simulink model "Intergration_simu"  (R2018b)
settings: Solver=FixedStepDiscrete  StartTime=0.0  StopTime=14  FixedStep=0.005  RelTol=1e-3
PostLoadFcn:
  | if any(exist('dsrtsu_mdlpostloadfcn', 'file') ~= 0), dsrtsu_mdlpostloadfcn('Execute', bdroot); end
values from neighbouring files (symbols this model uses):
  P_x165_On = 1.0    [CAN_Tx.sldd]
  P_x242_On = 1.0    [CAN_Tx.sldd]
  P_x246_On = 1.0    [CAN_Tx.sldd]
libraries: rtican x112, simulink x59
(part 2 of 31)

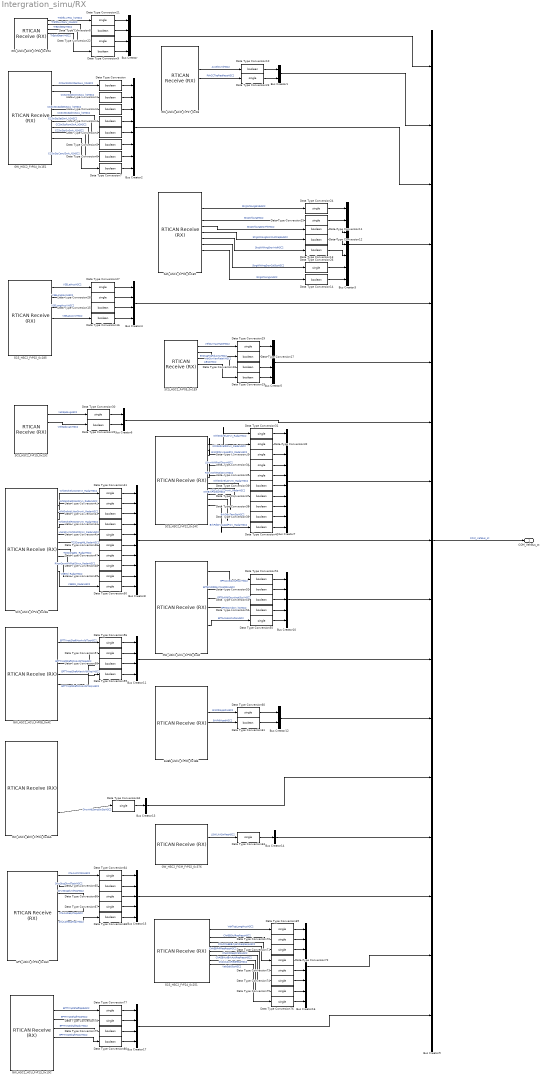
== system Intergration_simu/RX ==
  Bus Creator : BusCreator  Inputs=4  OutDataTypeStr=Bus: x194  NonVirtualBus=on
      settings: InheritFromInputs=off
  Bus Creator1 : BusCreator  Inputs=2  OutDataTypeStr=Bus: xFB  NonVirtualBus=on
      settings: InheritFromInputs=off
  Bus Creator10 : BusCreator  Inputs=5  OutDataTypeStr=Bus: xAF  NonVirtualBus=on
      settings: InheritFromInputs=off
  Bus Creator11 : BusCreator  Inputs=4  OutDataTypeStr=Bus: xAC  NonVirtualBus=on
      settings: InheritFromInputs=off
  Bus Creator12 : BusCreator  Inputs=2  OutDataTypeStr=Bus: x1B6  NonVirtualBus=on
      settings: InheritFromInputs=off
  Bus Creator13 : BusCreator  Inputs=1  OutDataTypeStr=Bus: x46A  NonVirtualBus=on
      settings: InheritFromInputs=off
  Bus Creator14 : BusCreator  Inputs=1  OutDataTypeStr=Bus: x376  NonVirtualBus=on
      settings: InheritFromInputs=off
  Bus Creator15 : BusCreator  Inputs=5  OutDataTypeStr=Bus: x1EC  NonVirtualBus=on
      settings: InheritFromInputs=off
  Bus Creator16 : BusCreator  Inputs=8  OutDataTypeStr=Bus: x251  NonVirtualBus=on
      settings: InheritFromInputs=off
  Bus Creator17 : BusCreator  Inputs=4  OutDataTypeStr=Bus: x19C  NonVirtualBus=on
      settings: InheritFromInputs=off
  Bus Creator2 : BusCreator  Inputs=8  OutDataTypeStr=Bus: x1E1  NonVirtualBus=on
      settings: InheritFromInputs=off
  Bus Creator3 : BusCreator  Inputs=7  OutDataTypeStr=Bus: x1E5  NonVirtualBus=on
      settings: InheritFromInputs=off
  Bus Creator4 : BusCreator  Inputs=4  OutDataTypeStr=Bus: x185  NonVirtualBus=on
      settings: InheritFromInputs=off
  Bus Creator5 : BusCreator  Inputs=4  OutDataTypeStr=Bus: x1E9  NonVirtualBus=on
      settings: InheritFromInputs=off
  Bus Creator6 : BusCreator  Inputs=2  OutDataTypeStr=Bus: x23C  NonVirtualBus=on
      settings: InheritFromInputs=off
  Bus Creator7 : BusCreator  Inputs=10  OutDataTypeStr=Bus: x24C  NonVirtualBus=on
      settings: InheritFromInputs=off
  Bus Creator8 : BusCreator  Inputs=10  OutDataTypeStr=Bus: x24E  NonVirtualBus=on
      settings: InheritFromInputs=off
  Bus Creator9 : BusCreator  Inputs=17  OutDataTypeStr=Bus: COM_VEHBUS_ST  NonVirtualBus=on
      settings: InheritFromInputs=off
  Data Type Conversion{,1..20,36..40,43..44,51..54,58..59,61,65,68,79..80} (39 alike) : DataTypeConversion  OutDataTypeStr=boolean
  Data Type Conversion{21..35,41..42,45..50,55..57,60,62..64,66..67,69..78} (42 alike) : DataTypeConversion  OutDataTypeStr=single
  EHBS_HSC2_FrP00_0x1B6 : rtican/RTICAN Receive (RX)   Reserved1=[]  Reserved2=[]  Reserved3=[]  Reserved4=[]  SfcnMessage=[]  Msg_Struct=[]  BoardTypeNo=[]  BoardNo=[]  ChannelNo=[]  Parameters=[]  DialogFcn=[]  UnitName=[]  Revision=[]  UnitValues=[]  DSProperties=struct('RTI',struct('Version',uint32(5),'BlockType',struct('isSLSource',uint8(1),'isSLSink',uint8(1),'isHWSource',uint8(0),'isHWSink',uint8(0),'isSetup',uint8(0),'isInline',uint8(1),'isNonInline',uint8(0),'isInterrupt',uint8(0),'isChannelwise',uint8(0)),'IOBoardType','RTICAN','UnitType','MESSAGE','Identifier','RX','DialogType','MSVC','BlockSet','RTICAN','SlaveProcessor','CAN'))  RTIBlockInterface=struct('OutputPortsWidth',int32([1 1 1 1 1 1 1]),'OutputPortsActive',[1 1 1 1 1 1 1],'OutputPortsName',{{'BrkPdlAppdChksmHSC2','BrkPdlAppdRCHSC2','BrkPdlAppdVHSC2','BrkPdlAppdHSC2',['RX status'],['RX time'],['RX delta time']}},'OutputPortsDataType',{{'SS_DOUBLE','SS_DOUBLE','SS_DOUBLE','SS_DOUBLE','SS_DOUBLE','SS_DOUBLE','SS_DOUBLE'}},'OutputPortsLabel',{{'BrkPdlAppdChksmHSC2','BrkPdlAppdRCHSC2','BrkPdlAppdVHSC2','BrkPdlAppdHSC2','','',''}},'OutputPortsLabelMode','ON','InputPortsWidth',int32(0),'InputPortsActive',0,'DialogFcn','rtican_message_interface_gui','BlockDisplay',{{'','center'}},'IconTransparency','on','ParameterTunableNames',{{}},'InitLevel',3,'BlockName',struct('Token',{{'EHBS_HSC2_FrP00'}}),'SampleTime',{{-1}},'TriggerPort',{{'none'}},'EnablePort',{{'none'}})  RTIBlockParameters=struct('BoardTypeNo',{{1,'OFF',[]}},'BoardNo',{{1,'ON',[1 16]}},'ChannelNo',{{1,'ON',[1 2]}},'Parameters',{{struct('DataFileSupport',struct('DataFileSelectedMaster',1,'DataFileSelectedLocal',1,'DataFileName','c:\users\linqi\desktop\matlab\acc\dbc\ep21_dbc\171114-lh1-ep21_ep2_fdr-_v07_acc.dbc|','DataFileDate',['24-11月-2020 15:06:17'],'SelectedFile','..\..\dbc\ep21_dbc\171114-lh1-ep21_ep2_fdr-_v07_acc.dbc','InterfaceFcn','rtican_dbc_file_parser'),'Options',struct('StatusSelected',1,'TimeSelected',1,'DeltaTimeSelected',1,'BytePortSelected',0,'MessageLengthSelected',0,'TriggerPort',struct('Selected',0,'TriggerType',0),'UserCoding',struct('Selected',0,'InterfaceFile','UserDecodingFile','FcnName','UserDecodeFcn','InportSelected',0,'InportWidth',1,'OutportSelected',0,'OutportWidth',1),'EnablePortSelected',0,'SignalOnPortnameSelected',1,'UseRXService',0),'Message',struct('MsgOnBlocknameSelected',1,'MsgName','EHBS_HSC2_FrP00','MsgIdFormat',0,'MsgId',438,'MsgLength',8,'NumSignals',4,'SampleTime',-1,'Signal',struct('SgnName',{'BrkPdlAppdChksmHSC2','BrkPdlAppdRCHSC2','BrkPdlAppdVHSC2','BrkPdlAppdHSC2'},'SgnStartBit',{0,8,48,50},'SgnLength',{8,4,2,1},'ByteLayout',{2,2,2,2},'Factor',{1,1,1,1},'Offset',{0,0,0,0},'SgnComment',{'','','',''},'SgnUnit',{'','','',''},'Min',{0,0,0,0},'Max',{255,15,3,1},'SgnType',{0,0,0,0},'SLDataType',{'SS_DOUBLE','SS_DOUBLE','SS_DOUBLE','SS_DOUBLE'},'DataType',{0,0,0,0},'ModeValue',{-1,-1,-1,-1}),'MsgIdNumFormat',0,'MsgComment',{{''}}),'Version',1.2,'general',struct('isFromLib',0)),'OFF',[]}},'GroupId',{{struct('Group',{{'RTICAN'}},'No',1,'Behavior',{{'NAMECHANGE'}},'BlockType',{{'SINK'}},'NameChangeFlag',0),'OFF',[]}},'SFcnRTICANMessage',{{struct('MsgType','RX','SFcnPortType','Scalar','MsgName','EHBS_HSC2_FrP00','MsgIdFormat','STD','MsgId',438,'MsgLength',8,'NumSignals',4,'SampleTime',-1,'Signal',struct('SgnName',{'BrkPdlAppdChksmHSC2','BrkPdlAppdRCHSC2','BrkPdlAppdVHSC2','BrkPdlAppdHSC2'},'SgnStartBit',{0,8,48,50},'SgnLength',{8,4,2,1},'ByteLayout',{['motorola back.'],['motorola back.'],['motorola back.'],['motorola back.']},'Factor',{1,1,1,1},'Offset',{0,0,0,0},'SgnType',{'standard','standard','standard','standard'},'SLDataType',{'SS_DOUBLE','SS_DOUBLE','SS_DOUBLE','SS_DOUBLE'},'DataType',{['unsigned int'],['unsigned int'],['unsigned int'],['unsigned int']},'ModeValue',{-1,-1,-1,-1}),'StatusSelected','yes','TimeSelected','yes','DeltaTimeSelected','yes','BytePortSelected','no','MessageLengthSelected','no','TriggerPort',struct('Selected','no','TriggerType',0),'UserCoding',struct('Selected','no','InterfaceFile','UserDecodingFile','FcnName','UserDecodeFcn','InportSelected','no','InportWidth',1,'OutportSelected','no','OutportWidth',1),'EnablePortSelected','no','UseRXService','no','BoardType','DS1','BoardNo',1,'ControllerNo',1),'OFF',[]}},'TLCFileName',{{'rtican_rx_message','OFF',[]}})  RTISFcnParameters=struct('SFcnRTICANMessage','struct','TLCFileName','char')  RTIBlockParaDefault=struct('BoardTypeNo',4302,'BoardNo',1,'ChannelNo',1,'Parameters',struct('DataFileSupport',struct('DataFileSelectedMaster',0,'DataFileSelectedLocal',0,'DataFileName','','DataFileDate','','SelectedFile',['<no file selected>']),'Options',struct('StatusSelected',1,'TimeSelected',1,'DeltaTimeSelected',1,'BytePortSelected',0,'MessageLengthSelected',0,'TriggerPort',struct('Selected',0,'TriggerType','rising'),'UserCoding',struct('Selected',0,'InterfaceFile','UserDecodingFile','FcnName','UserDecodeFcn','InportSelected',0,'InportWidth',1,'OutportSelected',0,'OutportWidth',1),'EnablePortSelected',0,'SignalOnPortnameSelected',1,'UseRXService',0),'Message',struct('MsgOnBlocknameSelected',0,'MsgName',['RX Message'],'MsgIdFormat',0,'MsgId',100,'MsgLength',8,'NumSignals',1,'SampleTime',-1,'Signal',struct('SgnName',['RX signal'],'SgnStartBit',0,'SgnLength',8,'SgnType',0,'ModeValue',-1,'DataType',0,'SLDataType','SS_DOUBLE','ByteLayout',0,'Factor',1,'Offset',0,'Min',0,'Max',255,'SgnComment',{{}},'SgnUnit',''),'MsgIdNumFormat',0,'MsgComment',{{''}}),'Version',1.2,'general',struct('isFromLib',1)),'GroupId',struct('Group',{{'RTICAN'}},'No',1,'Behavior',{{'NAMECHANGE'}},'BlockType',{{'SINK'}},'NameChangeFlag',0),'SFcnRTICANMessage',struct('MsgType','RX','MsgName',['RX Message'],'MsgIdFormat','STD','MsgId',100,'MsgLength',8,'NumSignals',1,'SampleTime',-1,'Signal',struct('SgnName',['RX signal'],'SgnStartBit',0,'SgnLength',8,'SgnType','standard','ModeValue',-1,'DataType',['unsigned int'],'ByteLayout',['little endian'],'SLDataType','SS_DOUBLE','Factor',1,'Offset',0),'StatusSelected','yes','TimeSelected','yes','DeltaTimeSelected','yes','BytePortSelected','no','MessageLengthSelected','no','EnablePortSelected','no','UserCoding',struct('Selected','no','InterfaceFile','UserDecodingFile','FcnName','UserDecodeFcn','InportSelected','no','InportWidth',1,'OutportSelected','no','OutportWidth',1),'TriggerPort',struct('Selected','no','TriggerType','rising'),'UseRXService','no','BoardType','DS4302','BoardNo',1,'ControllerNo',1,'SFcnPortType','Scalar'),'TLCFileName','rtican_rx_message')
      settings: AttributesFormatString=Group Id: RTICAN1\n  SourceProductName=dSPACE RTI CAN Blockset
  EPS_HSC2_FrP03_0x1EC : rtican/RTICAN Receive (RX)   Reserved1=[]  Reserved2=[]  Reserved3=[]  Reserved4=[]  SfcnMessage=[]  Msg_Struct=[]  BoardTypeNo=[]  BoardNo=[]  ChannelNo=[]  Parameters=[]  DialogFcn=[]  UnitName=[]  Revision=[]  UnitValues=[]  DSProperties=struct('RTI',struct('Version',uint32(5),'BlockType',struct('isSLSource',uint8(1),'isSLSink',uint8(1),'isHWSource',uint8(0),'isHWSink',uint8(0),'isSetup',uint8(0),'isInline',uint8(1),'isNonInline',uint8(0),'isInterrupt',uint8(0),'isChannelwise',uint8(0)),'IOBoardType','RTICAN','UnitType','MESSAGE','Identifier','RX','DialogType','MSVC','BlockSet','RTICAN','SlaveProcessor','CAN'))  RTIBlockInterface=struct('OutputPortsWidth',int32([1 1 1 1 1 1 1 1 1 1]),'OutputPortsActive',[1 1 1 1 1 1 1 1 1 1],'OutputPortsName',{{'ChLKACtrlStsHSC2','DrvrStrgDlvrdToqVHSC2','DrvrStrgDlvrdToqHSC2','ChLKARespToqPVHSC2','ChLKARespToqHSC2','ChLKARespToqVHSC2','ChLKAAlvRCHSC2',['RX status'],['RX time'],['RX delta time']}},'OutputPortsDataType',{{'SS_DOUBLE','SS_DOUBLE','SS_DOUBLE','SS_DOUBLE','SS_DOUBLE','SS_DOUBLE','SS_DOUBLE','SS_DOUBLE','SS_DOUBLE','SS_DOUBLE'}},'OutputPortsLabel',{{'ChLKACtrlStsHSC2','DrvrStrgDlvrdToqVHSC2','DrvrStrgDlvrdToqHSC2','ChLKARespToqPVHSC2','ChLKARespToqHSC2','ChLKARespToqVHSC2','ChLKAAlvRCHSC2','','',''}},'OutputPortsLabelMode','ON','InputPortsWidth',int32(0),'InputPortsActive',0,'DialogFcn','rtican_message_interface_gui','BlockDisplay',{{'','center'}},'IconTransparency','on','ParameterTunableNames',{{}},'InitLevel',3,'BlockName',struct('Token',{{'EPS_HSC2_FrP03'}}),'SampleTime',{{-1}},'TriggerPort',{{'none'}},'EnablePort',{{'none'}})  RTIBlockParameters=struct('BoardTypeNo',{{1,'OFF',[]}},'BoardNo',{{1,'ON',[1 16]}},'ChannelNo',{{1,'ON',[1 2]}},'Parameters',{{struct('DataFileSupport',struct('DataFileSelectedMaster',1,'DataFileSelectedLocal',1,'DataFileName','c:\users\linqi\desktop\matlab\acc\dbc\ep21_dbc\171114-lh1-ep21_ep2_fdr-_v07_acc.dbc|c:\users\linqi\desktop\matlab\acc\dbc\ep21_dbc\171120-lh1-ep21_ep2_fvcm-_v07_lka.dbc|','DataFileDate',{{{['24-11月-2020 15:06:17']},{['24-11月-2020 15:35:27']}}},'SelectedFile','..\..\dbc\ep21_dbc\171120-lh1-ep21_ep2_fvcm-_v07_lka.dbc','InterfaceFcn','rtican_dbc_file_parser'),'Options',struct('StatusSelected',1,'TimeSelected',1,'DeltaTimeSelected',1,'BytePortSelected',0,'MessageLengthSelected',0,'TriggerPort',struct('Selected',0,'TriggerType',0),'UserCoding',struct('Selected',0,'InterfaceFile','UserDecodingFile','FcnName','UserDecodeFcn','InportSelected',0,'InportWidth',1,'OutportSelected',0,'OutportWidth',1),'EnablePortSelected',0,'SignalOnPortnameSelected',1,'UseRXService',0),'Message',struct('MsgOnBlocknameSelected',1,'MsgName','EPS_HSC2_FrP03','MsgIdFormat',0,'MsgId',492,'MsgLength',8,'NumSignals',7,'SampleTime',-1,'Signal',struct('SgnName',{'ChLKACtrlStsHSC2','DrvrStrgDlvrdToqVHSC2','DrvrStrgDlvrdToqHSC2','ChLKARespToqPVHSC2','ChLKARespToqHSC2','ChLKARespToqVHSC2','ChLKAAlvRCHSC2'},'SgnStartBit',{12,15,16,32,48,59,60},'SgnLength',{3,1,11,15,11,1,4},'SgnType',{0,0,0,0,0,0,0},'ModeValue',{-1,-1,-1,-1,-1,-1,-1},'DataType',{0,0,0,0,0,0,0},'ByteLayout',{2,2,2,2,2,2,2},'Factor',{1,1,0.01,1,0.01,1,1},'Offset',{0,0,-10.24,0,-10.24,0,0},'SgnComment',{{''},{''},{''},{''},{''},{''},{''}},'SgnUnit',{'','','Nm','','Nm','',''},'Min',{0,0,-10.24,0,-10.24,0,0},'Max',{7,1,10.23,32767,10.23,1,15},'SLDataType',{'SS_DOUBLE','SS_DOUBLE','SS_DOUBLE','SS_DOUBLE','SS_DOUBLE','SS_DOUBLE','SS_DOUBLE'}),'MsgIdNumFormat',1,'MsgComment',{{''}}),'Version',1.2,'general',struct('isFromLib',0)),'OFF',[]}},'GroupId',{{struct('Group',{{'RTICAN'}},'No',1,'Behavior',{{'NAMECHANGE'}},'BlockType',{{'SINK'}},'NameChangeFlag',0),'OFF',[]}},'SFcnRTICANMessage',{{struct('MsgType','RX','SFcnPortType','Scalar','MsgName','EPS_HSC2_FrP03','MsgIdFormat','STD','MsgId',492,'MsgLength',8,'NumSignals',7,'SampleTime',-1,'Signal',struct('SgnName',{'ChLKACtrlStsHSC2','DrvrStrgDlvrdToqVHSC2','DrvrStrgDlvrdToqHSC2','ChLKARespToqPVHSC2','ChLKARespToqHSC2','ChLKARespToqVHSC2','ChLKAAlvRCHSC2'},'SgnStartBit',{12,15,16,32,48,59,60},'SgnLength',{3,1,11,15,11,1,4},'SgnType',{'standard','standard','standard','standard','standard','standard','standard'},'ModeValue',{-1,-1,-1,-1,-1,-1,-1},'DataType',{['unsigned int'],['unsigned int'],['unsigned int'],['unsigned int'],['unsigned int'],['unsigned int'],['unsigned int']},'ByteLayout',{['motorola back.'],['motorola back.'],['motorola back.'],['motorola back.'],['motorola back.'],['motorola back.'],['motorola back.']},'Factor',{1,1,0.01,1,0.01,1,1},'Offset',{0,0,-10.24,0,-10.24,0,0},'SLDataType',{'SS_DOUBLE','SS_DOUBLE','SS_DOUBLE','SS_DOUBLE','SS_DOUBLE','SS_DOUBLE','SS_DOUBLE'}),'StatusSelected','yes','TimeSelected','yes','DeltaTimeSelected','yes','BytePortSelected','no','MessageLengthSelected','no','TriggerPort',struct('Selected','no','TriggerType',0),'UserCoding',struct('Selected','no','InterfaceFile','UserDecodingFile','FcnName','UserDecodeFcn','InportSelected','no','InportWidth',1,'OutportSelected','no','OutportWidth',1),'EnablePortSelected','no','UseRXService','no','BoardType','DS1','BoardNo',1,'ControllerNo',1),'OFF',[]}},'TLCFileName',{{'rtican_rx_message','OFF',[]}})  RTISFcnParameters=struct('SFcnRTICANMessage','struct','TLCFileName','char')  RTIBlockParaDefault=struct('BoardTypeNo',4302,'BoardNo',1,'ChannelNo',1,'Parameters',struct('DataFileSupport',struct('DataFileSelectedMaster',0,'DataFileSelectedLocal',0,'DataFileName','','DataFileDate','','SelectedFile',['<no file selected>']),'Options',struct('StatusSelected',1,'TimeSelected',1,'DeltaTimeSelected',1,'BytePortSelected',0,'MessageLengthSelected',0,'TriggerPort',struct('Selected',0,'TriggerType','rising'),'UserCoding',struct('Selected',0,'InterfaceFile','UserDecodingFile','FcnName','UserDecodeFcn','InportSelected',0,'InportWidth',1,'OutportSelected',0,'OutportWidth',1),'EnablePortSelected',0,'SignalOnPortnameSelected',1,'UseRXService',0),'Message',struct('MsgOnBlocknameSelected',0,'MsgName',['RX Message'],'MsgIdFormat',0,'MsgId',100,'MsgLength',8,'NumSignals',1,'SampleTime',-1,'Signal',struct('SgnName',['RX signal'],'SgnStartBit',0,'SgnLength',8,'SgnType',0,'ModeValue',-1,'DataType',0,'SLDataType','SS_DOUBLE','ByteLayout',0,'Factor',1,'Offset',0,'Min',0,'Max',255,'SgnComment',{{}},'SgnUnit',''),'MsgIdNumFormat',0,'MsgComment',{{''}}),'Version',1.2,'general',struct('isFromLib',1)),'GroupId',struct('Group',{{'RTICAN'}},'No',1,'Behavior',{{'NAMECHANGE'}},'BlockType',{{'SINK'}},'NameChangeFlag',0),'SFcnRTICANMessage',struct('MsgType','RX','MsgName',['RX Message'],'MsgIdFormat','STD','MsgId',100,'MsgLength',8,'NumSignals',1,'SampleTime',-1,'Signal',struct('SgnName',['RX signal'],'SgnStartBit',0,'SgnLength',8,'SgnType','standard','ModeValue',-1,'DataType',['unsigned int'],'ByteLayout',['little endian'],'SLDataType','SS_DOUBLE','Factor',1,'Offset',0),'StatusSelected','yes','TimeSelected','yes','DeltaTimeSelected','yes','BytePortSelected','no','MessageLengthSelected','no','EnablePortSelected','no','UserCoding',struct('Selected','no','InterfaceFile','UserDecodingFile','FcnName','UserDecodeFcn','InportSelected','no','InportWidth',1,'OutportSelected','no','OutportWidth',1),'TriggerPort',struct('Selected','no','TriggerType','rising'),'UseRXService','no','BoardType','DS4302','BoardNo',1,'ControllerNo',1,'SFcnPortType','Scalar'),'TLCFileName','rtican_rx_message')
      settings: AttributesFormatString=Group Id: RTICAN1\n  SourceProductName=dSPACE RTI CAN Blockset
  GW_HSC2_BCM_FrP04_0x46A : rtican/RTICAN Receive (RX)   Reserved1=[]  Reserved2=[]  Reserved3=[]  Reserved4=[]  SfcnMessage=[]  Msg_Struct=[]  BoardTypeNo=[]  BoardNo=[]  ChannelNo=[]  Parameters=[]  DialogFcn=[]  UnitName=[]  Revision=[]  UnitValues=[]  DSProperties=struct('RTI',struct('Version',uint32(5),'BlockType',struct('isSLSource',uint8(1),'isSLSink',uint8(1),'isHWSource',uint8(0),'isHWSink',uint8(0),'isSetup',uint8(0),'isInline',uint8(1),'isNonInline',uint8(0),'isInterrupt',uint8(0),'isChannelwise',uint8(0)),'IOBoardType','RTICAN','UnitType','MESSAGE','Identifier','RX','DialogType','MSVC','BlockSet','RTICAN','SlaveProcessor','CAN'))  RTIBlockInterface=struct('OutputPortsWidth',int32([1 1 1 1 1 1 1 1 1 1 1 1 1 1 1 1 1 1 1 1 1 1 1]),'OutputPortsActive',ones(1,23),'OutputPortsName',{{'VehSideLghtStsHSC2','RDircnIndLghtFHSC2','KeyDetIndxHSC2','FrtWiperParkPosAHSC2','FrtWshrPumpAHSC2','RLDoorOpenStsHSC2','FrtPsngDoorOpenStsHSC2','DspMeasSysHSC2','BntOpenStsHSC2','RrFogLghtOnHSC2','RDircnIOHSC2','LDircnIndLghtFHSC2','LDircnIOHSC2','DipdBeamLghtOnHSC2','FrtFogLghtOnHSC2','MainBeamLghtOnHSC2','DrvrDoorOpenStsHSC2','DircnIndLampSwStsHSC2','RRDoorOpenStsHSC2','LdspcOpenStsHSC2',['RX status'],['RX time'],['RX delta time']}},'OutputPortsDataType',{{'SS_DOUBLE','SS_DOUBLE','SS_DOUBLE','SS_DOUBLE','SS_DOUBLE','SS_DOUBLE','SS_DOUBLE','SS_DOUBLE','SS_DOUBLE','SS_DOUBLE','SS_DOUBLE','SS_DOUBLE','SS_DOUBLE','SS_DOUBLE','SS_DOUBLE','SS_DOUBLE','SS_DOUBLE','SS_DOUBLE','SS_DOUBLE','SS_DOUBLE','SS_DOUBLE','SS_DOUBLE','SS_DOUBLE'}},'OutputPortsLabel',{{'VehSideLghtStsHSC2','RDircnIndLghtFHSC2','KeyDetIndxHSC2','FrtWiperParkPosAHSC2','FrtWshrPumpAHSC2','RLDoorOpenStsHSC2','FrtPsngDoorOpenStsHSC2','DspMeasSysHSC2','BntOpenStsHSC2','RrFogLghtOnHSC2','RDircnIOHSC2','LDircnIndLghtFHSC2','LDircnIOHSC2','DipdBeamLghtOnHSC2','FrtFogLghtOnHSC2','MainBeamLghtOnHSC2','DrvrDoorOpenStsHSC2','DircnIndLampSwStsHSC2','RRDoorOpenStsHSC2','LdspcOpenStsHSC2','','',''}},'OutputPortsLabelMode','ON','InputPortsWidth',int32(0),'InputPortsActive',0,'DialogFcn','rtican_message_interface_gui','BlockDisplay',{{'','center'}},'IconTransparency','on','ParameterTunableNames',{{}},'InitLevel',3,'BlockName',struct('Token',{{'GW_HSC2_BCM_FrP04'}}),'SampleTime',{{-1}},'TriggerPort',{{'none'}},'EnablePort',{{'none'}})  RTIBlockParameters=struct('BoardTypeNo',{{1,'OFF',[]}},'BoardNo',{{1,'ON',[1 16]}},'ChannelNo',{{1,'ON',[1 2]}},'Parameters',{{struct('DataFileSupport',struct('DataFileSelectedMaster',1,'DataFileSelectedLocal',1,'DataFileName','c:\users\linqi\desktop\matlab\acc\dbc\ep21_dbc\171114-lh1-ep21_ep2_fdr-_v07_acc.dbc|','DataFileDate',{{{['24-11月-2020 15:06:17']}}},'SelectedFile','..\..\dbc\ep21_dbc\171114-lh1-ep21_ep2_fdr-_v07_acc.dbc','InterfaceFcn','rtican_dbc_file_parser'),'Options',struct('StatusSelected',1,'TimeSelected',1,'DeltaTimeSelected',1,'BytePortSelected',0,'MessageLengthSelected',0,'TriggerPort',struct('Selected',0,'TriggerType',0),'UserCoding',struct('Selected',0,'InterfaceFile','UserDecodingFile','FcnName','UserDecodeFcn','InportSelected',0,'InportWidth',1,'OutportSelected',0,'OutportWidth',1),'EnablePortSelected',0,'SignalOnPortnameSelected',1,'UseRXService',0),'Message',struct('MsgOnBlocknameSelected',1,'MsgName','GW_HSC2_BCM_FrP04','MsgIdFormat',0,'MsgId',1130,'MsgLength',8,'NumSignals',20,'SampleTime',-1,'Signal',struct('SgnName',{'VehSideLghtStsHSC2','RDircnIndLghtFHSC2','KeyDetIndxHSC2','FrtWiperParkPosAHSC2','FrtWshrPumpAHSC2','RLDoorOpenStsHSC2','FrtPsngDoorOpenStsHSC2','DspMeasSysHSC2','BntOpenStsHSC2','RrFogLghtOnHSC2','RDircnIOHSC2','LDircnIndLghtFHSC2','LDircnIOHSC2','DipdBeamLghtOnHSC2','FrtFogLghtOnHSC2','MainBeamLghtOnHSC2','DrvrDoorOpenStsHSC2','DircnIndLampSwStsHSC2','RRDoorOpenStsHSC2','LdspcOpenStsHSC2'},'SgnStartBit',{0,8,9,12,15,16,18,20,22,48,49,50,51,53,54,55,56,58,60,62},'SgnLength',{2,1,3,1,1,2,2,1,2,1,1,1,1,1,1,1,2,2,2,2},'SgnType',{0,0,0,0,0,0,0,0,0,0,0,0,0,0,0,0,0,0,0,0},'ModeValue',{-1,-1,-1,-1,-1,-1,-1,-1,-1,-1,-1,-1,-1,-1,-1,-1,-1,-1,-1,-1},'DataType',{0,0,0,0,0,0,0,0,0,0,0,0,0,0,0,0,0,0,0,0},'ByteLayout',{2,2,2,2,2,2,2,2,2,2,2,2,2,2,2,2,2,2,2,2},'Factor',{1,1,1,1,1,1,1,1,1,1,1,1,1,1,1,1,1,1,1,1},'Offset',{0,0,0,0,0,0,0,0,0,0,0,0,0,0,0,0,0,0,0,0},'SgnComment',{{''},{''},{''},{['Front Wiper Park Position Active' char(10) 'Wiper Park Position for the Front wiper']},{['Front Washer Pump Active']},{''},{''},{''},{''},{''},{''},{''},{''},{''},{''},{''},{''},{''},{['Rear Right Door Open Status']},{''}},'SgnUnit',{'','','','','','','','','','','','','','','','','','','',''},'Min',{0,0,0,0,0,0,0,0,0,0,0,0,0,0,0,0,0,0,0,0},'Max',{3,1,7,1,1,3,3,1,3,1,1,1,1,1,1,1,3,3,3,3},'SLDataType',{'SS_DOUBLE','SS_DOUBLE','SS_DOUBLE','SS_DOUBLE','SS_DOUBLE','SS_DOUBLE','SS_DOUBLE','SS_DOUBLE','SS_DOUBLE','SS_DOUBLE','SS_DOUBLE','SS_DOUBLE','SS_DOUBLE','SS_DOUBLE','SS_DOUBLE','SS_DOUBLE','SS_DOUBLE','SS_DOUBLE','SS_DOUBLE','SS_DOUBLE'}),'MsgIdNumFormat',1,'MsgComment',{{''}}),'Version',1.2,'general',struct('isFromLib',0)),'OFF',[]}},'GroupId',{{struct('Group',{{'RTICAN'}},'No',1,'Behavior',{{'NAMECHANGE'}},'BlockType',{{'SINK'}},'NameChangeFlag',0),'OFF',[]}},'SFcnRTICANMessage',{{struct('MsgType','RX','SFcnPortType','Scalar','MsgName','GW_HSC2_BCM_FrP04','MsgIdFormat','STD','MsgId',1130,'MsgLength',8,'NumSignals',20,'SampleTime',-1,'Signal',struct('SgnName',{'VehSideLghtStsHSC2','RDircnIndLghtFHSC2','KeyDetIndxHSC2','FrtWiperParkPosAHSC2','FrtWshrPumpAHSC2','RLDoorOpenStsHSC2','FrtPsngDoorOpenStsHSC2','DspMeasSysHSC2','BntOpenStsHSC2','RrFogLghtOnHSC2','RDircnIOHSC2','LDircnIndLghtFHSC2','LDircnIOHSC2','DipdBeamLghtOnHSC2','FrtFogLghtOnHSC2','MainBeamLghtOnHSC2','DrvrDoorOpenStsHSC2','DircnIndLampSwStsHSC2','RRDoorOpenStsHSC2','LdspcOpenStsHSC2'},'SgnStartBit',{0,8,9,12,15,16,18,20,22,48,49,50,51,53,54,55,56,58,60,62},'SgnLength',{2,1,3,1,1,2,2,1,2,1,1,1,1,1,1,1,2,2,2,2},'SgnType',{'standard','standard','standard','standard','standard','standard','standard','standard','standard','standard','standard','standard','standard','standard','standard','standard','standard','standard','standard','standard'},'ModeValue',{-1,-1,-1,-1,-1,-1,-1,-1,-1,-1,-1,-1,-1,-1,-1,-1,-1,-1,-1,-1},'DataType',{['unsigned int'],['unsigned int'],['unsigned int'],['unsigned int'],['unsigned int'],['unsigned int'],['unsigned int'],['unsigned int'],['unsigned int'],['unsigned int'],['unsigned int'],['unsigned int'],['unsigned int'],['unsigned int'],['unsigned int'],['unsigned int'],['unsigned int'],['unsigned int'],['unsigned int'],['unsigned int']},'ByteLayout',{['motorola back.'],['motorola back.'],['motorola back.'],['motorola back.'],['motorola back.'],['motorola back.'],['motorola back.'],['motorola back.'],['motorola back.'],['motorola back.'],['motorola back.'],['motorola back.'],['motorola back.'],['motorola back.'],['motorola back.'],['motorola back.'],['motorola back.'],['motorola back.'],['motorola back.'],['motorola back.']},'Factor',{1,1,1,1,1,1,1,1,1,1,1,1,1,1,1,1,1,1,1,1},'Offset',{0,0,0,0,0,0,0,0,0,0,0,0,0,0,0,0,0,0,0,0},'SLDataType',{'SS_DOUBLE','SS_DOUBLE','SS_DOUBLE','SS_DOUBLE','SS_DOUBLE','SS_DOUBLE','SS_DOUBLE','SS_DOUBLE','SS_DOUBLE','SS_DOUBLE','SS_DOUBLE','SS_DOUBLE','SS_DOUBLE','SS_DOUBLE','SS_DOUBLE','SS_DOUBLE','SS_DOUBLE','SS_DOUBLE','SS_DOUBLE','SS_DOUBLE'}),'StatusSelected','yes','TimeSelected','yes','DeltaTimeSelected','yes','BytePortSelected','no','MessageLengthSelected','no','TriggerPort',struct('Selected','no','TriggerType',0),'UserCoding',struct('Selected','no','InterfaceFile','UserDecodingFile','FcnName','UserDecodeFcn','InportSelected','no','InportWidth',1,'OutportSelected','no','OutportWidth',1),'EnablePortSelected','no','UseRXService','no','BoardType','DS1','BoardNo',1,'ControllerNo',1),'OFF',[]}},'TLCFileName',{{'rtican_rx_message','OFF',[]}})  RTISFcnParameters=struct('SFcnRTICANMessage','struct','TLCFileName','char')  RTIBlockParaDefault=struct('BoardTypeNo',4302,'BoardNo',1,'ChannelNo',1,'Parameters',struct('DataFileSupport',struct('DataFileSelectedMaster',0,'DataFileSelectedLocal',0,'DataFileName','','DataFileDate','','SelectedFile',['<no file selected>']),'Options',struct('StatusSelected',1,'TimeSelected',1,'DeltaTimeSelected',1,'BytePortSelected',0,'MessageLengthSelected',0,'TriggerPort',struct('Selected',0,'TriggerType','rising'),'UserCoding',struct('Selected',0,'InterfaceFile','UserDecodingFile','FcnName','UserDecodeFcn','InportSelected',0,'InportWidth',1,'OutportSelected',0,'OutportWidth',1),'EnablePortSelected',0,'SignalOnPortnameSelected',1,'UseRXService',0),'Message',struct('MsgOnBlocknameSelected',0,'MsgName',['RX Message'],'MsgIdFormat',0,'MsgId',100,'MsgLength',8,'NumSignals',1,'SampleTime',-1,'Signal',struct('SgnName',['RX signal'],'SgnStartBit',0,'SgnLength',8,'SgnType',0,'ModeValue',-1,'DataType',0,'SLDataType','SS_DOUBLE','ByteLayout',0,'Factor',1,'Offset',0,'Min',0,'Max',255,'SgnComment',{{}},'SgnUnit',''),'MsgIdNumFormat',0,'MsgComment',{{''}}),'Version',1.2,'general',struct('isFromLib',1)),'GroupId',struct('Group',{{'RTICAN'}},'No',1,'Behavior',{{'NAMECHANGE'}},'BlockType',{{'SINK'}},'NameChangeFlag',0),'SFcnRTICANMessage',struct('MsgType','RX','MsgName',['RX Message'],'MsgIdFormat','STD','MsgId',100,'MsgLength',8,'NumSignals',1,'SampleTime',-1,'Signal',struct('SgnName',['RX signal'],'SgnStartBit',0,'SgnLength',8,'SgnType','standard','ModeValue',-1,'DataType',['unsigned int'],'ByteLayout',['little endian'],'SLDataType','SS_DOUBLE','Factor',1,'Offset',0),'StatusSelected','yes','TimeSelected','yes','DeltaTimeSelected','yes','BytePortSelected','no','MessageLengthSelected','no','EnablePortSelected','no','UserCoding',struct('Selected','no','InterfaceFile','UserDecodingFile','FcnName','UserDecodeFcn','InportSelected','no','InportWidth',1,'OutportSelected','no','OutportWidth',1),'TriggerPort',struct('Selected','no','TriggerType','rising'),'UseRXService','no','BoardType','DS4302','BoardNo',1,'ControllerNo',1,'SFcnPortType','Scalar'),'TLCFileName','rtican_rx_message')
      settings: AttributesFormatString=Group Id: RTICAN1\n  SourceProductName=dSPACE RTI CAN Blockset
  GW_HSC2_ECM_FrP04_0x194 : rtican/RTICAN Receive (RX)   Reserved1=[]  Reserved2=[]  Reserved3=[]  Reserved4=[]  SfcnMessage=[]  Msg_Struct=[]  BoardTypeNo=[]  BoardNo=[]  ChannelNo=[]  Parameters=[]  DialogFcn=[]  UnitName=[]  Revision=[]  UnitValues=[]  DSProperties=struct('RTI',struct('Version',uint32(5),'BlockType',struct('isSLSource',uint8(1),'isSLSink',uint8(1),'isHWSource',uint8(0),'isHWSink',uint8(0),'isSetup',uint8(0),'isInline',uint8(1),'isNonInline',uint8(0),'isInterrupt',uint8(0),'isChannelwise',uint8(0)),'IOBoardType','RTICAN','UnitType','MESSAGE','Identifier','RX','DialogType','MSVC','BlockSet','RTICAN','SlaveProcessor','CAN'))  RTIBlockInterface=struct('OutputPortsWidth',int32([1 1 1 1 1 1 1]),'OutputPortsActive',[1 1 1 1 1 1 1],'OutputPortsName',{{'TrShftLvrPos_h1HSC2','TrShftLvrPosV_h1HSC2','TrEstdGearHSC2','TrEstdGearVHSC2',['RX status'],['RX time'],['RX delta time']}},'OutputPortsDataType',{{'SS_DOUBLE','SS_DOUBLE','SS_DOUBLE','SS_DOUBLE','SS_DOUBLE','SS_DOUBLE','SS_DOUBLE'}},'OutputPortsLabel',{{'TrShftLvrPos_h1HSC2','TrShftLvrPosV_h1HSC2','TrEstdGearHSC2','TrEstdGearVHSC2','','',''}},'OutputPortsLabelMode','ON','InputPortsWidth',int32(0),'InputPortsActive',0,'DialogFcn','rtican_message_interface_gui','BlockDisplay',{{'','center'}},'IconTransparency','on','ParameterTunableNames',{{}},'InitLevel',3,'BlockName',struct('Token',{{'GW_HSC2_ECM_FrP04'}}),'SampleTime',{{-1}},'TriggerPort',{{'none'}},'EnablePort',{{'none'}})  RTIBlockParameters=struct('BoardTypeNo',{{1,'OFF',[]}},'BoardNo',{{1,'ON',[1 16]}},'ChannelNo',{{1,'ON',[1 2]}},'Parameters',{{struct('DataFileSupport',struct('DataFileSelectedMaster',1,'DataFileSelectedLocal',1,'DataFileName','c:\users\linqi\desktop\matlab\acc\dbc\ep21_dbc\171114-lh1-ep21_ep2_fdr-_v07.dbc|','DataFileDate',['24-11月-2020 15:06:17'],'SelectedFile','..\..\dbc\ep21_dbc\171114-lh1-ep21_ep2_fdr-_v07_acc.dbc','InterfaceFcn','rtican_dbc_file_parser'),'Options',struct('StatusSelected',1,'TimeSelected',1,'DeltaTimeSelected',1,'BytePortSelected',0,'MessageLengthSelected',0,'TriggerPort',struct('Selected',0,'TriggerType',0),'UserCoding',struct('Selected',0,'InterfaceFile','UserDecodingFile','FcnName','UserDecodeFcn','InportSelected',0,'InportWidth',1,'OutportSelected',0,'OutportWidth',1),'EnablePortSelected',0,'SignalOnPortnameSelected',1,'UseRXService',0),'Message',struct('MsgOnBlocknameSelected',1,'MsgName','GW_HSC2_ECM_FrP04','MsgIdFormat',0,'MsgId',404,'MsgLength',8,'NumSignals',4,'SampleTime',-1,'Signal',struct('SgnName',{'TrShftLvrPos_h1HSC2','TrShftLvrPosV_h1HSC2','TrEstdGearHSC2','TrEstdGearVHSC2'},'SgnStartBit',{32,36,56,60},'SgnLength',{4,1,4,1},'ByteLayout',{2,2,2,2},'Factor',{1,1,1,1},'Offset',{0,0,0,0},'SgnComment',{'','','',''},'SgnUnit',{'','','',''},'Min',{0,0,0,0},'Max',{15,1,15,1},'SgnType',{0,0,0,0},'SLDataType',{'SS_DOUBLE','SS_DOUBLE','SS_DOUBLE','SS_DOUBLE'},'DataType',{0,0,0,0},'ModeValue',{-1,-1,-1,-1}),'MsgIdNumFormat',0,'MsgComment',{{''}}),'Version',1.2,'general',struct('isFromLib',0)),'OFF',[]}},'GroupId',{{struct('Group',{{'RTICAN'}},'No',1,'Behavior',{{'NAMECHANGE'}},'BlockType',{{'SINK'}},'NameChangeFlag',0),'OFF',[]}},'SFcnRTICANMessage',{{struct('MsgType','RX','SFcnPortType','Scalar','MsgName','GW_HSC2_ECM_FrP04','MsgIdFormat','STD','MsgId',404,'MsgLength',8,'NumSignals',4,'SampleTime',-1,'Signal',struct('SgnName',{'TrShftLvrPos_h1HSC2','TrShftLvrPosV_h1HSC2','TrEstdGearHSC2','TrEstdGearVHSC2'},'SgnStartBit',{32,36,56,60},'SgnLength',{4,1,4,1},'ByteLayout',{['motorola back.'],['motorola back.'],['motorola back.'],['motorola back.']},'Factor',{1,1,1,1},'Offset',{0,0,0,0},'SgnType',{'standard','standard','standard','standard'},'SLDataType',{'SS_DOUBLE','SS_DOUBLE','SS_DOUBLE','SS_DOUBLE'},'DataType',{['unsigned int'],['unsigned int'],['unsigned int'],['unsigned int']},'ModeValue',{-1,-1,-1,-1}),'StatusSelected','yes','TimeSelected','yes','DeltaTimeSelected','yes','BytePortSelected','no','MessageLengthSelected','no','TriggerPort',struct('Selected','no','TriggerType',0),'UserCoding',struct('Selected','no','InterfaceFile','UserDecodingFile','FcnName','UserDecodeFcn','InportSelected','no','InportWidth',1,'OutportSelected','no','OutportWidth',1),'EnablePortSelected','no','UseRXService','no','BoardType','DS1','BoardNo',1,'ControllerNo',1),'OFF',[]}},'TLCFileName',{{'rtican_rx_message','OFF',[]}})  RTISFcnParameters=struct('SFcnRTICANMessage','struct','TLCFileName','char')  RTIBlockParaDefault=struct('BoardTypeNo',4302,'BoardNo',1,'ChannelNo',1,'Parameters',struct('DataFileSupport',struct('DataFileSelectedMaster',0,'DataFileSelectedLocal',0,'DataFileName','','DataFileDate','','SelectedFile',['<no file selected>']),'Options',struct('StatusSelected',1,'TimeSelected',1,'DeltaTimeSelected',1,'BytePortSelected',0,'MessageLengthSelected',0,'TriggerPort',struct('Selected',0,'TriggerType','rising'),'UserCoding',struct('Selected',0,'InterfaceFile','UserDecodingFile','FcnName','UserDecodeFcn','InportSelected',0,'InportWidth',1,'OutportSelected',0,'OutportWidth',1),'EnablePortSelected',0,'SignalOnPortnameSelected',1,'UseRXService',0),'Message',struct('MsgOnBlocknameSelected',0,'MsgName',['RX Message'],'MsgIdFormat',0,'MsgId',100,'MsgLength',8,'NumSignals',1,'SampleTime',-1,'Signal',struct('SgnName',['RX signal'],'SgnStartBit',0,'SgnLength',8,'SgnType',0,'ModeValue',-1,'DataType',0,'SLDataType','SS_DOUBLE','ByteLayout',0,'Factor',1,'Offset',0,'Min',0,'Max',255,'SgnComment',{{}},'SgnUnit',''),'MsgIdNumFormat',0,'MsgComment',{{''}}),'Version',1.2,'general',struct('isFromLib',1)),'GroupId',struct('Group',{{'RTICAN'}},'No',1,'Behavior',{{'NAMECHANGE'}},'BlockType',{{'SINK'}},'NameChangeFlag',0),'SFcnRTICANMessage',struct('MsgType','RX','MsgName',['RX Message'],'MsgIdFormat','STD','MsgId',100,'MsgLength',8,'NumSignals',1,'SampleTime',-1,'Signal',struct('SgnName',['RX signal'],'SgnStartBit',0,'SgnLength',8,'SgnType','standard','ModeValue',-1,'DataType',['unsigned int'],'ByteLayout',['little endian'],'SLDataType','SS_DOUBLE','Factor',1,'Offset',0),'StatusSelected','yes','TimeSelected','yes','DeltaTimeSelected','yes','BytePortSelected','no','MessageLengthSelected','no','EnablePortSelected','no','UserCoding',struct('Selected','no','InterfaceFile','UserDecodingFile','FcnName','UserDecodeFcn','InportSelected','no','InportWidth',1,'OutportSelected','no','OutportWidth',1),'TriggerPort',struct('Selected','no','TriggerType','rising'),'UseRXService','no','BoardType','DS4302','BoardNo',1,'ControllerNo',1,'SFcnPortType','Scalar'),'TLCFileName','rtican_rx_message')
      settings: AttributesFormatString=Group Id: RTICAN1\n  SourceProductName=dSPACE RTI CAN Blockset
  GW_HSC2_ECM_FrP27_0xFB : rtican/RTICAN Receive (RX)   Reserved1=[]  Reserved2=[]  Reserved3=[]  Reserved4=[]  SfcnMessage=[]  Msg_Struct=[]  BoardTypeNo=[]  BoardNo=[]  ChannelNo=[]  Parameters=[]  DialogFcn=[]  UnitName=[]  Revision=[]  UnitValues=[]  DSProperties=struct('RTI',struct('Version',uint32(5),'BlockType',struct('isSLSource',uint8(1),'isSLSink',uint8(1),'isHWSource',uint8(0),'isHWSink',uint8(0),'isSetup',uint8(0),'isInline',uint8(1),'isNonInline',uint8(0),'isInterrupt',uint8(0),'isChannelwise',uint8(0)),'IOBoardType','RTICAN','UnitType','MESSAGE','Identifier','RX','DialogType','MSVC','BlockSet','RTICAN','SlaveProcessor','CAN'))  RTIBlockInterface=struct('OutputPortsWidth',int32([1 1 1 1 1 1 1]),'OutputPortsActive',[1 1 1 1 1 1 1],'OutputPortsName',{{'PtACCToqReqRespPVHSC2','PtADASAlvRCHSC2','AccelOvrdHSC2','PtACCToqReqRespHSC2',['RX status'],['RX time'],['RX delta time']}},'OutputPortsDataType',{{'SS_DOUBLE','SS_DOUBLE','SS_DOUBLE','SS_DOUBLE','SS_DOUBLE','SS_DOUBLE','SS_DOUBLE'}},'OutputPortsLabel',{{'PtACCToqReqRespPVHSC2','PtADASAlvRCHSC2','AccelOvrdHSC2','PtACCToqReqRespHSC2','','',''}},'OutputPortsLabelMode','ON','InputPortsWidth',int32(0),'InputPortsActive',0,'DialogFcn','rtican_message_interface_gui','BlockDisplay',{{'','center'}},'IconTransparency','on','ParameterTunableNames',{{}},'InitLevel',3,'BlockName',struct('Token',{{'GW_HSC2_ECM_FrP27'}}),'SampleTime',{{-1}},'TriggerPort',{{'none'}},'EnablePort',{{'none'}})  RTIBlockParameters=struct('BoardTypeNo',{{1,'OFF',[]}},'BoardNo',{{1,'ON',[1 16]}},'ChannelNo',{{1,'ON',[1 2]}},'Parameters',{{struct('DataFileSupport',struct('DataFileSelectedMaster',1,'DataFileSelectedLocal',1,'DataFileName','c:\users\linqi\desktop\matlab\acc\dbc\ep21_dbc\171114-lh1-ep21_ep2_fdr-_v07.dbc|','DataFileDate',['24-11月-2020 15:06:17'],'SelectedFile','..\..\dbc\ep21_dbc\171114-lh1-ep21_ep2_fdr-_v07_acc.dbc','InterfaceFcn','rtican_dbc_file_parser'),'Options',struct('StatusSelected',1,'TimeSelected',1,'DeltaTimeSelected',1,'BytePortSelected',0,'MessageLengthSelected',0,'TriggerPort',struct('Selected',0,'TriggerType',0),'UserCoding',struct('Selected',0,'InterfaceFile','UserDecodingFile','FcnName','UserDecodeFcn','InportSelected',0,'InportWidth',1,'OutportSelected',0,'OutportWidth',1),'EnablePortSelected',0,'SignalOnPortnameSelected',1,'UseRXService',0),'Message',struct('MsgOnBlocknameSelected',1,'MsgName','GW_HSC2_ECM_FrP27','MsgIdFormat',0,'MsgId',251,'MsgLength',8,'NumSignals',4,'SampleTime',-1,'Signal',struct('SgnName',{'PtACCToqReqRespPVHSC2','PtADASAlvRCHSC2','AccelOvrdHSC2','PtACCToqReqRespHSC2'},'SgnStartBit',{16,20,43,58},'SgnLength',{4,4,1,3},'ByteLayout',{2,2,2,2},'Factor',{1,1,1,1},'Offset',{0,0,0,0},'SgnComment',{'','','',''},'SgnUnit',{'','','',''},'Min',{0,0,0,0},'Max',{15,15,1,7},'SgnType',{0,0,0,0},'SLDataType',{'SS_DOUBLE','SS_DOUBLE','SS_DOUBLE','SS_DOUBLE'},'DataType',{0,0,0,0},'ModeValue',{-1,-1,-1,-1}),'MsgIdNumFormat',0,'MsgComment',{{''}}),'Version',1.2,'general',struct('isFromLib',0)),'OFF',[]}},'GroupId',{{struct('Group',{{'RTICAN'}},'No',1,'Behavior',{{'NAMECHANGE'}},'BlockType',{{'SINK'}},'NameChangeFlag',0),'OFF',[]}},'SFcnRTICANMessage',{{struct('MsgType','RX','SFcnPortType','Scalar','MsgName','GW_HSC2_ECM_FrP27','MsgIdFormat','STD','MsgId',251,'MsgLength',8,'NumSignals',4,'SampleTime',-1,'Signal',struct('SgnName',{'PtACCToqReqRespPVHSC2','PtADASAlvRCHSC2','AccelOvrdHSC2','PtACCToqReqRespHSC2'},'SgnStartBit',{16,20,43,58},'SgnLength',{4,4,1,3},'ByteLayout',{['motorola back.'],['motorola back.'],['motorola back.'],['motorola back.']},'Factor',{1,1,1,1},'Offset',{0,0,0,0},'SgnType',{'standard','standard','standard','standard'},'SLDataType',{'SS_DOUBLE','SS_DOUBLE','SS_DOUBLE','SS_DOUBLE'},'DataType',{['unsigned int'],['unsigned int'],['unsigned int'],['unsigned int']},'ModeValue',{-1,-1,-1,-1}),'StatusSelected','yes','TimeSelected','yes','DeltaTimeSelected','yes','BytePortSelected','no','MessageLengthSelected','no','TriggerPort',struct('Selected','no','TriggerType',0),'UserCoding',struct('Selected','no','InterfaceFile','UserDecodingFile','FcnName','UserDecodeFcn','InportSelected','no','InportWidth',1,'OutportSelected','no','OutportWidth',1),'EnablePortSelected','no','UseRXService','no','BoardType','DS1','BoardNo',1,'ControllerNo',1),'OFF',[]}},'TLCFileName',{{'rtican_rx_message','OFF',[]}})  RTISFcnParameters=struct('SFcnRTICANMessage','struct','TLCFileName','char')  RTIBlockParaDefault=struct('BoardTypeNo',4302,'BoardNo',1,'ChannelNo',1,'Parameters',struct('DataFileSupport',struct('DataFileSelectedMaster',0,'DataFileSelectedLocal',0,'DataFileName','','DataFileDate','','SelectedFile',['<no file selected>']),'Options',struct('StatusSelected',1,'TimeSelected',1,'DeltaTimeSelected',1,'BytePortSelected',0,'MessageLengthSelected',0,'TriggerPort',struct('Selected',0,'TriggerType','rising'),'UserCoding',struct('Selected',0,'InterfaceFile','UserDecodingFile','FcnName','UserDecodeFcn','InportSelected',0,'InportWidth',1,'OutportSelected',0,'OutportWidth',1),'EnablePortSelected',0,'SignalOnPortnameSelected',1,'UseRXService',0),'Message',struct('MsgOnBlocknameSelected',0,'MsgName',['RX Message'],'MsgIdFormat',0,'MsgId',100,'MsgLength',8,'NumSignals',1,'SampleTime',-1,'Signal',struct('SgnName',['RX signal'],'SgnStartBit',0,'SgnLength',8,'SgnType',0,'ModeValue',-1,'DataType',0,'SLDataType','SS_DOUBLE','ByteLayout',0,'Factor',1,'Offset',0,'Min',0,'Max',255,'SgnComment',{{}},'SgnUnit',''),'MsgIdNumFormat',0,'MsgComment',{{''}}),'Version',1.2,'general',struct('isFromLib',1)),'GroupId',struct('Group',{{'RTICAN'}},'No',1,'Behavior',{{'NAMECHANGE'}},'BlockType',{{'SINK'}},'NameChangeFlag',0),'SFcnRTICANMessage',struct('MsgType','RX','MsgName',['RX Message'],'MsgIdFormat','STD','MsgId',100,'MsgLength',8,'NumSignals',1,'SampleTime',-1,'Signal',struct('SgnName',['RX signal'],'SgnStartBit',0,'SgnLength',8,'SgnType','standard','ModeValue',-1,'DataType',['unsigned int'],'ByteLayout',['little endian'],'SLDataType','SS_DOUBLE','Factor',1,'Offset',0),'StatusSelected','yes','TimeSelected','yes','DeltaTimeSelected','yes','BytePortSelected','no','MessageLengthSelected','no','EnablePortSelected','no','UserCoding',struct('Selected','no','InterfaceFile','UserDecodingFile','FcnName','UserDecodeFcn','InportSelected','no','InportWidth',1,'OutportSelected','no','OutportWidth',1),'TriggerPort',struct('Selected','no','TriggerType','rising'),'UseRXService','no','BoardType','DS4302','BoardNo',1,'ControllerNo',1,'SFcnPortType','Scalar'),'TLCFileName','rtican_rx_message')
      settings: AttributesFormatString=Group Id: RTICAN1\n  SourceProductName=dSPACE RTI CAN Blockset
  GW_HSC2_FICM_FrP02_0x376 : rtican/RTICAN Receive (RX)   Reserved1=[]  Reserved2=[]  Reserved3=[]  Reserved4=[]  SfcnMessage=[]  Msg_Struct=[]  BoardTypeNo=[]  BoardNo=[]  ChannelNo=[]  Parameters=[]  DialogFcn=[]  UnitName=[]  Revision=[]  UnitValues=[]  DSProperties=struct('RTI',struct('Version',uint32(5),'BlockType',struct('isSLSource',uint8(1),'isSLSink',uint8(1),'isHWSource',uint8(0),'isHWSink',uint8(0),'isSetup',uint8(0),'isInline',uint8(1),'isNonInline',uint8(0),'isInterrupt',uint8(0),'isChannelwise',uint8(0)),'IOBoardType','RTICAN','UnitType','MESSAGE','Identifier','RX','DialogType','MSVC','BlockSet','RTICAN','SlaveProcessor','CAN'))  RTIBlockInterface=struct('OutputPortsWidth',int32([1 1 1 1 1]),'OutputPortsActive',[1 1 1 1 1],'OutputPortsName',{{'RstrFctryDeftsReqHSC2','LDWLKASwReqHSC2',['RX status'],['RX time'],['RX delta time']}},'OutputPortsDataType',{{'SS_DOUBLE','SS_DOUBLE','SS_DOUBLE','SS_DOUBLE','SS_DOUBLE'}},'OutputPortsLabel',{{'RstrFctryDeftsReqHSC2','LDWLKASwReqHSC2','','',''}},'OutputPortsLabelMode','ON','InputPortsWidth',int32(0),'InputPortsActive',0,'DialogFcn','rtican_message_interface_gui','BlockDisplay',{{'','center'}},'IconTransparency','on','ParameterTunableNames',{{}},'InitLevel',3,'BlockName',struct('Token',{{'GW_HSC2_FICM_FrP02'}}),'SampleTime',{{-1}},'TriggerPort',{{'none'}},'EnablePort',{{'none'}})  RTIBlockParameters=struct('BoardTypeNo',{{1,'OFF',[]}},'BoardNo',{{1,'ON',[1 16]}},'ChannelNo',{{1,'ON',[1 2]}},'Parameters',{{struct('DataFileSupport',struct('DataFileSelectedMaster',1,'DataFileSelectedLocal',1,'DataFileName','c:\users\linqi\desktop\matlab\acc\dbc\ep21_dbc\171114-lh1-ep21_ep2_fdr-_v07_acc.dbc|','DataFileDate',{{{['24-11月-2020 15:06:17']}}},'SelectedFile','..\..\dbc\ep21_dbc\171114-lh1-ep21_ep2_fdr-_v07_acc.dbc','InterfaceFcn','rtican_dbc_file_parser'),'Options',struct('StatusSelected',1,'TimeSelected',1,'DeltaTimeSelected',1,'BytePortSelected',0,'MessageLengthSelected',0,'TriggerPort',struct('Selected',0,'TriggerType',0),'UserCoding',struct('Selected',0,'InterfaceFile','UserDecodingFile','FcnName','UserDecodeFcn','InportSelected',0,'InportWidth',1,'OutportSelected',0,'OutportWidth',1),'EnablePortSelected',0,'SignalOnPortnameSelected',1,'UseRXService',0),'Message',struct('MsgOnBlocknameSelected',1,'MsgName','GW_HSC2_FICM_FrP02','MsgIdFormat',0,'MsgId',886,'MsgLength',8,'NumSignals',2,'SampleTime',-1,'Signal',struct('SgnName',{'RstrFctryDeftsReqHSC2','LDWLKASwReqHSC2'},'SgnStartBit',{0,37},'SgnLength',{1,3},'SgnType',{0,0},'ModeValue',{-1,-1},'DataType',{0,0},'ByteLayout',{2,2},'Factor',{1,1},'Offset',{0,0},'SgnComment',{{''},{''}},'SgnUnit',{'',''},'Min',{0,0},'Max',{1,7},'SLDataType',{'SS_DOUBLE','SS_DOUBLE'}),'MsgIdNumFormat',1,'MsgComment',{{''}}),'Version',1.2,'general',struct('isFromLib',0)),'OFF',[]}},'GroupId',{{struct('Group',{{'RTICAN'}},'No',1,'Behavior',{{'NAMECHANGE'}},'BlockType',{{'SINK'}},'NameChangeFlag',0),'OFF',[]}},'SFcnRTICANMessage',{{struct('MsgType','RX','SFcnPortType','Scalar','MsgName','GW_HSC2_FICM_FrP02','MsgIdFormat','STD','MsgId',886,'MsgLength',8,'NumSignals',2,'SampleTime',-1,'Signal',struct('SgnName',{'RstrFctryDeftsReqHSC2','LDWLKASwReqHSC2'},'SgnStartBit',{0,37},'SgnLength',{1,3},'SgnType',{'standard','standard'},'ModeValue',{-1,-1},'DataType',{['unsigned int'],['unsigned int']},'ByteLayout',{['motorola back.'],['motorola back.']},'Factor',{1,1},'Offset',{0,0},'SLDataType',{'SS_DOUBLE','SS_DOUBLE'}),'StatusSelected','yes','TimeSelected','yes','DeltaTimeSelected','yes','BytePortSelected','no','MessageLengthSelected','no','TriggerPort',struct('Selected','no','TriggerType',0),'UserCoding',struct('Selected','no','InterfaceFile','UserDecodingFile','FcnName','UserDecodeFcn','InportSelected','no','InportWidth',1,'OutportSelected','no','OutportWidth',1),'EnablePortSelected','no','UseRXService','no','BoardType','DS1','BoardNo',1,'ControllerNo',1),'OFF',[]}},'TLCFileName',{{'rtican_rx_message','OFF',[]}})  RTISFcnParameters=struct('SFcnRTICANMessage','struct','TLCFileName','char')  RTIBlockParaDefault=struct('BoardTypeNo',4302,'BoardNo',1,'ChannelNo',1,'Parameters',struct('DataFileSupport',struct('DataFileSelectedMaster',0,'DataFileSelectedLocal',0,'DataFileName','','DataFileDate','','SelectedFile',['<no file selected>']),'Options',struct('StatusSelected',1,'TimeSelected',1,'DeltaTimeSelected',1,'BytePortSelected',0,'MessageLengthSelected',0,'TriggerPort',struct('Selected',0,'TriggerType','rising'),'UserCoding',struct('Selected',0,'InterfaceFile','UserDecodingFile','FcnName','UserDecodeFcn','InportSelected',0,'InportWidth',1,'OutportSelected',0,'OutportWidth',1),'EnablePortSelected',0,'SignalOnPortnameSelected',1,'UseRXService',0),'Message',struct('MsgOnBlocknameSelected',0,'MsgName',['RX Message'],'MsgIdFormat',0,'MsgId',100,'MsgLength',8,'NumSignals',1,'SampleTime',-1,'Signal',struct('SgnName',['RX signal'],'SgnStartBit',0,'SgnLength',8,'SgnType',0,'ModeValue',-1,'DataType',0,'SLDataType','SS_DOUBLE','ByteLayout',0,'Factor',1,'Offset',0,'Min',0,'Max',255,'SgnComment',{{}},'SgnUnit',''),'MsgIdNumFormat',0,'MsgComment',{{''}}),'Version',1.2,'general',struct('isFromLib',1)),'GroupId',struct('Group',{{'RTICAN'}},'No',1,'Behavior',{{'NAMECHANGE'}},'BlockType',{{'SINK'}},'NameChangeFlag',0),'SFcnRTICANMessage',struct('MsgType','RX','MsgName',['RX Message'],'MsgIdFormat','STD','MsgId',100,'MsgLength',8,'NumSignals',1,'SampleTime',-1,'Signal',struct('SgnName',['RX signal'],'SgnStartBit',0,'SgnLength',8,'SgnType','standard','ModeValue',-1,'DataType',['unsigned int'],'ByteLayout',['little endian'],'SLDataType','SS_DOUBLE','Factor',1,'Offset',0),'StatusSelected','yes','TimeSelected','yes','DeltaTimeSelected','yes','BytePortSelected','no','MessageLengthSelected','no','EnablePortSelected','no','UserCoding',struct('Selected','no','InterfaceFile','UserDecodingFile','FcnName','UserDecodeFcn','InportSelected','no','InportWidth',1,'OutportSelected','no','OutportWidth',1),'TriggerPort',struct('Selected','no','TriggerType','rising'),'UseRXService','no','BoardType','DS4302','BoardNo',1,'ControllerNo',1,'SFcnPortType','Scalar'),'TLCFileName','rtican_rx_message')
      settings: AttributesFormatString=Group Id: RTICAN1\n  SourceProductName=dSPACE RTI CAN Blockset
  GW_HSC2_FrP04_0x1E1 : rtican/RTICAN Receive (RX)   Reserved1=[]  Reserved2=[]  Reserved3=[]  Reserved4=[]  SfcnMessage=[]  Msg_Struct=[]  BoardTypeNo=[]  BoardNo=[]  ChannelNo=[]  Parameters=[]  DialogFcn=[]  UnitName=[]  Revision=[]  UnitValues=[]  DSProperties=struct('RTI',struct('Version',uint32(5),'BlockType',struct('isSLSource',uint8(1),'isSLSink',uint8(1),'isHWSource',uint8(0),'isHWSink',uint8(0),'isSetup',uint8(0),'isInline',uint8(1),'isNonInline',uint8(0),'isInterrupt',uint8(0),'isChannelwise',uint8(0)),'IOBoardType','RTICAN','UnitType','MESSAGE','Identifier','RX','DialogType','MSVC','BlockSet','RTICAN','SlaveProcessor','CAN'))  RTIBlockInterface=struct('OutputPortsWidth',int32([1 1 1 1 1 1 1 1 1 1 1 1 1 1]),'OutputPortsActive',ones(1,14),'OutputPortsName',{{'CCSwStsAlvRC_h2HSC2','CCSwStsDistDecSwA_h2HSC2','CCSwStsDistIncSwA_h2HSC2','CCSwStsPV_h2HSC2','CCSwStsSwDataIntgty_h2HSC2','CCSwStsSpdDecSwA_h2HSC2','CCSwStsSpdIncSwA_h2HSC2','CCSwStsSetSwA_h2HSC2','CCSwStsRsmSwA_h2HSC2','CCSwStsOnSwA_h2HSC2','CCSwStsCanclSwA_h2HSC2',['RX status'],['RX time'],['RX delta time']}},'OutputPortsDataType',{{'SS_DOUBLE','SS_DOUBLE','SS_DOUBLE','SS_DOUBLE','SS_DOUBLE','SS_DOUBLE','SS_DOUBLE','SS_DOUBLE','SS_DOUBLE','SS_DOUBLE','SS_DOUBLE','SS_DOUBLE','SS_DOUBLE','SS_DOUBLE'}},'OutputPortsLabel',{{'CCSwStsAlvRC_h2HSC2','CCSwStsDistDecSwA_h2HSC2','CCSwStsDistIncSwA_h2HSC2','CCSwStsPV_h2HSC2','CCSwStsSwDataIntgty_h2HSC2','CCSwStsSpdDecSwA_h2HSC2','CCSwStsSpdIncSwA_h2HSC2','CCSwStsSetSwA_h2HSC2','CCSwStsRsmSwA_h2HSC2','CCSwStsOnSwA_h2HSC2','CCSwStsCanclSwA_h2HSC2','','',''}},'OutputPortsLabelMode','ON','InputPortsWidth',int32(0),'InputPortsActive',0,'DialogFcn','rtican_message_interface_gui','BlockDisplay',{{'','center'}},'IconTransparency','on','ParameterTunableNames',{{}},'InitLevel',3,'BlockName',struct('Token',{{'GW_HSC2_FrP04'}}),'SampleTime',{{-1}},'TriggerPort',{{'none'}},'EnablePort',{{'none'}})  RTIBlockParameters=struct('BoardTypeNo',{{1,'OFF',[]}},'BoardNo',{{1,'ON',[1 16]}},'ChannelNo',{{1,'ON',[1 2]}},'Parameters',{{struct('DataFileSupport',struct('DataFileSelectedMaster',1,'DataFileSelectedLocal',1,'DataFileName','c:\users\linqi\desktop\matlab\acc\dbc\ep21_dbc\171114-lh1-ep21_ep2_fdr-_v07.dbc|','DataFileDate',['24-11月-2020 15:06:17'],'SelectedFile','..\..\dbc\ep21_dbc\171114-lh1-ep21_ep2_fdr-_v07_acc.dbc','InterfaceFcn','rtican_dbc_file_parser'),'Options',struct('StatusSelected',1,'TimeSelected',1,'DeltaTimeSelected',1,'BytePortSelected',0,'MessageLengthSelected',0,'TriggerPort',struct('Selected',0,'TriggerType',0),'UserCoding',struct('Selected',0,'InterfaceFile','UserDecodingFile','FcnName','UserDecodeFcn','InportSelected',0,'InportWidth',1,'OutportSelected',0,'OutportWidth',1),'EnablePortSelected',0,'SignalOnPortnameSelected',1,'UseRXService',0),'Message',struct('MsgOnBlocknameSelected',1,'MsgName','GW_HSC2_FrP04','MsgIdFormat',0,'MsgId',481,'MsgLength',7,'NumSignals',11,'SampleTime',-1,'Signal',struct('SgnName',{'CCSwStsAlvRC_h2HSC2','CCSwStsDistDecSwA_h2HSC2','CCSwStsDistIncSwA_h2HSC2','CCSwStsPV_h2HSC2','CCSwStsSwDataIntgty_h2HSC2','CCSwStsSpdDecSwA_h2HSC2','CCSwStsSpdIncSwA_h2HSC2','CCSwStsSetSwA_h2HSC2','CCSwStsRsmSwA_h2HSC2','CCSwStsOnSwA_h2HSC2','CCSwStsCanclSwA_h2HSC2'},'SgnStartBit',{32,34,35,40,48,50,51,52,53,54,55},'SgnLength',{2,1,1,8,2,1,1,1,1,1,1},'ByteLayout',{2,2,2,2,2,2,2,2,2,2,2},'Factor',{1,1,1,1,1,1,1,1,1,1,1},'Offset',{0,0,0,0,0,0,0,0,0,0,0},'SgnComment',{'','','','','','','','','','',''},'SgnUnit',{'','','','','','','','','','',''},'Min',{0,0,0,0,0,0,0,0,0,0,0},'Max',{3,1,1,255,3,1,1,1,1,1,1},'SgnType',{0,0,0,0,0,0,0,0,0,0,0},'SLDataType',{'SS_DOUBLE','SS_DOUBLE','SS_DOUBLE','SS_DOUBLE','SS_DOUBLE','SS_DOUBLE','SS_DOUBLE','SS_DOUBLE','SS_DOUBLE','SS_DOUBLE','SS_DOUBLE'},'DataType',{0,0,0,0,0,0,0,0,0,0,0},'ModeValue',{-1,-1,-1,-1,-1,-1,-1,-1,-1,-1,-1}),'MsgIdNumFormat',0,'MsgComment',{{''}}),'Version',1.2,'general',struct('isFromLib',0)),'OFF',[]}},'GroupId',{{struct('Group',{{'RTICAN'}},'No',1,'Behavior',{{'NAMECHANGE'}},'BlockType',{{'SINK'}},'NameChangeFlag',0),'OFF',[]}},'SFcnRTICANMessage',{{struct('MsgType','RX','SFcnPortType','Scalar','MsgName','GW_HSC2_FrP04','MsgIdFormat','STD','MsgId',481,'MsgLength',7,'NumSignals',11,'SampleTime',-1,'Signal',struct('SgnName',{'CCSwStsAlvRC_h2HSC2','CCSwStsDistDecSwA_h2HSC2','CCSwStsDistIncSwA_h2HSC2','CCSwStsPV_h2HSC2','CCSwStsSwDataIntgty_h2HSC2','CCSwStsSpdDecSwA_h2HSC2','CCSwStsSpdIncSwA_h2HSC2','CCSwStsSetSwA_h2HSC2','CCSwStsRsmSwA_h2HSC2','CCSwStsOnSwA_h2HSC2','CCSwStsCanclSwA_h2HSC2'},'SgnStartBit',{32,34,35,40,48,50,51,52,53,54,55},'SgnLength',{2,1,1,8,2,1,1,1,1,1,1},'ByteLayout',{['motorola back.'],['motorola back.'],['motorola back.'],['motorola back.'],['motorola back.'],['motorola back.'],['motorola back.'],['motorola back.'],['motorola back.'],['motorola back.'],['motorola back.']},'Factor',{1,1,1,1,1,1,1,1,1,1,1},'Offset',{0,0,0,0,0,0,0,0,0,0,0},'SgnType',{'standard','standard','standard','standard','standard','standard','standard','standard','standard','standard','standard'},'SLDataType',{'SS_DOUBLE','SS_DOUBLE','SS_DOUBLE','SS_DOUBLE','SS_DOUBLE','SS_DOUBLE','SS_DOUBLE','SS_DOUBLE','SS_DOUBLE','SS_DOUBLE','SS_DOUBLE'},'DataType',{['unsigned int'],['unsigned int'],['unsigned int'],['unsigned int'],['unsigned int'],['unsigned int'],['unsigned int'],['unsigned int'],['unsigned int'],['unsigned int'],['unsigned int']},'ModeValue',{-1,-1,-1,-1,-1,-1,-1,-1,-1,-1,-1}),'StatusSelected','yes','TimeSelected','yes','DeltaTimeSelected','yes','BytePortSelected','no','MessageLengthSelected','no','TriggerPort',struct('Selected','no','TriggerType',0),'UserCoding',struct('Selected','no','InterfaceFile','UserDecodingFile','FcnName','UserDecodeFcn','InportSelected','no','InportWidth',1,'OutportSelected','no','OutportWidth',1),'EnablePortSelected','no','UseRXService','no','BoardType','DS1','BoardNo',1,'ControllerNo',1),'OFF',[]}},'TLCFileName',{{'rtican_rx_message','OFF',[]}})  RTISFcnParameters=struct('SFcnRTICANMessage','struct','TLCFileName','char')  RTIBlockParaDefault=struct('BoardTypeNo',4302,'BoardNo',1,'ChannelNo',1,'Parameters',struct('DataFileSupport',struct('DataFileSelectedMaster',0,'DataFileSelectedLocal',0,'DataFileName','','DataFileDate','','SelectedFile',['<no file selected>']),'Options',struct('StatusSelected',1,'TimeSelected',1,'DeltaTimeSelected',1,'BytePortSelected',0,'MessageLengthSelected',0,'TriggerPort',struct('Selected',0,'TriggerType','rising'),'UserCoding',struct('Selected',0,'InterfaceFile','UserDecodingFile','FcnName','UserDecodeFcn','InportSelected',0,'InportWidth',1,'OutportSelected',0,'OutportWidth',1),'EnablePortSelected',0,'SignalOnPortnameSelected',1,'UseRXService',0),'Message',struct('MsgOnBlocknameSelected',0,'MsgName',['RX Message'],'MsgIdFormat',0,'MsgId',100,'MsgLength',8,'NumSignals',1,'SampleTime',-1,'Signal',struct('SgnName',['RX signal'],'SgnStartBit',0,'SgnLength',8,'SgnType',0,'ModeValue',-1,'DataType',0,'SLDataType','SS_DOUBLE','ByteLayout',0,'Factor',1,'Offset',0,'Min',0,'Max',255,'SgnComment',{{}},'SgnUnit',''),'MsgIdNumFormat',0,'MsgComment',{{''}}),'Version',1.2,'general',struct('isFromLib',1)),'GroupId',struct('Group',{{'RTICAN'}},'No',1,'Behavior',{{'NAMECHANGE'}},'BlockType',{{'SINK'}},'NameChangeFlag',0),'SFcnRTICANMessage',struct('MsgType','RX','MsgName',['RX Message'],'MsgIdFormat','STD','MsgId',100,'MsgLength',8,'NumSignals',1,'SampleTime',-1,'Signal',struct('SgnName',['RX signal'],'SgnStartBit',0,'SgnLength',8,'SgnType','standard','ModeValue',-1,'DataType',['unsigned int'],'ByteLayout',['little endian'],'SLDataType','SS_DOUBLE','Factor',1,'Offset',0),'StatusSelected','yes','TimeSelected','yes','DeltaTimeSelected','yes','BytePortSelected','no','MessageLengthSelected','no','EnablePortSelected','no','UserCoding',struct('Selected','no','InterfaceFile','UserDecodingFile','FcnName','UserDecodeFcn','InportSelected','no','InportWidth',1,'OutportSelected','no','OutportWidth',1),'TriggerPort',struct('Selected','no','TriggerType','rising'),'UseRXService','no','BoardType','DS4302','BoardNo',1,'ControllerNo',1,'SFcnPortType','Scalar'),'TLCFileName','rtican_rx_message')
      settings: AttributesFormatString=Group Id: RTICAN1\n  SourceProductName=dSPACE RTI CAN Blockset
  GW_HSC2_HCU_FrP00_0xAF : rtican/RTICAN Receive (RX)   Reserved1=[]  Reserved2=[]  Reserved3=[]  Reserved4=[]  SfcnMessage=[]  Msg_Struct=[]  BoardTypeNo=[]  BoardNo=[]  ChannelNo=[]  Parameters=[]  DialogFcn=[]  UnitName=[]  Revision=[]  UnitValues=[]  DSProperties=struct('RTI',struct('Version',uint32(5),'BlockType',struct('isSLSource',uint8(1),'isSLSink',uint8(1),'isHWSource',uint8(0),'isHWSink',uint8(0),'isSetup',uint8(0),'isInline',uint8(1),'isNonInline',uint8(0),'isInterrupt',uint8(0),'isChannelwise',uint8(0)),'IOBoardType','RTICAN','UnitType','MESSAGE','Identifier','RX','DialogType','MSVC','BlockSet','RTICAN','SlaveProcessor','CAN'))  RTIBlockInterface=struct('OutputPortsWidth',int32([1 1 1 1 1 1 1 1 1 1 1]),'OutputPortsActive',ones(1,11),'OutputPortsName',{{'EPTAccelActuPosPVHSC2','EPTAccelActuPosVHSC2','HCU_FrP00_RollingCounterHSC2','EPTBrkPdlDscrtInptStsHSC2','EPTBrkPdlDscrtInptStsVHSC2','EPTStCmdOn_h1HSC2','EPTBrkPdlDscrtInptStsPVHSC2','EPTAccelActuPosHSC2',['RX status'],['RX time'],['RX delta time']}},'OutputPortsDataType',{{'SS_DOUBLE','SS_DOUBLE','SS_DOUBLE','SS_DOUBLE','SS_DOUBLE','SS_DOUBLE','SS_DOUBLE','SS_DOUBLE','SS_DOUBLE','SS_DOUBLE','SS_DOUBLE'}},'OutputPortsLabel',{{'EPTAccelActuPosPVHSC2','EPTAccelActuPosVHSC2','HCU_FrP00_RollingCounterHSC2','EPTBrkPdlDscrtInptStsHSC2','EPTBrkPdlDscrtInptStsVHSC2','EPTStCmdOn_h1HSC2','EPTBrkPdlDscrtInptStsPVHSC2','EPTAccelActuPosHSC2','','',''}},'OutputPortsLabelMode','ON','InputPortsWidth',int32(0),'InputPortsActive',0,'DialogFcn','rtican_message_interface_gui','BlockDisplay',{{'','center'}},'IconTransparency','on','ParameterTunableNames',{{}},'InitLevel',3,'BlockName',struct('Token',{{'GW_HSC2_HCU_FrP00'}}),'SampleTime',{{-1}},'TriggerPort',{{'none'}},'EnablePort',{{'none'}})  RTIBlockParameters=struct('BoardTypeNo',{{1,'OFF',[]}},'BoardNo',{{1,'ON',[1 16]}},'ChannelNo',{{1,'ON',[1 2]}},'Parameters',{{struct('DataFileSupport',struct('DataFileSelectedMaster',1,'DataFileSelectedLocal',1,'DataFileName','c:\users\linqi\desktop\matlab\acc\dbc\ep21_dbc\171114-lh1-ep21_ep2_fdr-_v07.dbc|','DataFileDate',['24-11月-2020 15:06:17'],'SelectedFile','..\..\dbc\ep21_dbc\171114-lh1-ep21_ep2_fdr-_v07_acc.dbc','InterfaceFcn','rtican_dbc_file_parser'),'Options',struct('StatusSelected',1,'TimeSelected',1,'DeltaTimeSelected',1,'BytePortSelected',0,'MessageLengthSelected',0,'TriggerPort',struct('Selected',0,'TriggerType',0),'UserCoding',struct('Selected',0,'InterfaceFile','UserDecodingFile','FcnName','UserDecodeFcn','InportSelected',0,'InportWidth',1,'OutportSelected',0,'OutportWidth',1),'EnablePortSelected',0,'SignalOnPortnameSelected',1,'UseRXService',0),'Message',struct('MsgOnBlocknameSelected',1,'MsgName','GW_HSC2_HCU_FrP00','MsgIdFormat',0,'MsgId',175,'MsgLength',8,'NumSignals',8,'SampleTime',-1,'Signal',struct('SgnName',{'EPTAccelActuPosPVHSC2','EPTAccelActuPosVHSC2','HCU_FrP00_RollingCounterHSC2','EPTBrkPdlDscrtInptStsHSC2','EPTBrkPdlDscrtInptStsVHSC2','EPTStCmdOn_h1HSC2','EPTBrkPdlDscrtInptStsPVHSC2','EPTAccelActuPosHSC2'},'SgnStartBit',{8,19,20,39,40,41,42,56},'SgnLength',{9,1,4,1,1,1,4,8},'ByteLayout',{2,2,2,2,2,2,2,2},'Factor',{1,1,1,1,1,1,1,0.392157},'Offset',{0,0,0,0,0,0,0,0},'SgnComment',{['Electric Powertrain Accelerator Actual Position Protection Value'],'','','',['Electric Powertrain Brake Pedal Discrete Input Status Validity'],'',['Electric Powertrain Brake Pedal Discrete Input Status Protection Value'],''},'SgnUnit',{'','','','','','','','%'},'Min',{0,0,0,0,0,0,0,0},'Max',{511,1,15,1,1,1,15,100},'SgnType',{0,0,0,0,0,0,0,0},'SLDataType',{'SS_DOUBLE','SS_DOUBLE','SS_DOUBLE','SS_DOUBLE','SS_DOUBLE','SS_DOUBLE','SS_DOUBLE','SS_DOUBLE'},'DataType',{0,0,0,0,0,0,0,0},'ModeValue',{-1,-1,-1,-1,-1,-1,-1,-1}),'MsgIdNumFormat',0,'MsgComment',{{''}}),'Version',1.2,'general',struct('isFromLib',0)),'OFF',[]}},'GroupId',{{struct('Group',{{'RTICAN'}},'No',1,'Behavior',{{'NAMECHANGE'}},'BlockType',{{'SINK'}},'NameChangeFlag',0),'OFF',[]}},'SFcnRTICANMessage',{{struct('MsgType','RX','SFcnPortType','Scalar','MsgName','GW_HSC2_HCU_FrP00','MsgIdFormat','STD','MsgId',175,'MsgLength',8,'NumSignals',8,'SampleTime',-1,'Signal',struct('SgnName',{'EPTAccelActuPosPVHSC2','EPTAccelActuPosVHSC2','HCU_FrP00_RollingCounterHSC2','EPTBrkPdlDscrtInptStsHSC2','EPTBrkPdlDscrtInptStsVHSC2','EPTStCmdOn_h1HSC2','EPTBrkPdlDscrtInptStsPVHSC2','EPTAccelActuPosHSC2'},'SgnStartBit',{8,19,20,39,40,41,42,56},'SgnLength',{9,1,4,1,1,1,4,8},'ByteLayout',{['motorola back.'],['motorola back.'],['motorola back.'],['motorola back.'],['motorola back.'],['motorola back.'],['motorola back.'],['motorola back.']},'Factor',{1,1,1,1,1,1,1,0.392157},'Offset',{0,0,0,0,0,0,0,0},'SgnType',{'standard','standard','standard','standard','standard','standard','standard','standard'},'SLDataType',{'SS_DOUBLE','SS_DOUBLE','SS_DOUBLE','SS_DOUBLE','SS_DOUBLE','SS_DOUBLE','SS_DOUBLE','SS_DOUBLE'},'DataType',{['unsigned int'],['unsigned int'],['unsigned int'],['unsigned int'],['unsigned int'],['unsigned int'],['unsigned int'],['unsigned int']},'ModeValue',{-1,-1,-1,-1,-1,-1,-1,-1}),'StatusSelected','yes','TimeSelected','yes','DeltaTimeSelected','yes','BytePortSelected','no','MessageLengthSelected','no','TriggerPort',struct('Selected','no','TriggerType',0),'UserCoding',struct('Selected','no','InterfaceFile','UserDecodingFile','FcnName','UserDecodeFcn','InportSelected','no','InportWidth',1,'OutportSelected','no','OutportWidth',1),'EnablePortSelected','no','UseRXService','no','BoardType','DS1','BoardNo',1,'ControllerNo',1),'OFF',[]}},'TLCFileName',{{'rtican_rx_message','OFF',[]}})  RTISFcnParameters=struct('SFcnRTICANMessage','struct','TLCFileName','char')  RTIBlockParaDefault=struct('BoardTypeNo',4302,'BoardNo',1,'ChannelNo',1,'Parameters',struct('DataFileSupport',struct('DataFileSelectedMaster',0,'DataFileSelectedLocal',0,'DataFileName','','DataFileDate','','SelectedFile',['<no file selected>']),'Options',struct('StatusSelected',1,'TimeSelected',1,'DeltaTimeSelected',1,'BytePortSelected',0,'MessageLengthSelected',0,'TriggerPort',struct('Selected',0,'TriggerType','rising'),'UserCoding',struct('Selected',0,'InterfaceFile','UserDecodingFile','FcnName','UserDecodeFcn','InportSelected',0,'InportWidth',1,'OutportSelected',0,'OutportWidth',1),'EnablePortSelected',0,'SignalOnPortnameSelected',1,'UseRXService',0),'Message',struct('MsgOnBlocknameSelected',0,'MsgName',['RX Message'],'MsgIdFormat',0,'MsgId',100,'MsgLength',8,'NumSignals',1,'SampleTime',-1,'Signal',struct('SgnName',['RX signal'],'SgnStartBit',0,'SgnLength',8,'SgnType',0,'ModeValue',-1,'DataType',0,'SLDataType','SS_DOUBLE','ByteLayout',0,'Factor',1,'Offset',0,'Min',0,'Max',255,'SgnComment',{{}},'SgnUnit',''),'MsgIdNumFormat',0,'MsgComment',{{''}}),'Version',1.2,'general',struct('isFromLib',1)),'GroupId',struct('Group',{{'RTICAN'}},'No',1,'Behavior',{{'NAMECHANGE'}},'BlockType',{{'SINK'}},'NameChangeFlag',0),'SFcnRTICANMessage',struct('MsgType','RX','MsgName',['RX Message'],'MsgIdFormat','STD','MsgId',100,'MsgLength',8,'NumSignals',1,'SampleTime',-1,'Signal',struct('SgnName',['RX signal'],'SgnStartBit',0,'SgnLength',8,'SgnType','standard','ModeValue',-1,'DataType',['unsigned int'],'ByteLayout',['little endian'],'SLDataType','SS_DOUBLE','Factor',1,'Offset',0),'StatusSelected','yes','TimeSelected','yes','DeltaTimeSelected','yes','BytePortSelected','no','MessageLengthSelected','no','EnablePortSelected','no','UserCoding',struct('Selected','no','InterfaceFile','UserDecodingFile','FcnName','UserDecodeFcn','InportSelected','no','InportWidth',1,'OutportSelected','no','OutportWidth',1),'TriggerPort',struct('Selected','no','TriggerType','rising'),'UseRXService','no','BoardType','DS4302','BoardNo',1,'ControllerNo',1,'SFcnPortType','Scalar'),'TLCFileName','rtican_rx_message')
      settings: AttributesFormatString=Group Id: RTICAN1\n  SourceProductName=dSPACE RTI CAN Blockset
  GW_HSC2_HCU_FrP08_0xAC : rtican/RTICAN Receive (RX)   Reserved1=[]  Reserved2=[]  Reserved3=[]  Reserved4=[]  SfcnMessage=[]  Msg_Struct=[]  BoardTypeNo=[]  BoardNo=[]  ChannelNo=[]  Parameters=[]  DialogFcn=[]  UnitName=[]  Revision=[]  UnitValues=[]  DSProperties=struct('RTI',struct('Version',uint32(5),'BlockType',struct('isSLSource',uint8(1),'isSLSink',uint8(1),'isHWSource',uint8(0),'isHWSink',uint8(0),'isSetup',uint8(0),'isInline',uint8(1),'isNonInline',uint8(0),'isInterrupt',uint8(0),'isChannelwise',uint8(0)),'IOBoardType','RTICAN','UnitType','MESSAGE','Identifier','RX','DialogType','MSVC','BlockSet','RTICAN','SlaveProcessor','CAN'))  RTIBlockInterface=struct('OutputPortsWidth',int32([1 1 1 1 1 1 1 1 1]),'OutputPortsActive',[1 1 1 1 1 1 1 1 1],'OutputPortsName',{{'EPTTrInptShaftToqChksmHSC2','EPTTrInptShaftMaxAvlblToqHSC2','EPTTrInptShaftToqAlvRlngCtrHSC2','EPTTrInptShaftMinAvlblToqHSC2','EPTTrInptShaftMaxAvlblToqVHSC2','EPTTrInptShaftMinAvlblToqVHSC2',['RX status'],['RX time'],['RX delta time']}},'OutputPortsDataType',{{'SS_DOUBLE','SS_DOUBLE','SS_DOUBLE','SS_DOUBLE','SS_DOUBLE','SS_DOUBLE','SS_DOUBLE','SS_DOUBLE','SS_DOUBLE'}},'OutputPortsLabel',{{'EPTTrInptShaftToqChksmHSC2','EPTTrInptShaftMaxAvlblToqHSC2','EPTTrInptShaftToqAlvRlngCtrHSC2','EPTTrInptShaftMinAvlblToqHSC2','EPTTrInptShaftMaxAvlblToqVHSC2','EPTTrInptShaftMinAvlblToqVHSC2','','',''}},'OutputPortsLabelMode','ON','InputPortsWidth',int32(0),'InputPortsActive',0,'DialogFcn','rtican_message_interface_gui','BlockDisplay',{{'','center'}},'IconTransparency','on','ParameterTunableNames',{{}},'InitLevel',3,'BlockName',struct('Token',{{'GW_HSC2_HCU_FrP08'}}),'SampleTime',{{-1}},'TriggerPort',{{'none'}},'EnablePort',{{'none'}})  RTIBlockParameters=struct('BoardTypeNo',{{1,'OFF',[]}},'BoardNo',{{1,'ON',[1 16]}},'ChannelNo',{{1,'ON',[1 2]}},'Parameters',{{struct('DataFileSupport',struct('DataFileSelectedMaster',1,'DataFileSelectedLocal',1,'DataFileName','c:\users\linqi\desktop\matlab\acc\dbc\ep21_dbc\171114-lh1-ep21_ep2_fdr-_v07.dbc|','DataFileDate',['24-11月-2020 15:06:17'],'SelectedFile','..\..\dbc\ep21_dbc\171114-lh1-ep21_ep2_fdr-_v07_acc.dbc','InterfaceFcn','rtican_dbc_file_parser'),'Options',struct('StatusSelected',1,'TimeSelected',1,'DeltaTimeSelected',1,'BytePortSelected',0,'MessageLengthSelected',0,'TriggerPort',struct('Selected',0,'TriggerType',0),'UserCoding',struct('Selected',0,'InterfaceFile','UserDecodingFile','FcnName','UserDecodeFcn','InportSelected',0,'InportWidth',1,'OutportSelected',0,'OutportWidth',1),'EnablePortSelected',0,'SignalOnPortnameSelected',1,'UseRXService',0),'Message',struct('MsgOnBlocknameSelected',1,'MsgName','GW_HSC2_HCU_FrP08','MsgIdFormat',0,'MsgId',172,'MsgLength',8,'NumSignals',6,'SampleTime',-1,'Signal',struct('SgnName',{'EPTTrInptShaftToqChksmHSC2','EPTTrInptShaftMaxAvlblToqHSC2','EPTTrInptShaftToqAlvRlngCtrHSC2','EPTTrInptShaftMinAvlblToqHSC2','EPTTrInptShaftMaxAvlblToqVHSC2','EPTTrInptShaftMinAvlblToqVHSC2'},'SgnStartBit',{0,32,44,48,60,61},'SgnLength',{8,12,4,12,1,1},'ByteLayout',{2,2,2,2,2,2},'Factor',{1,2^-1,1,2^-1,1,1},'Offset',{0,-848,0,-848,0,0},'SgnComment',{['Electric Powertrain Transmission Input Shaft Torque Checksum'],'',['Electric Powertrain Transmission Input Shaft Torque Alive Rolling Counter'],'','',''},'SgnUnit',{'','Nm',['count value'],'Nm','',''},'Min',{0,-848,0,-848,0,0},'Max',{255,1199.5,15,1199.5,1,1},'SgnType',{0,0,0,0,0,0},'SLDataType',{'SS_DOUBLE','SS_DOUBLE','SS_DOUBLE','SS_DOUBLE','SS_DOUBLE','SS_DOUBLE'},'DataType',{0,0,0,0,0,0},'ModeValue',{-1,-1,-1,-1,-1,-1}),'MsgIdNumFormat',0,'MsgComment',{{''}}),'Version',1.2,'general',struct('isFromLib',0)),'OFF',[]}},'GroupId',{{struct('Group',{{'RTICAN'}},'No',1,'Behavior',{{'NAMECHANGE'}},'BlockType',{{'SINK'}},'NameChangeFlag',0),'OFF',[]}},'SFcnRTICANMessage',{{struct('MsgType','RX','SFcnPortType','Scalar','MsgName','GW_HSC2_HCU_FrP08','MsgIdFormat','STD','MsgId',172,'MsgLength',8,'NumSignals',6,'SampleTime',-1,'Signal',struct('SgnName',{'EPTTrInptShaftToqChksmHSC2','EPTTrInptShaftMaxAvlblToqHSC2','EPTTrInptShaftToqAlvRlngCtrHSC2','EPTTrInptShaftMinAvlblToqHSC2','EPTTrInptShaftMaxAvlblToqVHSC2','EPTTrInptShaftMinAvlblToqVHSC2'},'SgnStartBit',{0,32,44,48,60,61},'SgnLength',{8,12,4,12,1,1},'ByteLayout',{['motorola back.'],['motorola back.'],['motorola back.'],['motorola back.'],['motorola back.'],['motorola back.']},'Factor',{1,2^-1,1,2^-1,1,1},'Offset',{0,-848,0,-848,0,0},'SgnType',{'standard','standard','standard','standard','standard','standard'},'SLDataType',{'SS_DOUBLE','SS_DOUBLE','SS_DOUBLE','SS_DOUBLE','SS_DOUBLE','SS_DOUBLE'},'DataType',{['unsigned int'],['unsigned int'],['unsigned int'],['unsigned int'],['unsigned int'],['unsigned int']},'ModeValue',{-1,-1,-1,-1,-1,-1}),'StatusSelected','yes','TimeSelected','yes','DeltaTimeSelected','yes','BytePortSelected','no','MessageLengthSelected','no','TriggerPort',struct('Selected','no','TriggerType',0),'UserCoding',struct('Selected','no','InterfaceFile','UserDecodingFile','FcnName','UserDecodeFcn','InportSelected','no','InportWidth',1,'OutportSelected','no','OutportWidth',1),'EnablePortSelected','no','UseRXService','no','BoardType','DS1','BoardNo',1,'ControllerNo',1),'OFF',[]}},'TLCFileName',{{'rtican_rx_message','OFF',[]}})  RTISFcnParameters=struct('SFcnRTICANMessage','struct','TLCFileName','char')  RTIBlockParaDefault=struct('BoardTypeNo',4302,'BoardNo',1,'ChannelNo',1,'Parameters',struct('DataFileSupport',struct('DataFileSelectedMaster',0,'DataFileSelectedLocal',0,'DataFileName','','DataFileDate','','SelectedFile',['<no file selected>']),'Options',struct('StatusSelected',1,'TimeSelected',1,'DeltaTimeSelected',1,'BytePortSelected',0,'MessageLengthSelected',0,'TriggerPort',struct('Selected',0,'TriggerType','rising'),'UserCoding',struct('Selected',0,'InterfaceFile','UserDecodingFile','FcnName','UserDecodeFcn','InportSelected',0,'InportWidth',1,'OutportSelected',0,'OutportWidth',1),'EnablePortSelected',0,'SignalOnPortnameSelected',1,'UseRXService',0),'Message',struct('MsgOnBlocknameSelected',0,'MsgName',['RX Message'],'MsgIdFormat',0,'MsgId',100,'MsgLength',8,'NumSignals',1,'SampleTime',-1,'Signal',struct('SgnName',['RX signal'],'SgnStartBit',0,'SgnLength',8,'SgnType',0,'ModeValue',-1,'DataType',0,'SLDataType','SS_DOUBLE','ByteLayout',0,'Factor',1,'Offset',0,'Min',0,'Max',255,'SgnComment',{{}},'SgnUnit',''),'MsgIdNumFormat',0,'MsgComment',{{''}}),'Version',1.2,'general',struct('isFromLib',1)),'GroupId',struct('Group',{{'RTICAN'}},'No',1,'Behavior',{{'NAMECHANGE'}},'BlockType',{{'SINK'}},'NameChangeFlag',0),'SFcnRTICANMessage',struct('MsgType','RX','MsgName',['RX Message'],'MsgIdFormat','STD','MsgId',100,'MsgLength',8,'NumSignals',1,'SampleTime',-1,'Signal',struct('SgnName',['RX signal'],'SgnStartBit',0,'SgnLength',8,'SgnType','standard','ModeValue',-1,'DataType',['unsigned int'],'ByteLayout',['little endian'],'SLDataType','SS_DOUBLE','Factor',1,'Offset',0),'StatusSelected','yes','TimeSelected','yes','DeltaTimeSelected','yes','BytePortSelected','no','MessageLengthSelected','no','EnablePortSelected','no','UserCoding',struct('Selected','no','InterfaceFile','UserDecodingFile','FcnName','UserDecodeFcn','InportSelected','no','InportWidth',1,'OutportSelected','no','OutportWidth',1),'TriggerPort',struct('Selected','no','TriggerType','rising'),'UseRXService','no','BoardType','DS4302','BoardNo',1,'ControllerNo',1,'SFcnPortType','Scalar'),'TLCFileName','rtican_rx_message')
      settings: AttributesFormatString=Group Id: RTICAN1\n  SourceProductName=dSPACE RTI CAN Blockset
  GW_HSC2_HCU_FrP13_0x19C : rtican/RTICAN Receive (RX)   Reserved1=[]  Reserved2=[]  Reserved3=[]  Reserved4=[]  SfcnMessage=[]  Msg_Struct=[]  BoardTypeNo=[]  BoardNo=[]  ChannelNo=[]  Parameters=[]  DialogFcn=[]  UnitName=[]  Revision=[]  UnitValues=[]  DSProperties=struct('RTI',struct('Version',uint32(5),'BlockType',struct('isSLSource',uint8(1),'isSLSink',uint8(1),'isHWSource',uint8(0),'isHWSink',uint8(0),'isSetup',uint8(0),'isInline',uint8(1),'isNonInline',uint8(0),'isInterrupt',uint8(0),'isChannelwise',uint8(0)),'IOBoardType','RTICAN','UnitType','MESSAGE','Identifier','RX','DialogType','MSVC','BlockSet','RTICAN','SlaveProcessor','CAN'))  RTIBlockInterface=struct('OutputPortsWidth',int32([1 1 1 1 1 1 1 1]),'OutputPortsActive',[1 1 1 1 1 1 1 1],'OutputPortsName',{{'VCUNRCDAlvRCHSC2','EPTTrInptShaftSpdHSC2','EPTTrInptShaftToqHSC2','EPTTrInptShaftSpdVHSC2','EPTTrInptShaftToqVHSC2',['RX status'],['RX time'],['RX delta time']}},'OutputPortsDataType',{{'SS_DOUBLE','SS_DOUBLE','SS_DOUBLE','SS_DOUBLE','SS_DOUBLE','SS_DOUBLE','SS_DOUBLE','SS_DOUBLE'}},'OutputPortsLabel',{{'VCUNRCDAlvRCHSC2','EPTTrInptShaftSpdHSC2','EPTTrInptShaftToqHSC2','EPTTrInptShaftSpdVHSC2','EPTTrInptShaftToqVHSC2','','',''}},'OutputPortsLabelMode','ON','InputPortsWidth',int32(0),'InputPortsActive',0,'DialogFcn','rtican_message_interface_gui','BlockDisplay',{{'','center'}},'IconTransparency','on','ParameterTunableNames',{{}},'InitLevel',3,'BlockName',struct('Token',{{'GW_HSC2_HCU_FrP13'}}),'SampleTime',{{-1}},'TriggerPort',{{'none'}},'EnablePort',{{'none'}})  RTIBlockParameters=struct('BoardTypeNo',{{1,'OFF',[]}},'BoardNo',{{1,'ON',[1 16]}},'ChannelNo',{{1,'ON',[1 2]}},'Parameters',{{struct('DataFileSupport',struct('DataFileSelectedMaster',1,'DataFileSelectedLocal',1,'DataFileName','c:\users\linqi\desktop\matlab\acc\dbc\ep21_dbc\171114-lh1-ep21_ep2_fdr-_v07_acc.dbc|c:\users\linqi\desktop\matlab\acc\dbc\ep21_dbc\171120-lh1-ep21_ep2_fvcm-_v07_lka.dbc|','DataFileDate',{{{['24-11月-2020 15:06:17']},{['24-11月-2020 15:35:27']}}},'SelectedFile','..\..\dbc\ep21_dbc\171114-lh1-ep21_ep2_fdr-_v07_acc.dbc','InterfaceFcn','rtican_dbc_file_parser'),'Options',struct('StatusSelected',1,'TimeSelected',1,'DeltaTimeSelected',1,'BytePortSelected',0,'MessageLengthSelected',0,'TriggerPort',struct('Selected',0,'TriggerType',0),'UserCoding',struct('Selected',0,'InterfaceFile','UserDecodingFile','FcnName','UserDecodeFcn','InportSelected',0,'InportWidth',1,'OutportSelected',0,'OutportWidth',1),'EnablePortSelected',0,'SignalOnPortnameSelected',1,'UseRXService',0),'Message',struct('MsgOnBlocknameSelected',1,'MsgName','GW_HSC2_HCU_FrP13','MsgIdFormat',0,'MsgId',412,'MsgLength',8,'NumSignals',5,'SampleTime',-1,'Signal',struct('SgnName',{'VCUNRCDAlvRCHSC2','EPTTrInptShaftSpdHSC2','EPTTrInptShaftToqHSC2','EPTTrInptShaftSpdVHSC2','EPTTrInptShaftToqVHSC2'},'SgnStartBit',{8,16,32,61,62},'SgnLength',{4,16,12,1,1},'SgnType',{0,0,0,0,0},'ModeValue',{-1,-1,-1,-1,-1},'DataType',{0,0,0,0,0},'ByteLayout',{2,2,2,2,2},'Factor',{1,1,2^-1,1,1},'Offset',{0,-32767,-848,0,0},'SgnComment',{{''},{''},{''},{''},{''}},'SgnUnit',{'','rpm','Nm','',''},'Min',{0,-32767,-848,0,0},'Max',{15,32768,1199.5,1,1},'SLDataType',{'SS_DOUBLE','SS_DOUBLE','SS_DOUBLE','SS_DOUBLE','SS_DOUBLE'}),'MsgIdNumFormat',1,'MsgComment',{{''}}),'Version',1.2,'general',struct('isFromLib',0)),'OFF',[]}},'GroupId',{{struct('Group',{{'RTICAN'}},'No',1,'Behavior',{{'NAMECHANGE'}},'BlockType',{{'SINK'}},'NameChangeFlag',0),'OFF',[]}},'SFcnRTICANMessage',{{struct('MsgType','RX','SFcnPortType','Scalar','MsgName','GW_HSC2_HCU_FrP13','MsgIdFormat','STD','MsgId',412,'MsgLength',8,'NumSignals',5,'SampleTime',-1,'Signal',struct('SgnName',{'VCUNRCDAlvRCHSC2','EPTTrInptShaftSpdHSC2','EPTTrInptShaftToqHSC2','EPTTrInptShaftSpdVHSC2','EPTTrInptShaftToqVHSC2'},'SgnStartBit',{8,16,32,61,62},'SgnLength',{4,16,12,1,1},'SgnType',{'standard','standard','standard','standard','standard'},'ModeValue',{-1,-1,-1,-1,-1},'DataType',{['unsigned int'],['unsigned int'],['unsigned int'],['unsigned int'],['unsigned int']},'ByteLayout',{['motorola back.'],['motorola back.'],['motorola back.'],['motorola back.'],['motorola back.']},'Factor',{1,1,2^-1,1,1},'Offset',{0,-32767,-848,0,0},'SLDataType',{'SS_DOUBLE','SS_DOUBLE','SS_DOUBLE','SS_DOUBLE','SS_DOUBLE'}),'StatusSelected','yes','TimeSelected','yes','DeltaTimeSelected','yes','BytePortSelected','no','MessageLengthSelected','no','TriggerPort',struct('Selected','no','TriggerType',0),'UserCoding',struct('Selected','no','InterfaceFile','UserDecodingFile','FcnName','UserDecodeFcn','InportSelected','no','InportWidth',1,'OutportSelected','no','OutportWidth',1),'EnablePortSelected','no','UseRXService','no','BoardType','DS1','BoardNo',1,'ControllerNo',1),'OFF',[]}},'TLCFileName',{{'rtican_rx_message','OFF',[]}})  RTISFcnParameters=struct('SFcnRTICANMessage','struct','TLCFileName','char')  RTIBlockParaDefault=struct('BoardTypeNo',4302,'BoardNo',1,'ChannelNo',1,'Parameters',struct('DataFileSupport',struct('DataFileSelectedMaster',0,'DataFileSelectedLocal',0,'DataFileName','','DataFileDate','','SelectedFile',['<no file selected>']),'Options',struct('StatusSelected',1,'TimeSelected',1,'DeltaTimeSelected',1,'BytePortSelected',0,'MessageLengthSelected',0,'TriggerPort',struct('Selected',0,'TriggerType','rising'),'UserCoding',struct('Selected',0,'InterfaceFile','UserDecodingFile','FcnName','UserDecodeFcn','InportSelected',0,'InportWidth',1,'OutportSelected',0,'OutportWidth',1),'EnablePortSelected',0,'SignalOnPortnameSelected',1,'UseRXService',0),'Message',struct('MsgOnBlocknameSelected',0,'MsgName',['RX Message'],'MsgIdFormat',0,'MsgId',100,'MsgLength',8,'NumSignals',1,'SampleTime',-1,'Signal',struct('SgnName',['RX signal'],'SgnStartBit',0,'SgnLength',8,'SgnType',0,'ModeValue',-1,'DataType',0,'SLDataType','SS_DOUBLE','ByteLayout',0,'Factor',1,'Offset',0,'Min',0,'Max',255,'SgnComment',{{}},'SgnUnit',''),'MsgIdNumFormat',0,'MsgComment',{{''}}),'Version',1.2,'general',struct('isFromLib',1)),'GroupId',struct('Group',{{'RTICAN'}},'No',1,'Behavior',{{'NAMECHANGE'}},'BlockType',{{'SINK'}},'NameChangeFlag',0),'SFcnRTICANMessage',struct('MsgType','RX','MsgName',['RX Message'],'MsgIdFormat','STD','MsgId',100,'MsgLength',8,'NumSignals',1,'SampleTime',-1,'Signal',struct('SgnName',['RX signal'],'SgnStartBit',0,'SgnLength',8,'SgnType','standard','ModeValue',-1,'DataType',['unsigned int'],'ByteLayout',['little endian'],'SLDataType','SS_DOUBLE','Factor',1,'Offset',0),'StatusSelected','yes','TimeSelected','yes','DeltaTimeSelected','yes','BytePortSelected','no','MessageLengthSelected','no','EnablePortSelected','no','UserCoding',struct('Selected','no','InterfaceFile','UserDecodingFile','FcnName','UserDecodeFcn','InportSelected','no','InportWidth',1,'OutportSelected','no','OutportWidth',1),'TriggerPort',struct('Selected','no','TriggerType','rising'),'UseRXService','no','BoardType','DS4302','BoardNo',1,'ControllerNo',1,'SFcnPortType','Scalar'),'TLCFileName','rtican_rx_message')
      settings: AttributesFormatString=Group Id: RTICAN1\n  SourceProductName=dSPACE RTI CAN Blockset
  SAS_HSC2_FrP00_0x1E5 : rtican/RTICAN Receive (RX)   Reserved1=[]  Reserved2=[]  Reserved3=[]  Reserved4=[]  SfcnMessage=[]  Msg_Struct=[]  BoardTypeNo=[]  BoardNo=[]  ChannelNo=[]  Parameters=[]  DialogFcn=[]  UnitName=[]  Revision=[]  UnitValues=[]  DSProperties=struct('RTI',struct('Version',uint32(5),'BlockType',struct('isSLSource',uint8(1),'isSLSink',uint8(1),'isHWSource',uint8(0),'isHWSink',uint8(0),'isSetup',uint8(0),'isInline',uint8(1),'isNonInline',uint8(0),'isInterrupt',uint8(0),'isChannelwise',uint8(0)),'IOBoardType','RTICAN','UnitType','MESSAGE','Identifier','RX','DialogType','MSVC','BlockSet','RTICAN','SlaveProcessor','CAN'))  RTIBlockInterface=struct('OutputPortsWidth',int32([1 1 1 1 1 1 1 1 1 1 1 1 1]),'OutputPortsActive',ones(1,13),'OutputPortsName',{{'StrgWhlAngSnsrChksmHSC2','StrgWhlAngExtdPVHSC2','StrgWhlAngGrdHSC2','StrgWhlAngAlvRCHSC2','StrgWhlAngHSC2','StrgWhlAngSnsrFltHSC2','StrgWhlAngSnsrMultCapbHSC2','StrgWhlAngSnsrInidHSC2','StrgWhlAngSnsrCalStsHSC2','StrgWhlAngVHSC2',['RX status'],['RX time'],['RX delta time']}},'OutputPortsDataType',{{'SS_DOUBLE','SS_DOUBLE','SS_DOUBLE','SS_DOUBLE','SS_DOUBLE','SS_DOUBLE','SS_DOUBLE','SS_DOUBLE','SS_DOUBLE','SS_DOUBLE','SS_DOUBLE','SS_DOUBLE','SS_DOUBLE'}},'OutputPortsLabel',{{'StrgWhlAngSnsrChksmHSC2','StrgWhlAngExtdPVHSC2','StrgWhlAngGrdHSC2','StrgWhlAngAlvRCHSC2','StrgWhlAngHSC2','StrgWhlAngSnsrFltHSC2','StrgWhlAngSnsrMultCapbHSC2','StrgWhlAngSnsrInidHSC2','StrgWhlAngSnsrCalStsHSC2','StrgWhlAngVHSC2','','',''}},'OutputPortsLabelMode','ON','InputPortsWidth',int32(0),'InputPortsActive',0,'DialogFcn','rtican_message_interface_gui','BlockDisplay',{{'','center'}},'IconTransparency','on','ParameterTunableNames',{{}},'InitLevel',3,'BlockName',struct('Token',{{'SAS_HSC2_FrP00'}}),'SampleTime',{{-1}},'TriggerPort',{{'none'}},'EnablePort',{{'none'}})  RTIBlockParameters=struct('BoardTypeNo',{{1,'OFF',[]}},'BoardNo',{{1,'ON',[1 16]}},'ChannelNo',{{1,'ON',[1 2]}},'Parameters',{{struct('DataFileSupport',struct('DataFileSelectedMaster',1,'DataFileSelectedLocal',1,'DataFileName','c:\users\linqi\desktop\matlab\acc\dbc\ep21_dbc\171114-lh1-ep21_ep2_fdr-_v07.dbc|','DataFileDate',['24-11月-2020 15:06:17'],'SelectedFile','..\..\dbc\ep21_dbc\171114-lh1-ep21_ep2_fdr-_v07_acc.dbc','InterfaceFcn','rtican_dbc_file_parser'),'Options',struct('StatusSelected',1,'TimeSelected',1,'DeltaTimeSelected',1,'BytePortSelected',0,'MessageLengthSelected',0,'TriggerPort',struct('Selected',0,'TriggerType',0),'UserCoding',struct('Selected',0,'InterfaceFile','UserDecodingFile','FcnName','UserDecodeFcn','InportSelected',0,'InportWidth',1,'OutportSelected',0,'OutportWidth',1),'EnablePortSelected',0,'SignalOnPortnameSelected',1,'UseRXService',0),'Message',struct('MsgOnBlocknameSelected',1,'MsgName','SAS_HSC2_FrP00','MsgIdFormat',0,'MsgId',485,'MsgLength',8,'NumSignals',10,'SampleTime',-1,'Signal',struct('SgnName',{'StrgWhlAngSnsrChksmHSC2','StrgWhlAngExtdPVHSC2','StrgWhlAngGrdHSC2','StrgWhlAngAlvRCHSC2','StrgWhlAngHSC2','StrgWhlAngSnsrFltHSC2','StrgWhlAngSnsrMultCapbHSC2','StrgWhlAngSnsrInidHSC2','StrgWhlAngSnsrCalStsHSC2','StrgWhlAngVHSC2'},'SgnStartBit',{0,8,24,36,40,56,57,58,61,63},'SgnLength',{8,16,12,4,16,1,1,1,2,1},'ByteLayout',{2,2,2,2,2,2,2,2,2,2},'Factor',{1,1,1,1,2^-4,1,1,1,1,1},'Offset',{0,0,-2048,0,-2048,0,0,0,0,0},'SgnComment',{'','','','','','','','','',''},'SgnUnit',{'','','degree/s','','degree','','','','',''},'Min',{0,0,-2048,0,-2048,0,0,0,0,0},'Max',{255,65535,2046,15,2047.88,1,1,1,3,1},'SgnType',{0,0,0,0,0,0,0,0,0,0},'SLDataType',{'SS_DOUBLE','SS_DOUBLE','SS_DOUBLE','SS_DOUBLE','SS_DOUBLE','SS_DOUBLE','SS_DOUBLE','SS_DOUBLE','SS_DOUBLE','SS_DOUBLE'},'DataType',{0,0,0,0,0,0,0,0,0,0},'ModeValue',{-1,-1,-1,-1,-1,-1,-1,-1,-1,-1}),'MsgIdNumFormat',0,'MsgComment',{{''}}),'Version',1.2,'general',struct('isFromLib',0)),'OFF',[]}},'GroupId',{{struct('Group',{{'RTICAN'}},'No',1,'Behavior',{{'NAMECHANGE'}},'BlockType',{{'SINK'}},'NameChangeFlag',0),'OFF',[]}},'SFcnRTICANMessage',{{struct('MsgType','RX','SFcnPortType','Scalar','MsgName','SAS_HSC2_FrP00','MsgIdFormat','STD','MsgId',485,'MsgLength',8,'NumSignals',10,'SampleTime',-1,'Signal',struct('SgnName',{'StrgWhlAngSnsrChksmHSC2','StrgWhlAngExtdPVHSC2','StrgWhlAngGrdHSC2','StrgWhlAngAlvRCHSC2','StrgWhlAngHSC2','StrgWhlAngSnsrFltHSC2','StrgWhlAngSnsrMultCapbHSC2','StrgWhlAngSnsrInidHSC2','StrgWhlAngSnsrCalStsHSC2','StrgWhlAngVHSC2'},'SgnStartBit',{0,8,24,36,40,56,57,58,61,63},'SgnLength',{8,16,12,4,16,1,1,1,2,1},'ByteLayout',{['motorola back.'],['motorola back.'],['motorola back.'],['motorola back.'],['motorola back.'],['motorola back.'],['motorola back.'],['motorola back.'],['motorola back.'],['motorola back.']},'Factor',{1,1,1,1,2^-4,1,1,1,1,1},'Offset',{0,0,-2048,0,-2048,0,0,0,0,0},'SgnType',{'standard','standard','standard','standard','standard','standard','standard','standard','standard','standard'},'SLDataType',{'SS_DOUBLE','SS_DOUBLE','SS_DOUBLE','SS_DOUBLE','SS_DOUBLE','SS_DOUBLE','SS_DOUBLE','SS_DOUBLE','SS_DOUBLE','SS_DOUBLE'},'DataType',{['unsigned int'],['unsigned int'],['unsigned int'],['unsigned int'],['unsigned int'],['unsigned int'],['unsigned int'],['unsigned int'],['unsigned int'],['unsigned int']},'ModeValue',{-1,-1,-1,-1,-1,-1,-1,-1,-1,-1}),'StatusSelected','yes','TimeSelected','yes','DeltaTimeSelected','yes','BytePortSelected','no','MessageLengthSelected','no','TriggerPort',struct('Selected','no','TriggerType',0),'UserCoding',struct('Selected','no','InterfaceFile','UserDecodingFile','FcnName','UserDecodeFcn','InportSelected','no','InportWidth',1,'OutportSelected','no','OutportWidth',1),'EnablePortSelected','no','UseRXService','no','BoardType','DS1','BoardNo',1,'ControllerNo',1),'OFF',[]}},'TLCFileName',{{'rtican_rx_message','OFF',[]}})  RTISFcnParameters=struct('SFcnRTICANMessage','struct','TLCFileName','char')  RTIBlockParaDefault=struct('BoardTypeNo',4302,'BoardNo',1,'ChannelNo',1,'Parameters',struct('DataFileSupport',struct('DataFileSelectedMaster',0,'DataFileSelectedLocal',0,'DataFileName','','DataFileDate','','SelectedFile',['<no file selected>']),'Options',struct('StatusSelected',1,'TimeSelected',1,'DeltaTimeSelected',1,'BytePortSelected',0,'MessageLengthSelected',0,'TriggerPort',struct('Selected',0,'TriggerType','rising'),'UserCoding',struct('Selected',0,'InterfaceFile','UserDecodingFile','FcnName','UserDecodeFcn','InportSelected',0,'InportWidth',1,'OutportSelected',0,'OutportWidth',1),'EnablePortSelected',0,'SignalOnPortnameSelected',1,'UseRXService',0),'Message',struct('MsgOnBlocknameSelected',0,'MsgName',['RX Message'],'MsgIdFormat',0,'MsgId',100,'MsgLength',8,'NumSignals',1,'SampleTime',-1,'Signal',struct('SgnName',['RX signal'],'SgnStartBit',0,'SgnLength',8,'SgnType',0,'ModeValue',-1,'DataType',0,'SLDataType','SS_DOUBLE','ByteLayout',0,'Factor',1,'Offset',0,'Min',0,'Max',255,'SgnComment',{{}},'SgnUnit',''),'MsgIdNumFormat',0,'MsgComment',{{''}}),'Version',1.2,'general',struct('isFromLib',1)),'GroupId',struct('Group',{{'RTICAN'}},'No',1,'Behavior',{{'NAMECHANGE'}},'BlockType',{{'SINK'}},'NameChangeFlag',0),'SFcnRTICANMessage',struct('MsgType','RX','MsgName',['RX Message'],'MsgIdFormat','STD','MsgId',100,'MsgLength',8,'NumSignals',1,'SampleTime',-1,'Signal',struct('SgnName',['RX signal'],'SgnStartBit',0,'SgnLength',8,'SgnType','standard','ModeValue',-1,'DataType',['unsigned int'],'ByteLayout',['little endian'],'SLDataType','SS_DOUBLE','Factor',1,'Offset',0),'StatusSelected','yes','TimeSelected','yes','DeltaTimeSelected','yes','BytePortSelected','no','MessageLengthSelected','no','EnablePortSelected','no','UserCoding',struct('Selected','no','InterfaceFile','UserDecodingFile','FcnName','UserDecodeFcn','InportSelected','no','InportWidth',1,'OutportSelected','no','OutportWidth',1),'TriggerPort',struct('Selected','no','TriggerType','rising'),'UseRXService','no','BoardType','DS4302','BoardNo',1,'ControllerNo',1,'SFcnPortType','Scalar'),'TLCFileName','rtican_rx_message')
      settings: AttributesFormatString=Group Id: RTICAN1\n  SourceProductName=dSPACE RTI CAN Blockset
  SCS_HSC2_FrP02_0x185 : rtican/RTICAN Receive (RX)   Reserved1=[]  Reserved2=[]  Reserved3=[]  Reserved4=[]  SfcnMessage=[]  Msg_Struct=[]  BoardTypeNo=[]  BoardNo=[]  ChannelNo=[]  Parameters=[]  DialogFcn=[]  UnitName=[]  Revision=[]  UnitValues=[]  DSProperties=struct('RTI',struct('Version',uint32(5),'BlockType',struct('isSLSource',uint8(1),'isSLSink',uint8(1),'isHWSource',uint8(0),'isHWSink',uint8(0),'isSetup',uint8(0),'isInline',uint8(1),'isNonInline',uint8(0),'isInterrupt',uint8(0),'isChannelwise',uint8(0)),'IOBoardType','RTICAN','UnitType','MESSAGE','Identifier','RX','DialogType','MSVC','BlockSet','RTICAN','SlaveProcessor','CAN'))  RTIBlockInterface=struct('OutputPortsWidth',int32([1 1 1 1 1 1 1]),'OutputPortsActive',[1 1 1 1 1 1 1],'OutputPortsName',{{'VSELatAccHSC2','VSELongtAccHSC2','VSELongtAccVHSC2','VSELatAccVHSC2',['RX status'],['RX time'],['RX delta time']}},'OutputPortsDataType',{{'SS_DOUBLE','SS_DOUBLE','SS_DOUBLE','SS_DOUBLE','SS_DOUBLE','SS_DOUBLE','SS_DOUBLE'}},'OutputPortsLabel',{{'VSELatAccHSC2','VSELongtAccHSC2','VSELongtAccVHSC2','VSELatAccVHSC2','','',''}},'OutputPortsLabelMode','ON','InputPortsWidth',int32(0),'InputPortsActive',0,'DialogFcn','rtican_message_interface_gui','BlockDisplay',{{'','center'}},'IconTransparency','on','ParameterTunableNames',{{}},'InitLevel',3,'BlockName',struct('Token',{{'SCS_HSC2_FrP02'}}),'SampleTime',{{-1}},'TriggerPort',{{'none'}},'EnablePort',{{'none'}})  RTIBlockParameters=struct('BoardTypeNo',{{1,'OFF',[]}},'BoardNo',{{1,'ON',[1 16]}},'ChannelNo',{{1,'ON',[1 2]}},'Parameters',{{struct('DataFileSupport',struct('DataFileSelectedMaster',1,'DataFileSelectedLocal',1,'DataFileName','c:\users\linqi\desktop\matlab\acc\dbc\ep21_dbc\171114-lh1-ep21_ep2_fdr-_v07.dbc|','DataFileDate',['24-11月-2020 15:06:17'],'SelectedFile','..\..\dbc\ep21_dbc\171114-lh1-ep21_ep2_fdr-_v07_acc.dbc','InterfaceFcn','rtican_dbc_file_parser'),'Options',struct('StatusSelected',1,'TimeSelected',1,'DeltaTimeSelected',1,'BytePortSelected',0,'MessageLengthSelected',0,'TriggerPort',struct('Selected',0,'TriggerType',0),'UserCoding',struct('Selected',0,'InterfaceFile','UserDecodingFile','FcnName','UserDecodeFcn','InportSelected',0,'InportWidth',1,'OutportSelected',0,'OutportWidth',1),'EnablePortSelected',0,'SignalOnPortnameSelected',1,'UseRXService',0),'Message',struct('MsgOnBlocknameSelected',1,'MsgName','SCS_HSC2_FrP02','MsgIdFormat',0,'MsgId',389,'MsgLength',4,'NumSignals',4,'SampleTime',-1,'Signal',struct('SgnName',{'VSELatAccHSC2','VSELongtAccHSC2','VSELongtAccVHSC2','VSELatAccVHSC2'},'SgnStartBit',{0,16,26,27},'SgnLength',{12,10,1,1},'ByteLayout',{2,2,2,2},'Factor',{2^-6,0.03,1,1},'Offset',{0,0,0,0},'SgnComment',{'','','',''},'SgnUnit',{'m/s^2','m/s^2','',''},'Min',{-32,-15.36,0,0},'Max',{31.9844,15.33,1,1},'SgnType',{0,0,0,0},'SLDataType',{'SS_DOUBLE','SS_DOUBLE','SS_DOUBLE','SS_DOUBLE'},'DataType',{1,1,0,0},'ModeValue',{-1,-1,-1,-1}),'MsgIdNumFormat',0,'MsgComment',{{''}}),'Version',1.2,'general',struct('isFromLib',0)),'OFF',[]}},'GroupId',{{struct('Group',{{'RTICAN'}},'No',1,'Behavior',{{'NAMECHANGE'}},'BlockType',{{'SINK'}},'NameChangeFlag',0),'OFF',[]}},'SFcnRTICANMessage',{{struct('MsgType','RX','SFcnPortType','Scalar','MsgName','SCS_HSC2_FrP02','MsgIdFormat','STD','MsgId',389,'MsgLength',4,'NumSignals',4,'SampleTime',-1,'Signal',struct('SgnName',{'VSELatAccHSC2','VSELongtAccHSC2','VSELongtAccVHSC2','VSELatAccVHSC2'},'SgnStartBit',{0,16,26,27},'SgnLength',{12,10,1,1},'ByteLayout',{['motorola back.'],['motorola back.'],['motorola back.'],['motorola back.']},'Factor',{2^-6,0.03,1,1},'Offset',{0,0,0,0},'SgnType',{'standard','standard','standard','standard'},'SLDataType',{'SS_DOUBLE','SS_DOUBLE','SS_DOUBLE','SS_DOUBLE'},'DataType',{['signed int'],['signed int'],['unsigned int'],['unsigned int']},'ModeValue',{-1,-1,-1,-1}),'StatusSelected','yes','TimeSelected','yes','DeltaTimeSelected','yes','BytePortSelected','no','MessageLengthSelected','no','TriggerPort',struct('Selected','no','TriggerType',0),'UserCoding',struct('Selected','no','InterfaceFile','UserDecodingFile','FcnName','UserDecodeFcn','InportSelected','no','InportWidth',1,'OutportSelected','no','OutportWidth',1),'EnablePortSelected','no','UseRXService','no','BoardType','DS1','BoardNo',1,'ControllerNo',1),'OFF',[]}},'TLCFileName',{{'rtican_rx_message','OFF',[]}})  RTISFcnParameters=struct('SFcnRTICANMessage','struct','TLCFileName','char')  RTIBlockParaDefault=struct('BoardTypeNo',4302,'BoardNo',1,'ChannelNo',1,'Parameters',struct('DataFileSupport',struct('DataFileSelectedMaster',0,'DataFileSelectedLocal',0,'DataFileName','','DataFileDate','','SelectedFile',['<no file selected>']),'Options',struct('StatusSelected',1,'TimeSelected',1,'DeltaTimeSelected',1,'BytePortSelected',0,'MessageLengthSelected',0,'TriggerPort',struct('Selected',0,'TriggerType','rising'),'UserCoding',struct('Selected',0,'InterfaceFile','UserDecodingFile','FcnName','UserDecodeFcn','InportSelected',0,'InportWidth',1,'OutportSelected',0,'OutportWidth',1),'EnablePortSelected',0,'SignalOnPortnameSelected',1,'UseRXService',0),'Message',struct('MsgOnBlocknameSelected',0,'MsgName',['RX Message'],'MsgIdFormat',0,'MsgId',100,'MsgLength',8,'NumSignals',1,'SampleTime',-1,'Signal',struct('SgnName',['RX signal'],'SgnStartBit',0,'SgnLength',8,'SgnType',0,'ModeValue',-1,'DataType',0,'SLDataType','SS_DOUBLE','ByteLayout',0,'Factor',1,'Offset',0,'Min',0,'Max',255,'SgnComment',{{}},'SgnUnit',''),'MsgIdNumFormat',0,'MsgComment',{{''}}),'Version',1.2,'general',struct('isFromLib',1)),'GroupId',struct('Group',{{'RTICAN'}},'No',1,'Behavior',{{'NAMECHANGE'}},'BlockType',{{'SINK'}},'NameChangeFlag',0),'SFcnRTICANMessage',struct('MsgType','RX','MsgName',['RX Message'],'MsgIdFormat','STD','MsgId',100,'MsgLength',8,'NumSignals',1,'SampleTime',-1,'Signal',struct('SgnName',['RX signal'],'SgnStartBit',0,'SgnLength',8,'SgnType','standard','ModeValue',-1,'DataType',['unsigned int'],'ByteLayout',['little endian'],'SLDataType','SS_DOUBLE','Factor',1,'Offset',0),'StatusSelected','yes','TimeSelected','yes','DeltaTimeSelected','yes','BytePortSelected','no','MessageLengthSelected','no','EnablePortSelected','no','UserCoding',struct('Selected','no','InterfaceFile','UserDecodingFile','FcnName','UserDecodeFcn','InportSelected','no','InportWidth',1,'OutportSelected','no','OutportWidth',1),'TriggerPort',struct('Selected','no','TriggerType','rising'),'UseRXService','no','BoardType','DS4302','BoardNo',1,'ControllerNo',1,'SFcnPortType','Scalar'),'TLCFileName','rtican_rx_message')
      settings: AttributesFormatString=Group Id: RTICAN1\n  SourceProductName=dSPACE RTI CAN Blockset
  SCS_HSC2_FrP05_0x1E9 : rtican/RTICAN Receive (RX)   Reserved1=[]  Reserved2=[]  Reserved3=[]  Reserved4=[]  SfcnMessage=[]  Msg_Struct=[]  BoardTypeNo=[]  BoardNo=[]  ChannelNo=[]  Parameters=[]  DialogFcn=[]  UnitName=[]  Revision=[]  UnitValues=[]  DSProperties=struct('RTI',struct('Version',uint32(5),'BlockType',struct('isSLSource',uint8(1),'isSLSink',uint8(1),'isHWSource',uint8(0),'isHWSink',uint8(0),'isSetup',uint8(0),'isInline',uint8(1),'isNonInline',uint8(0),'isInterrupt',uint8(0),'isChannelwise',uint8(0)),'IOBoardType','RTICAN','UnitType','MESSAGE','Identifier','RX','DialogType','MSVC','BlockSet','RTICAN','SlaveProcessor','CAN'))  RTIBlockInterface=struct('OutputPortsWidth',int32([1 1 1 1 1 1 1]),'OutputPortsActive',[1 1 1 1 1 1 1],'OutputPortsName',{{'VehDynYawRateHSC2','VehDynYawRateVHSC2','EnDragToqRducnAHSC2','ABSAHSC2',['RX status'],['RX time'],['RX delta time']}},'OutputPortsDataType',{{'SS_DOUBLE','SS_DOUBLE','SS_DOUBLE','SS_DOUBLE','SS_DOUBLE','SS_DOUBLE','SS_DOUBLE'}},'OutputPortsLabel',{{'VehDynYawRateHSC2','VehDynYawRateVHSC2','EnDragToqRducnAHSC2','ABSAHSC2','','',''}},'OutputPortsLabelMode','ON','InputPortsWidth',int32(0),'InputPortsActive',0,'DialogFcn','rtican_message_interface_gui','BlockDisplay',{{'','center'}},'IconTransparency','on','ParameterTunableNames',{{}},'InitLevel',3,'BlockName',struct('Token',{{'SCS_HSC2_FrP05'}}),'SampleTime',{{-1}},'TriggerPort',{{'none'}},'EnablePort',{{'none'}})  RTIBlockParameters=struct('BoardTypeNo',{{1,'OFF',[]}},'BoardNo',{{1,'ON',[1 16]}},'ChannelNo',{{1,'ON',[1 2]}},'Parameters',{{struct('DataFileSupport',struct('DataFileSelectedMaster',1,'DataFileSelectedLocal',1,'DataFileName','c:\users\linqi\desktop\matlab\acc\dbc\ep21_dbc\171114-lh1-ep21_ep2_fdr-_v07.dbc|','DataFileDate',['24-11月-2020 15:06:17'],'SelectedFile','..\..\dbc\ep21_dbc\171114-lh1-ep21_ep2_fdr-_v07_acc.dbc','InterfaceFcn','rtican_dbc_file_parser'),'Options',struct('StatusSelected',1,'TimeSelected',1,'DeltaTimeSelected',1,'BytePortSelected',0,'MessageLengthSelected',0,'TriggerPort',struct('Selected',0,'TriggerType',0),'UserCoding',struct('Selected',0,'InterfaceFile','UserDecodingFile','FcnName','UserDecodeFcn','InportSelected',0,'InportWidth',1,'OutportSelected',0,'OutportWidth',1),'EnablePortSelected',0,'SignalOnPortnameSelected',1,'UseRXService',0),'Message',struct('MsgOnBlocknameSelected',1,'MsgName','SCS_HSC2_FrP05','MsgIdFormat',0,'MsgId',489,'MsgLength',8,'NumSignals',4,'SampleTime',-1,'Signal',struct('SgnName',{'VehDynYawRateHSC2','VehDynYawRateVHSC2','EnDragToqRducnAHSC2','ABSAHSC2'},'SgnStartBit',{16,28,33,38},'SgnLength',{12,1,1,1},'ByteLayout',{2,2,2,2},'Factor',{2^-4,1,1,1},'Offset',{0,0,0,0},'SgnComment',{'','',['Engine Drag Torque Reduction Active' char(10) ''],''},'SgnUnit',{'deg/s','','',''},'Min',{-128,0,0,0},'Max',{127.938,1,1,1},'SgnType',{0,0,0,0},'SLDataType',{'SS_DOUBLE','SS_DOUBLE','SS_DOUBLE','SS_DOUBLE'},'DataType',{1,0,0,0},'ModeValue',{-1,-1,-1,-1}),'MsgIdNumFormat',0,'MsgComment',{{''}}),'Version',1.2,'general',struct('isFromLib',0)),'OFF',[]}},'GroupId',{{struct('Group',{{'RTICAN'}},'No',1,'Behavior',{{'NAMECHANGE'}},'BlockType',{{'SINK'}},'NameChangeFlag',0),'OFF',[]}},'SFcnRTICANMessage',{{struct('MsgType','RX','SFcnPortType','Scalar','MsgName','SCS_HSC2_FrP05','MsgIdFormat','STD','MsgId',489,'MsgLength',8,'NumSignals',4,'SampleTime',-1,'Signal',struct('SgnName',{'VehDynYawRateHSC2','VehDynYawRateVHSC2','EnDragToqRducnAHSC2','ABSAHSC2'},'SgnStartBit',{16,28,33,38},'SgnLength',{12,1,1,1},'ByteLayout',{['motorola back.'],['motorola back.'],['motorola back.'],['motorola back.']},'Factor',{2^-4,1,1,1},'Offset',{0,0,0,0},'SgnType',{'standard','standard','standard','standard'},'SLDataType',{'SS_DOUBLE','SS_DOUBLE','SS_DOUBLE','SS_DOUBLE'},'DataType',{['signed int'],['unsigned int'],['unsigned int'],['unsigned int']},'ModeValue',{-1,-1,-1,-1}),'StatusSelected','yes','TimeSelected','yes','DeltaTimeSelected','yes','BytePortSelected','no','MessageLengthSelected','no','TriggerPort',struct('Selected','no','TriggerType',0),'UserCoding',struct('Selected','no','InterfaceFile','UserDecodingFile','FcnName','UserDecodeFcn','InportSelected','no','InportWidth',1,'OutportSelected','no','OutportWidth',1),'EnablePortSelected','no','UseRXService','no','BoardType','DS1','BoardNo',1,'ControllerNo',1),'OFF',[]}},'TLCFileName',{{'rtican_rx_message','OFF',[]}})  RTISFcnParameters=struct('SFcnRTICANMessage','struct','TLCFileName','char')  RTIBlockParaDefault=struct('BoardTypeNo',4302,'BoardNo',1,'ChannelNo',1,'Parameters',struct('DataFileSupport',struct('DataFileSelectedMaster',0,'DataFileSelectedLocal',0,'DataFileName','','DataFileDate','','SelectedFile',['<no file selected>']),'Options',struct('StatusSelected',1,'TimeSelected',1,'DeltaTimeSelected',1,'BytePortSelected',0,'MessageLengthSelected',0,'TriggerPort',struct('Selected',0,'TriggerType','rising'),'UserCoding',struct('Selected',0,'InterfaceFile','UserDecodingFile','FcnName','UserDecodeFcn','InportSelected',0,'InportWidth',1,'OutportSelected',0,'OutportWidth',1),'EnablePortSelected',0,'SignalOnPortnameSelected',1,'UseRXService',0),'Message',struct('MsgOnBlocknameSelected',0,'MsgName',['RX Message'],'MsgIdFormat',0,'MsgId',100,'MsgLength',8,'NumSignals',1,'SampleTime',-1,'Signal',struct('SgnName',['RX signal'],'SgnStartBit',0,'SgnLength',8,'SgnType',0,'ModeValue',-1,'DataType',0,'SLDataType','SS_DOUBLE','ByteLayout',0,'Factor',1,'Offset',0,'Min',0,'Max',255,'SgnComment',{{}},'SgnUnit',''),'MsgIdNumFormat',0,'MsgComment',{{''}}),'Version',1.2,'general',struct('isFromLib',1)),'GroupId',struct('Group',{{'RTICAN'}},'No',1,'Behavior',{{'NAMECHANGE'}},'BlockType',{{'SINK'}},'NameChangeFlag',0),'SFcnRTICANMessage',struct('MsgType','RX','MsgName',['RX Message'],'MsgIdFormat','STD','MsgId',100,'MsgLength',8,'NumSignals',1,'SampleTime',-1,'Signal',struct('SgnName',['RX signal'],'SgnStartBit',0,'SgnLength',8,'SgnType','standard','ModeValue',-1,'DataType',['unsigned int'],'ByteLayout',['little endian'],'SLDataType','SS_DOUBLE','Factor',1,'Offset',0),'StatusSelected','yes','TimeSelected','yes','DeltaTimeSelected','yes','BytePortSelected','no','MessageLengthSelected','no','EnablePortSelected','no','UserCoding',struct('Selected','no','InterfaceFile','UserDecodingFile','FcnName','UserDecodeFcn','InportSelected','no','InportWidth',1,'OutportSelected','no','OutportWidth',1),'TriggerPort',struct('Selected','no','TriggerType','rising'),'UseRXService','no','BoardType','DS4302','BoardNo',1,'ControllerNo',1,'SFcnPortType','Scalar'),'TLCFileName','rtican_rx_message')
      settings: AttributesFormatString=Group Id: RTICAN1\n  SourceProductName=dSPACE RTI CAN Blockset
  SCS_HSC2_FrP19_0x23C : rtican/RTICAN Receive (RX)   Reserved1=[]  Reserved2=[]  Reserved3=[]  Reserved4=[]  SfcnMessage=[]  Msg_Struct=[]  BoardTypeNo=[]  BoardNo=[]  ChannelNo=[]  Parameters=[]  DialogFcn=[]  UnitName=[]  Revision=[]  UnitValues=[]  DSProperties=struct('RTI',struct('Version',uint32(5),'BlockType',struct('isSLSource',uint8(1),'isSLSink',uint8(1),'isHWSource',uint8(0),'isHWSink',uint8(0),'isSetup',uint8(0),'isInline',uint8(1),'isNonInline',uint8(0),'isInterrupt',uint8(0),'isChannelwise',uint8(0)),'IOBoardType','RTICAN','UnitType','MESSAGE','Identifier','RX','DialogType','MSVC','BlockSet','RTICAN','SlaveProcessor','CAN'))  RTIBlockInterface=struct('OutputPortsWidth',int32([1 1 1 1 1 1 1]),'OutputPortsActive',[1 1 1 1 1 1 1],'OutputPortsName',{{'VehSpdAvgAlvRCHSC2','VehSpdAvgHSC2','VehSpdAvgVHSC2','VehSpdAvgPVHSC2',['RX status'],['RX time'],['RX delta time']}},'OutputPortsDataType',{{'SS_DOUBLE','SS_DOUBLE','SS_DOUBLE','SS_DOUBLE','SS_DOUBLE','SS_DOUBLE','SS_DOUBLE'}},'OutputPortsLabel',{{'VehSpdAvgAlvRCHSC2','VehSpdAvgHSC2','VehSpdAvgVHSC2','VehSpdAvgPVHSC2','','',''}},'OutputPortsLabelMode','ON','InputPortsWidth',int32(0),'InputPortsActive',0,'DialogFcn','rtican_message_interface_gui','BlockDisplay',{{'','center'}},'IconTransparency','on','ParameterTunableNames',{{}},'InitLevel',3,'BlockName',struct('Token',{{'SCS_HSC2_FrP19'}}),'SampleTime',{{-1}},'TriggerPort',{{'none'}},'EnablePort',{{'none'}})  RTIBlockParameters=struct('BoardTypeNo',{{1,'OFF',[]}},'BoardNo',{{1,'ON',[1 16]}},'ChannelNo',{{1,'ON',[1 2]}},'Parameters',{{struct('DataFileSupport',struct('DataFileSelectedMaster',1,'DataFileSelectedLocal',1,'DataFileName','c:\users\linqi\desktop\matlab\acc\dbc\ep21_dbc\171114-lh1-ep21_ep2_fdr-_v07.dbc|','DataFileDate',['24-11月-2020 15:06:17'],'SelectedFile','..\..\dbc\ep21_dbc\171114-lh1-ep21_ep2_fdr-_v07_acc.dbc','InterfaceFcn','rtican_dbc_file_parser'),'Options',struct('StatusSelected',1,'TimeSelected',1,'DeltaTimeSelected',1,'BytePortSelected',0,'MessageLengthSelected',0,'TriggerPort',struct('Selected',0,'TriggerType',0),'UserCoding',struct('Selected',0,'InterfaceFile','UserDecodingFile','FcnName','UserDecodeFcn','InportSelected',0,'InportWidth',1,'OutportSelected',0,'OutportWidth',1),'EnablePortSelected',0,'SignalOnPortnameSelected',1,'UseRXService',0),'Message',struct('MsgOnBlocknameSelected',1,'MsgName','SCS_HSC2_FrP19','MsgIdFormat',0,'MsgId',572,'MsgLength',8,'NumSignals',4,'SampleTime',-1,'Signal',struct('SgnName',{'VehSpdAvgAlvRCHSC2','VehSpdAvgHSC2','VehSpdAvgVHSC2','VehSpdAvgPVHSC2'},'SgnStartBit',{28,32,47,48},'SgnLength',{4,15,1,16},'ByteLayout',{2,2,2,2},'Factor',{1,2^-6,1,1},'Offset',{0,0,0,0},'SgnComment',{'','','',''},'SgnUnit',{'','km/h','',''},'Min',{0,0,0,0},'Max',{15,511.984,1,65535},'SgnType',{0,0,0,0},'SLDataType',{'SS_DOUBLE','SS_DOUBLE','SS_DOUBLE','SS_DOUBLE'},'DataType',{0,0,0,0},'ModeValue',{-1,-1,-1,-1}),'MsgIdNumFormat',0,'MsgComment',{{''}}),'Version',1.2,'general',struct('isFromLib',0)),'OFF',[]}},'GroupId',{{struct('Group',{{'RTICAN'}},'No',1,'Behavior',{{'NAMECHANGE'}},'BlockType',{{'SINK'}},'NameChangeFlag',0),'OFF',[]}},'SFcnRTICANMessage',{{struct('MsgType','RX','SFcnPortType','Scalar','MsgName','SCS_HSC2_FrP19','MsgIdFormat','STD','MsgId',572,'MsgLength',8,'NumSignals',4,'SampleTime',-1,'Signal',struct('SgnName',{'VehSpdAvgAlvRCHSC2','VehSpdAvgHSC2','VehSpdAvgVHSC2','VehSpdAvgPVHSC2'},'SgnStartBit',{28,32,47,48},'SgnLength',{4,15,1,16},'ByteLayout',{['motorola back.'],['motorola back.'],['motorola back.'],['motorola back.']},'Factor',{1,2^-6,1,1},'Offset',{0,0,0,0},'SgnType',{'standard','standard','standard','standard'},'SLDataType',{'SS_DOUBLE','SS_DOUBLE','SS_DOUBLE','SS_DOUBLE'},'DataType',{['unsigned int'],['unsigned int'],['unsigned int'],['unsigned int']},'ModeValue',{-1,-1,-1,-1}),'StatusSelected','yes','TimeSelected','yes','DeltaTimeSelected','yes','BytePortSelected','no','MessageLengthSelected','no','TriggerPort',struct('Selected','no','TriggerType',0),'UserCoding',struct('Selected','no','InterfaceFile','UserDecodingFile','FcnName','UserDecodeFcn','InportSelected','no','InportWidth',1,'OutportSelected','no','OutportWidth',1),'EnablePortSelected','no','UseRXService','no','BoardType','DS1','BoardNo',1,'ControllerNo',1),'OFF',[]}},'TLCFileName',{{'rtican_rx_message','OFF',[]}})  RTISFcnParameters=struct('SFcnRTICANMessage','struct','TLCFileName','char')  RTIBlockParaDefault=struct('BoardTypeNo',4302,'BoardNo',1,'ChannelNo',1,'Parameters',struct('DataFileSupport',struct('DataFileSelectedMaster',0,'DataFileSelectedLocal',0,'DataFileName','','DataFileDate','','SelectedFile',['<no file selected>']),'Options',struct('StatusSelected',1,'TimeSelected',1,'DeltaTimeSelected',1,'BytePortSelected',0,'MessageLengthSelected',0,'TriggerPort',struct('Selected',0,'TriggerType','rising'),'UserCoding',struct('Selected',0,'InterfaceFile','UserDecodingFile','FcnName','UserDecodeFcn','InportSelected',0,'InportWidth',1,'OutportSelected',0,'OutportWidth',1),'EnablePortSelected',0,'SignalOnPortnameSelected',1,'UseRXService',0),'Message',struct('MsgOnBlocknameSelected',0,'MsgName',['RX Message'],'MsgIdFormat',0,'MsgId',100,'MsgLength',8,'NumSignals',1,'SampleTime',-1,'Signal',struct('SgnName',['RX signal'],'SgnStartBit',0,'SgnLength',8,'SgnType',0,'ModeValue',-1,'DataType',0,'SLDataType','SS_DOUBLE','ByteLayout',0,'Factor',1,'Offset',0,'Min',0,'Max',255,'SgnComment',{{}},'SgnUnit',''),'MsgIdNumFormat',0,'MsgComment',{{''}}),'Version',1.2,'general',struct('isFromLib',1)),'GroupId',struct('Group',{{'RTICAN'}},'No',1,'Behavior',{{'NAMECHANGE'}},'BlockType',{{'SINK'}},'NameChangeFlag',0),'SFcnRTICANMessage',struct('MsgType','RX','MsgName',['RX Message'],'MsgIdFormat','STD','MsgId',100,'MsgLength',8,'NumSignals',1,'SampleTime',-1,'Signal',struct('SgnName',['RX signal'],'SgnStartBit',0,'SgnLength',8,'SgnType','standard','ModeValue',-1,'DataType',['unsigned int'],'ByteLayout',['little endian'],'SLDataType','SS_DOUBLE','Factor',1,'Offset',0),'StatusSelected','yes','TimeSelected','yes','DeltaTimeSelected','yes','BytePortSelected','no','MessageLengthSelected','no','EnablePortSelected','no','UserCoding',struct('Selected','no','InterfaceFile','UserDecodingFile','FcnName','UserDecodeFcn','InportSelected','no','InportWidth',1,'OutportSelected','no','OutportWidth',1),'TriggerPort',struct('Selected','no','TriggerType','rising'),'UseRXService','no','BoardType','DS4302','BoardNo',1,'ControllerNo',1,'SFcnPortType','Scalar'),'TLCFileName','rtican_rx_message')
      settings: AttributesFormatString=Group Id: RTICAN1\n  SourceProductName=dSPACE RTI CAN Blockset
  SCS_HSC2_FrP22_0x24C : rtican/RTICAN Receive (RX)   Reserved1=[]  Reserved2=[]  Reserved3=[]  Reserved4=[]  SfcnMessage=[]  Msg_Struct=[]  BoardTypeNo=[]  BoardNo=[]  ChannelNo=[]  Parameters=[]  DialogFcn=[]  UnitName=[]  Revision=[]  UnitValues=[]  DSProperties=struct('RTI',struct('Version',uint32(5),'BlockType',struct('isSLSource',uint8(1),'isSLSink',uint8(1),'isHWSource',uint8(0),'isHWSink',uint8(0),'isSetup',uint8(0),'isInline',uint8(1),'isNonInline',uint8(0),'isInterrupt',uint8(0),'isChannelwise',uint8(0)),'IOBoardType','RTICAN','UnitType','MESSAGE','Identifier','RX','DialogType','MSVC','BlockSet','RTICAN','SlaveProcessor','CAN'))  RTIBlockInterface=struct('OutputPortsWidth',int32([1 1 1 1 1 1 1 1 1 1 1 1 1 1 1 1]),'OutputPortsActive',ones(1,16),'OutputPortsName',{{'WhlGndVelDrvnChksm_RadarHSC2','WhlGndVelLDrvn_RadarHSC2','WhlGndVelRDrvn_RadarHSC2','BrkPdlDrvrAppdPrs_RadarHSC2','WhlGndVelDrvnRC_RadarHSC2','BrkPdlDrvrAppdPrsAlvRC_RadarHSC2','LDrvnWhlRotlDircnHSC2','RDrvnWhlRotlDircnHSC2','WhlGndVelLDrvnV_RadarHSC2','WhlGndVelRDrvnV_RadarHSC2','WhlBrkPrsStsHSC2','BrkDiscTemStsHSC2','BrkPdlDrvrAppdPrsV_RadarHSC2',['RX status'],['RX time'],['RX delta time']}},'OutputPortsDataType',{{'SS_DOUBLE','SS_DOUBLE','SS_DOUBLE','SS_DOUBLE','SS_DOUBLE','SS_DOUBLE','SS_DOUBLE','SS_DOUBLE','SS_DOUBLE','SS_DOUBLE','SS_DOUBLE','SS_DOUBLE','SS_DOUBLE','SS_DOUBLE','SS_DOUBLE','SS_DOUBLE'}},'OutputPortsLabel',{{'WhlGndVelDrvnChksm_RadarHSC2','WhlGndVelLDrvn_RadarHSC2','WhlGndVelRDrvn_RadarHSC2','BrkPdlDrvrAppdPrs_RadarHSC2','WhlGndVelDrvnRC_RadarHSC2','BrkPdlDrvrAppdPrsAlvRC_RadarHSC2','LDrvnWhlRotlDircnHSC2','RDrvnWhlRotlDircnHSC2','WhlGndVelLDrvnV_RadarHSC2','WhlGndVelRDrvnV_RadarHSC2','WhlBrkPrsStsHSC2','BrkDiscTemStsHSC2','BrkPdlDrvrAppdPrsV_RadarHSC2','','',''}},'OutputPortsLabelMode','ON','InputPortsWidth',int32(0),'InputPortsActive',0,'DialogFcn','rtican_message_interface_gui','BlockDisplay',{{'','center'}},'IconTransparency','on','ParameterTunableNames',{{}},'InitLevel',3,'BlockName',struct('Token',{{'SCS_HSC2_FrP22'}}),'SampleTime',{{-1}},'TriggerPort',{{'none'}},'EnablePort',{{'none'}})  RTIBlockParameters=struct('BoardTypeNo',{{1,'OFF',[]}},'BoardNo',{{1,'ON',[1 16]}},'ChannelNo',{{1,'ON',[1 2]}},'Parameters',{{struct('DataFileSupport',struct('DataFileSelectedMaster',1,'DataFileSelectedLocal',1,'DataFileName','c:\users\linqi\desktop\matlab\acc\dbc\ep21_dbc\171114-lh1-ep21_ep2_fdr-_v07.dbc|','DataFileDate',['24-11月-2020 15:06:17'],'SelectedFile','..\..\dbc\ep21_dbc\171114-lh1-ep21_ep2_fdr-_v07_acc.dbc','InterfaceFcn','rtican_dbc_file_parser'),'Options',struct('StatusSelected',1,'TimeSelected',1,'DeltaTimeSelected',1,'BytePortSelected',0,'MessageLengthSelected',0,'TriggerPort',struct('Selected',0,'TriggerType',0),'UserCoding',struct('Selected',0,'InterfaceFile','UserDecodingFile','FcnName','UserDecodeFcn','InportSelected',0,'InportWidth',1,'OutportSelected',0,'OutportWidth',1),'EnablePortSelected',0,'SignalOnPortnameSelected',1,'UseRXService',0),'Message',struct('MsgOnBlocknameSelected',1,'MsgName','SCS_HSC2_FrP22','MsgIdFormat',0,'MsgId',588,'MsgLength',8,'NumSignals',13,'SampleTime',-1,'Signal',struct('SgnName',{'WhlGndVelDrvnChksm_RadarHSC2','WhlGndVelLDrvn_RadarHSC2','WhlGndVelRDrvn_RadarHSC2','BrkPdlDrvrAppdPrs_RadarHSC2','WhlGndVelDrvnRC_RadarHSC2','BrkPdlDrvrAppdPrsAlvRC_RadarHSC2','LDrvnWhlRotlDircnHSC2','RDrvnWhlRotlDircnHSC2','WhlGndVelLDrvnV_RadarHSC2','WhlGndVelRDrvnV_RadarHSC2','WhlBrkPrsStsHSC2','BrkDiscTemStsHSC2','BrkPdlDrvrAppdPrsV_RadarHSC2'},'SgnStartBit',{0,8,24,40,48,52,54,57,59,60,61,62,63},'SgnLength',{8,14,14,8,4,2,2,2,1,1,1,1,1},'ByteLayout',{2,2,2,2,2,2,2,2,2,2,2,2,2},'Factor',{1,2^-5,2^-5,75,1,1,1,1,1,1,1,1,1},'Offset',{0,0,0,0,0,0,0,0,0,0,0,0,0},'SgnComment',{'','','','','','','','','','','','',''},'SgnUnit',{'','km/h','km/h','kPa','','','','','','','','',''},'Min',{0,0,0,0,0,0,0,0,0,0,0,0,0},'Max',{255,511.969,511.969,19125,15,3,3,3,1,1,1,1,1},'SgnType',{0,0,0,0,0,0,0,0,0,0,0,0,0},'SLDataType',{'SS_DOUBLE','SS_DOUBLE','SS_DOUBLE','SS_DOUBLE','SS_DOUBLE','SS_DOUBLE','SS_DOUBLE','SS_DOUBLE','SS_DOUBLE','SS_DOUBLE','SS_DOUBLE','SS_DOUBLE','SS_DOUBLE'},'DataType',{0,0,0,0,0,0,0,0,0,0,0,0,0},'ModeValue',{-1,-1,-1,-1,-1,-1,-1,-1,-1,-1,-1,-1,-1}),'MsgIdNumFormat',0,'MsgComment',{{''}}),'Version',1.2,'general',struct('isFromLib',0)),'OFF',[]}},'GroupId',{{struct('Group',{{'RTICAN'}},'No',1,'Behavior',{{'NAMECHANGE'}},'BlockType',{{'SINK'}},'NameChangeFlag',0),'OFF',[]}},'SFcnRTICANMessage',{{struct('MsgType','RX','SFcnPortType','Scalar','MsgName','SCS_HSC2_FrP22','MsgIdFormat','STD','MsgId',588,'MsgLength',8,'NumSignals',13,'SampleTime',-1,'Signal',struct('SgnName',{'WhlGndVelDrvnChksm_RadarHSC2','WhlGndVelLDrvn_RadarHSC2','WhlGndVelRDrvn_RadarHSC2','BrkPdlDrvrAppdPrs_RadarHSC2','WhlGndVelDrvnRC_RadarHSC2','BrkPdlDrvrAppdPrsAlvRC_RadarHSC2','LDrvnWhlRotlDircnHSC2','RDrvnWhlRotlDircnHSC2','WhlGndVelLDrvnV_RadarHSC2','WhlGndVelRDrvnV_RadarHSC2','WhlBrkPrsStsHSC2','BrkDiscTemStsHSC2','BrkPdlDrvrAppdPrsV_RadarHSC2'},'SgnStartBit',{0,8,24,40,48,52,54,57,59,60,61,62,63},'SgnLength',{8,14,14,8,4,2,2,2,1,1,1,1,1},'ByteLayout',{['motorola back.'],['motorola back.'],['motorola back.'],['motorola back.'],['motorola back.'],['motorola back.'],['motorola back.'],['motorola back.'],['motorola back.'],['motorola back.'],['motorola back.'],['motorola back.'],['motorola back.']},'Factor',{1,2^-5,2^-5,75,1,1,1,1,1,1,1,1,1},'Offset',{0,0,0,0,0,0,0,0,0,0,0,0,0},'SgnType',{'standard','standard','standard','standard','standard','standard','standard','standard','standard','standard','standard','standard','standard'},'SLDataType',{'SS_DOUBLE','SS_DOUBLE','SS_DOUBLE','SS_DOUBLE','SS_DOUBLE','SS_DOUBLE','SS_DOUBLE','SS_DOUBLE','SS_DOUBLE','SS_DOUBLE','SS_DOUBLE','SS_DOUBLE','SS_DOUBLE'},'DataType',{['unsigned int'],['unsigned int'],['unsigned int'],['unsigned int'],['unsigned int'],['unsigned int'],['unsigned int'],['unsigned int'],['unsigned int'],['unsigned int'],['unsigned int'],['unsigned int'],['unsigned int']},'ModeValue',{-1,-1,-1,-1,-1,-1,-1,-1,-1,-1,-1,-1,-1}),'StatusSelected','yes','TimeSelected','yes','DeltaTimeSelected','yes','BytePortSelected','no','MessageLengthSelected','no','TriggerPort',struct('Selected','no','TriggerType',0),'UserCoding',struct('Selected','no','InterfaceFile','UserDecodingFile','FcnName','UserDecodeFcn','InportSelected','no','InportWidth',1,'OutportSelected','no','OutportWidth',1),'EnablePortSelected','no','UseRXService','no','BoardType','DS1','BoardNo',1,'ControllerNo',1),'OFF',[]}},'TLCFileName',{{'rtican_rx_message','OFF',[]}})  RTISFcnParameters=struct('SFcnRTICANMessage','struct','TLCFileName','char')  RTIBlockParaDefault=struct('BoardTypeNo',4302,'BoardNo',1,'ChannelNo',1,'Parameters',struct('DataFileSupport',struct('DataFileSelectedMaster',0,'DataFileSelectedLocal',0,'DataFileName','','DataFileDate','','SelectedFile',['<no file selected>']),'Options',struct('StatusSelected',1,'TimeSelected',1,'DeltaTimeSelected',1,'BytePortSelected',0,'MessageLengthSelected',0,'TriggerPort',struct('Selected',0,'TriggerType','rising'),'UserCoding',struct('Selected',0,'InterfaceFile','UserDecodingFile','FcnName','UserDecodeFcn','InportSelected',0,'InportWidth',1,'OutportSelected',0,'OutportWidth',1),'EnablePortSelected',0,'SignalOnPortnameSelected',1,'UseRXService',0),'Message',struct('MsgOnBlocknameSelected',0,'MsgName',['RX Message'],'MsgIdFormat',0,'MsgId',100,'MsgLength',8,'NumSignals',1,'SampleTime',-1,'Signal',struct('SgnName',['RX signal'],'SgnStartBit',0,'SgnLength',8,'SgnType',0,'ModeValue',-1,'DataType',0,'SLDataType','SS_DOUBLE','ByteLayout',0,'Factor',1,'Offset',0,'Min',0,'Max',255,'SgnComment',{{}},'SgnUnit',''),'MsgIdNumFormat',0,'MsgComment',{{''}}),'Version',1.2,'general',struct('isFromLib',1)),'GroupId',struct('Group',{{'RTICAN'}},'No',1,'Behavior',{{'NAMECHANGE'}},'BlockType',{{'SINK'}},'NameChangeFlag',0),'SFcnRTICANMessage',struct('MsgType','RX','MsgName',['RX Message'],'MsgIdFormat','STD','MsgId',100,'MsgLength',8,'NumSignals',1,'SampleTime',-1,'Signal',struct('SgnName',['RX signal'],'SgnStartBit',0,'SgnLength',8,'SgnType','standard','ModeValue',-1,'DataType',['unsigned int'],'ByteLayout',['little endian'],'SLDataType','SS_DOUBLE','Factor',1,'Offset',0),'StatusSelected','yes','TimeSelected','yes','DeltaTimeSelected','yes','BytePortSelected','no','MessageLengthSelected','no','EnablePortSelected','no','UserCoding',struct('Selected','no','InterfaceFile','UserDecodingFile','FcnName','UserDecodeFcn','InportSelected','no','InportWidth',1,'OutportSelected','no','OutportWidth',1),'TriggerPort',struct('Selected','no','TriggerType','rising'),'UseRXService','no','BoardType','DS4302','BoardNo',1,'ControllerNo',1,'SFcnPortType','Scalar'),'TLCFileName','rtican_rx_message')
      settings: AttributesFormatString=Group Id: RTICAN1\n  SourceProductName=dSPACE RTI CAN Blockset
  SCS_HSC2_FrP23_0x24E : rtican/RTICAN Receive (RX)   Reserved1=[]  Reserved2=[]  Reserved3=[]  Reserved4=[]  SfcnMessage=[]  Msg_Struct=[]  BoardTypeNo=[]  BoardNo=[]  ChannelNo=[]  Parameters=[]  DialogFcn=[]  UnitName=[]  Revision=[]  UnitValues=[]  DSProperties=struct('RTI',struct('Version',uint32(5),'BlockType',struct('isSLSource',uint8(1),'isSLSink',uint8(1),'isHWSource',uint8(0),'isHWSink',uint8(0),'isSetup',uint8(0),'isInline',uint8(1),'isNonInline',uint8(0),'isInterrupt',uint8(0),'isChannelwise',uint8(0)),'IOBoardType','RTICAN','UnitType','MESSAGE','Identifier','RX','DialogType','MSVC','BlockSet','RTICAN','SlaveProcessor','CAN'))  RTIBlockInterface=struct('OutputPortsWidth',int32([1 1 1 1 1 1 1 1 1 1 1 1 1 1 1]),'OutputPortsActive',ones(1,15),'OutputPortsName',{{'WhlGndVelNonDrvnChksm_RadarHSC2','WhlGndVelLNonDrvn_RadarHSC2','WhlGndVelRNonDrvn_RadarHSC2','WhlGndVelLNonDrvnV_RadarHSC2','WhlGndVelRNonDrvnV_RadarHSC2','LNonDrvnWhlRotlDircn_RadarHSC2','TCSOpngMd_RadarHSC2','TCSOpngSts_RadarHSC2','RNonDrvnWhlRotlDircn_RadarHSC2','VSEMd_RadarHSC2','VSESts_RadarHSC2','WhlGndVelNonDrvnRC_RadarHSC2',['RX status'],['RX time'],['RX delta time']}},'OutputPortsDataType',{{'SS_DOUBLE','SS_DOUBLE','SS_DOUBLE','SS_DOUBLE','SS_DOUBLE','SS_DOUBLE','SS_DOUBLE','SS_DOUBLE','SS_DOUBLE','SS_DOUBLE','SS_DOUBLE','SS_DOUBLE','SS_DOUBLE','SS_DOUBLE','SS_DOUBLE'}},'OutputPortsLabel',{{'WhlGndVelNonDrvnChksm_RadarHSC2','WhlGndVelLNonDrvn_RadarHSC2','WhlGndVelRNonDrvn_RadarHSC2','WhlGndVelLNonDrvnV_RadarHSC2','WhlGndVelRNonDrvnV_RadarHSC2','LNonDrvnWhlRotlDircn_RadarHSC2','TCSOpngMd_RadarHSC2','TCSOpngSts_RadarHSC2','RNonDrvnWhlRotlDircn_RadarHSC2','VSEMd_RadarHSC2','VSESts_RadarHSC2','WhlGndVelNonDrvnRC_RadarHSC2','','',''}},'OutputPortsLabelMode','ON','InputPortsWidth',int32(0),'InputPortsActive',0,'DialogFcn','rtican_message_interface_gui','BlockDisplay',{{'','center'}},'IconTransparency','on','ParameterTunableNames',{{}},'InitLevel',3,'BlockName',struct('Token',{{'SCS_HSC2_FrP23'}}),'SampleTime',{{-1}},'TriggerPort',{{'none'}},'EnablePort',{{'none'}})  RTIBlockParameters=struct('BoardTypeNo',{{1,'OFF',[]}},'BoardNo',{{1,'ON',[1 16]}},'ChannelNo',{{1,'ON',[1 2]}},'Parameters',{{struct('DataFileSupport',struct('DataFileSelectedMaster',1,'DataFileSelectedLocal',1,'DataFileName','c:\users\linqi\desktop\matlab\acc\dbc\ep21_dbc\171114-lh1-ep21_ep2_fdr-_v07.dbc|','DataFileDate',['24-11月-2020 15:06:17'],'SelectedFile','..\..\dbc\ep21_dbc\171114-lh1-ep21_ep2_fdr-_v07_acc.dbc','InterfaceFcn','rtican_dbc_file_parser'),'Options',struct('StatusSelected',1,'TimeSelected',1,'DeltaTimeSelected',1,'BytePortSelected',0,'MessageLengthSelected',0,'TriggerPort',struct('Selected',0,'TriggerType',0),'UserCoding',struct('Selected',0,'InterfaceFile','UserDecodingFile','FcnName','UserDecodeFcn','InportSelected',0,'InportWidth',1,'OutportSelected',0,'OutportWidth',1),'EnablePortSelected',0,'SignalOnPortnameSelected',1,'UseRXService',0),'Message',struct('MsgOnBlocknameSelected',1,'MsgName','SCS_HSC2_FrP23','MsgIdFormat',0,'MsgId',590,'MsgLength',8,'NumSignals',12,'SampleTime',-1,'Signal',struct('SgnName',{'WhlGndVelNonDrvnChksm_RadarHSC2','WhlGndVelLNonDrvn_RadarHSC2','WhlGndVelRNonDrvn_RadarHSC2','WhlGndVelLNonDrvnV_RadarHSC2','WhlGndVelRNonDrvnV_RadarHSC2','LNonDrvnWhlRotlDircn_RadarHSC2','TCSOpngMd_RadarHSC2','TCSOpngSts_RadarHSC2','RNonDrvnWhlRotlDircn_RadarHSC2','VSEMd_RadarHSC2','VSESts_RadarHSC2','WhlGndVelNonDrvnRC_RadarHSC2'},'SgnStartBit',{0,8,24,38,39,40,42,45,48,50,53,60},'SgnLength',{8,14,14,1,1,2,3,3,2,3,3,4},'ByteLayout',{2,2,2,2,2,2,2,2,2,2,2,2},'Factor',{1,2^-5,2^-5,1,1,1,1,1,1,1,1,1},'Offset',{0,0,0,0,0,0,0,0,0,0,0,0},'SgnComment',{'','','','','','','','','','','',''},'SgnUnit',{'','km/h','km/h','','','','','','','','',''},'Min',{0,0,0,0,0,0,0,0,0,0,0,0},'Max',{255,511.969,511.969,1,1,3,7,7,3,7,7,15},'SgnType',{0,0,0,0,0,0,0,0,0,0,0,0},'SLDataType',{'SS_DOUBLE','SS_DOUBLE','SS_DOUBLE','SS_DOUBLE','SS_DOUBLE','SS_DOUBLE','SS_DOUBLE','SS_DOUBLE','SS_DOUBLE','SS_DOUBLE','SS_DOUBLE','SS_DOUBLE'},'DataType',{0,0,0,0,0,0,0,0,0,0,0,0},'ModeValue',{-1,-1,-1,-1,-1,-1,-1,-1,-1,-1,-1,-1}),'MsgIdNumFormat',0,'MsgComment',{{''}}),'Version',1.2,'general',struct('isFromLib',0)),'OFF',[]}},'GroupId',{{struct('Group',{{'RTICAN'}},'No',1,'Behavior',{{'NAMECHANGE'}},'BlockType',{{'SINK'}},'NameChangeFlag',0),'OFF',[]}},'SFcnRTICANMessage',{{struct('MsgType','RX','SFcnPortType','Scalar','MsgName','SCS_HSC2_FrP23','MsgIdFormat','STD','MsgId',590,'MsgLength',8,'NumSignals',12,'SampleTime',-1,'Signal',struct('SgnName',{'WhlGndVelNonDrvnChksm_RadarHSC2','WhlGndVelLNonDrvn_RadarHSC2','WhlGndVelRNonDrvn_RadarHSC2','WhlGndVelLNonDrvnV_RadarHSC2','WhlGndVelRNonDrvnV_RadarHSC2','LNonDrvnWhlRotlDircn_RadarHSC2','TCSOpngMd_RadarHSC2','TCSOpngSts_RadarHSC2','RNonDrvnWhlRotlDircn_RadarHSC2','VSEMd_RadarHSC2','VSESts_RadarHSC2','WhlGndVelNonDrvnRC_RadarHSC2'},'SgnStartBit',{0,8,24,38,39,40,42,45,48,50,53,60},'SgnLength',{8,14,14,1,1,2,3,3,2,3,3,4},'ByteLayout',{['motorola back.'],['motorola back.'],['motorola back.'],['motorola back.'],['motorola back.'],['motorola back.'],['motorola back.'],['motorola back.'],['motorola back.'],['motorola back.'],['motorola back.'],['motorola back.']},'Factor',{1,2^-5,2^-5,1,1,1,1,1,1,1,1,1},'Offset',{0,0,0,0,0,0,0,0,0,0,0,0},'SgnType',{'standard','standard','standard','standard','standard','standard','standard','standard','standard','standard','standard','standard'},'SLDataType',{'SS_DOUBLE','SS_DOUBLE','SS_DOUBLE','SS_DOUBLE','SS_DOUBLE','SS_DOUBLE','SS_DOUBLE','SS_DOUBLE','SS_DOUBLE','SS_DOUBLE','SS_DOUBLE','SS_DOUBLE'},'DataType',{['unsigned int'],['unsigned int'],['unsigned int'],['unsigned int'],['unsigned int'],['unsigned int'],['unsigned int'],['unsigned int'],['unsigned int'],['unsigned int'],['unsigned int'],['unsigned int']},'ModeValue',{-1,-1,-1,-1,-1,-1,-1,-1,-1,-1,-1,-1}),'StatusSelected','yes','TimeSelected','yes','DeltaTimeSelected','yes','BytePortSelected','no','MessageLengthSelected','no','TriggerPort',struct('Selected','no','TriggerType',0),'UserCoding',struct('Selected','no','InterfaceFile','UserDecodingFile','FcnName','UserDecodeFcn','InportSelected','no','InportWidth',1,'OutportSelected','no','OutportWidth',1),'EnablePortSelected','no','UseRXService','no','BoardType','DS1','BoardNo',1,'ControllerNo',1),'OFF',[]}},'TLCFileName',{{'rtican_rx_message','OFF',[]}})  RTISFcnParameters=struct('SFcnRTICANMessage','struct','TLCFileName','char')  RTIBlockParaDefault=struct('BoardTypeNo',4302,'BoardNo',1,'ChannelNo',1,'Parameters',struct('DataFileSupport',struct('DataFileSelectedMaster',0,'DataFileSelectedLocal',0,'DataFileName','','DataFileDate','','SelectedFile',['<no file selected>']),'Options',struct('StatusSelected',1,'TimeSelected',1,'DeltaTimeSelected',1,'BytePortSelected',0,'MessageLengthSelected',0,'TriggerPort',struct('Selected',0,'TriggerType','rising'),'UserCoding',struct('Selected',0,'InterfaceFile','UserDecodingFile','FcnName','UserDecodeFcn','InportSelected',0,'InportWidth',1,'OutportSelected',0,'OutportWidth',1),'EnablePortSelected',0,'SignalOnPortnameSelected',1,'UseRXService',0),'Message',struct('MsgOnBlocknameSelected',0,'MsgName',['RX Message'],'MsgIdFormat',0,'MsgId',100,'MsgLength',8,'NumSignals',1,'SampleTime',-1,'Signal',struct('SgnName',['RX signal'],'SgnStartBit',0,'SgnLength',8,'SgnType',0,'ModeValue',-1,'DataType',0,'SLDataType','SS_DOUBLE','ByteLayout',0,'Factor',1,'Offset',0,'Min',0,'Max',255,'SgnComment',{{}},'SgnUnit',''),'MsgIdNumFormat',0,'MsgComment',{{''}}),'Version',1.2,'general',struct('isFromLib',1)),'GroupId',struct('Group',{{'RTICAN'}},'No',1,'Behavior',{{'NAMECHANGE'}},'BlockType',{{'SINK'}},'NameChangeFlag',0),'SFcnRTICANMessage',struct('MsgType','RX','MsgName',['RX Message'],'MsgIdFormat','STD','MsgId',100,'MsgLength',8,'NumSignals',1,'SampleTime',-1,'Signal',struct('SgnName',['RX signal'],'SgnStartBit',0,'SgnLength',8,'SgnType','standard','ModeValue',-1,'DataType',['unsigned int'],'ByteLayout',['little endian'],'SLDataType','SS_DOUBLE','Factor',1,'Offset',0),'StatusSelected','yes','TimeSelected','yes','DeltaTimeSelected','yes','BytePortSelected','no','MessageLengthSelected','no','EnablePortSelected','no','UserCoding',struct('Selected','no','InterfaceFile','UserDecodingFile','FcnName','UserDecodeFcn','InportSelected','no','InportWidth',1,'OutportSelected','no','OutportWidth',1),'TriggerPort',struct('Selected','no','TriggerType','rising'),'UseRXService','no','BoardType','DS4302','BoardNo',1,'ControllerNo',1,'SFcnPortType','Scalar'),'TLCFileName','rtican_rx_message')
      settings: AttributesFormatString=Group Id: RTICAN1\n  SourceProductName=dSPACE RTI CAN Blockset
  SCS_HSC2_FrP24_0x251 : rtican/RTICAN Receive (RX)   Reserved1=[]  Reserved2=[]  Reserved3=[]  Reserved4=[]  SfcnMessage=[]  Msg_Struct=[]  BoardTypeNo=[]  BoardNo=[]  ChannelNo=[]  Parameters=[]  DialogFcn=[]  UnitName=[]  Revision=[]  UnitValues=[]  DSProperties=struct('RTI',struct('Version',uint32(5),'BlockType',struct('isSLSource',uint8(1),'isSLSink',uint8(1),'isHWSource',uint8(0),'isHWSink',uint8(0),'isSetup',uint8(0),'isInline',uint8(1),'isNonInline',uint8(0),'isInterrupt',uint8(0),'isChannelwise',uint8(0)),'IOBoardType','RTICAN','UnitType','MESSAGE','Identifier','RX','DialogType','MSVC','BlockSet','RTICAN','SlaveProcessor','CAN'))  RTIBlockInterface=struct('OutputPortsWidth',int32([1 1 1 1 1 1 1 1 1 1 1 1 1]),'OutputPortsActive',ones(1,13),'OutputPortsName',{{'ChACCAEBChksm_RadarHSC2','VehTrgtLongtAccHSC2','ChACCAEBAlvRlngCtr_RadarHSC2','ChAEBDclReqRespHSC2','ChACCAEBBrkJerkReqRespHSC2','ChAEBPrflReqRespHSC2','ChACCReqFlrStsHSC2','ChAEBHydBrkAstReqRespHSC2','ChACCAccReqRespHSC2','VehSdslStsHSC2',['RX status'],['RX time'],['RX delta time']}},'OutputPortsDataType',{{'SS_DOUBLE','SS_DOUBLE','SS_DOUBLE','SS_DOUBLE','SS_DOUBLE','SS_DOUBLE','SS_DOUBLE','SS_DOUBLE','SS_DOUBLE','SS_DOUBLE','SS_DOUBLE','SS_DOUBLE','SS_DOUBLE'}},'OutputPortsLabel',{{'ChACCAEBChksm_RadarHSC2','VehTrgtLongtAccHSC2','ChACCAEBAlvRlngCtr_RadarHSC2','ChAEBDclReqRespHSC2','ChACCAEBBrkJerkReqRespHSC2','ChAEBPrflReqRespHSC2','ChACCReqFlrStsHSC2','ChAEBHydBrkAstReqRespHSC2','ChACCAccReqRespHSC2','VehSdslStsHSC2','','',''}},'OutputPortsLabelMode','ON','InputPortsWidth',int32(0),'InputPortsActive',0,'DialogFcn','rtican_message_interface_gui','BlockDisplay',{{'','center'}},'IconTransparency','on','ParameterTunableNames',{{}},'InitLevel',3,'BlockName',struct('Token',{{'SCS_HSC2_FrP24'}}),'SampleTime',{{-1}},'TriggerPort',{{'none'}},'EnablePort',{{'none'}})  RTIBlockParameters=struct('BoardTypeNo',{{1,'OFF',[]}},'BoardNo',{{1,'ON',[1 16]}},'ChannelNo',{{1,'ON',[1 2]}},'Parameters',{{struct('DataFileSupport',struct('DataFileSelectedMaster',1,'DataFileSelectedLocal',1,'DataFileName','c:\users\administrator.zx-201607042142\desktop\zone\2020_demo\ep21原车dbc\171114-lh1-ep21_ep2_fdr-_v07_acc.dbc|c:\users\administrator.zx-201607042142\documents\matlab\zone\dbc\ep21_dbc\171120-lh1-ep21_ep2_fvcm-_v07_lka.dbc|','DataFileDate',{{{['30-十一月-2020 14:32:34']},{''}}},'SelectedFile','c:\users\linqi\desktop\matlab\acc\dbc\ep21_dbc\171114-lh1-ep21_ep2_fdr-_v07_acc.dbc','InterfaceFcn','rtican_dbc_file_parser'),'Options',struct('StatusSelected',1,'TimeSelected',1,'DeltaTimeSelected',1,'BytePortSelected',0,'MessageLengthSelected',0,'TriggerPort',struct('Selected',0,'TriggerType',0),'UserCoding',struct('Selected',0,'InterfaceFile','UserDecodingFile','FcnName','UserDecodeFcn','InportSelected',0,'InportWidth',1,'OutportSelected',0,'OutportWidth',1),'EnablePortSelected',0,'SignalOnPortnameSelected',1,'UseRXService',0),'Message',struct('MsgOnBlocknameSelected',1,'MsgName','SCS_HSC2_FrP24','MsgIdFormat',0,'MsgId',593,'MsgLength',8,'NumSignals',10,'SampleTime',-1,'Signal',struct('SgnName',{'ChACCAEBChksm_RadarHSC2','VehTrgtLongtAccHSC2','ChACCAEBAlvRlngCtr_RadarHSC2','ChAEBDclReqRespHSC2','ChACCAEBBrkJerkReqRespHSC2','ChAEBPrflReqRespHSC2','ChACCReqFlrStsHSC2','ChAEBHydBrkAstReqRespHSC2','ChACCAccReqRespHSC2','VehSdslStsHSC2'},'SgnStartBit',{0,32,41,45,48,51,54,56,59,62},'SgnLength',{8,8,4,3,3,3,2,3,3,2},'SgnType',{0,0,0,0,0,0,0,0,0,0},'ModeValue',{-1,-1,-1,-1,-1,-1,-1,-1,-1,-1},'DataType',{0,0,0,0,0,0,0,0,0,0},'ByteLayout',{2,2,2,2,2,2,2,2,2,2},'Factor',{1,0.05,1,1,1,1,1,1,1,1},'Offset',{0,-7,0,0,0,0,0,0,0,0},'SgnComment',{{''},{''},{''},{['2017.05.25' char(10) 'ChACCAEBDclReqResp_Radar name changed to ChAEBDclReqResp']},{''},{['2017.05.25:' char(10) 'ChACCAEBPrflReqResp name changed to ChAEBPrflReqResp' char(10) '' char(10) ',and encode updated' char(10) '' char(10) 'ChAEBPrflReqResp' char(10) '' char(10) '']},{''},{['2017.05.25:' char(10) 'ChACCAEBHydBrkAstReqResp name changed to ChAEBHydBrkAstReqResp']},{['2017.05.25' char(10) 'ChACCAEBAccReqResp name changed to ChACCAccReqResp']},{''}},'SgnUnit',{'','','','','','','','','',''},'Min',{0,-7,0,0,0,0,0,0,0,0},'Max',{255,5.75,15,7,7,7,3,7,7,3},'SLDataType',{'SS_DOUBLE','SS_DOUBLE','SS_DOUBLE','SS_DOUBLE','SS_DOUBLE','SS_DOUBLE','SS_DOUBLE','SS_DOUBLE','SS_DOUBLE','SS_DOUBLE'}),'MsgIdNumFormat',1,'MsgComment',{{''}}),'Version',1.2,'general',struct('isFromLib',0)),'OFF',[]}},'GroupId',{{struct('Group',{{'RTICAN'}},'No',1,'Behavior',{{'NAMECHANGE'}},'BlockType',{{'SINK'}},'NameChangeFlag',0),'OFF',[]}},'SFcnRTICANMessage',{{struct('MsgType','RX','SFcnPortType','Scalar','MsgName','SCS_HSC2_FrP24','MsgIdFormat','STD','MsgId',593,'MsgLength',8,'NumSignals',10,'SampleTime',-1,'Signal',struct('SgnName',{'ChACCAEBChksm_RadarHSC2','VehTrgtLongtAccHSC2','ChACCAEBAlvRlngCtr_RadarHSC2','ChAEBDclReqRespHSC2','ChACCAEBBrkJerkReqRespHSC2','ChAEBPrflReqRespHSC2','ChACCReqFlrStsHSC2','ChAEBHydBrkAstReqRespHSC2','ChACCAccReqRespHSC2','VehSdslStsHSC2'},'SgnStartBit',{0,32,41,45,48,51,54,56,59,62},'SgnLength',{8,8,4,3,3,3,2,3,3,2},'SgnType',{'standard','standard','standard','standard','standard','standard','standard','standard','standard','standard'},'ModeValue',{-1,-1,-1,-1,-1,-1,-1,-1,-1,-1},'DataType',{['unsigned int'],['unsigned int'],['unsigned int'],['unsigned int'],['unsigned int'],['unsigned int'],['unsigned int'],['unsigned int'],['unsigned int'],['unsigned int']},'ByteLayout',{['motorola back.'],['motorola back.'],['motorola back.'],['motorola back.'],['motorola back.'],['motorola back.'],['motorola back.'],['motorola back.'],['motorola back.'],['motorola back.']},'Factor',{1,0.05,1,1,1,1,1,1,1,1},'Offset',{0,-7,0,0,0,0,0,0,0,0},'SLDataType',{'SS_DOUBLE','SS_DOUBLE','SS_DOUBLE','SS_DOUBLE','SS_DOUBLE','SS_DOUBLE','SS_DOUBLE','SS_DOUBLE','SS_DOUBLE','SS_DOUBLE'}),'StatusSelected','yes','TimeSelected','yes','DeltaTimeSelected','yes','BytePortSelected','no','MessageLengthSelected','no','TriggerPort',struct('Selected','no','TriggerType',0),'UserCoding',struct('Selected','no','InterfaceFile','UserDecodingFile','FcnName','UserDecodeFcn','InportSelected','no','InportWidth',1,'OutportSelected','no','OutportWidth',1),'EnablePortSelected','no','UseRXService','no','BoardType','DS1','BoardNo',1,'ControllerNo',1),'OFF',[]}},'TLCFileName',{{'rtican_rx_message','OFF',[]}})  RTISFcnParameters=struct('SFcnRTICANMessage','struct','TLCFileName','char')  RTIBlockParaDefault=struct('BoardTypeNo',4302,'BoardNo',1,'ChannelNo',1,'Parameters',struct('DataFileSupport',struct('DataFileSelectedMaster',0,'DataFileSelectedLocal',0,'DataFileName','','DataFileDate','','SelectedFile',['<no file selected>']),'Options',struct('StatusSelected',1,'TimeSelected',1,'DeltaTimeSelected',1,'BytePortSelected',0,'MessageLengthSelected',0,'TriggerPort',struct('Selected',0,'TriggerType','rising'),'UserCoding',struct('Selected',0,'InterfaceFile','UserDecodingFile','FcnName','UserDecodeFcn','InportSelected',0,'InportWidth',1,'OutportSelected',0,'OutportWidth',1),'EnablePortSelected',0,'SignalOnPortnameSelected',1,'UseRXService',0),'Message',struct('MsgOnBlocknameSelected',0,'MsgName',['RX Message'],'MsgIdFormat',0,'MsgId',100,'MsgLength',8,'NumSignals',1,'SampleTime',-1,'Signal',struct('SgnName',['RX signal'],'SgnStartBit',0,'SgnLength',8,'SgnType',0,'ModeValue',-1,'DataType',0,'SLDataType','SS_DOUBLE','ByteLayout',0,'Factor',1,'Offset',0,'Min',0,'Max',255,'SgnComment',{{}},'SgnUnit',''),'MsgIdNumFormat',0,'MsgComment',{{''}}),'Version',1.2,'general',struct('isFromLib',1)),'GroupId',struct('Group',{{'RTICAN'}},'No',1,'Behavior',{{'NAMECHANGE'}},'BlockType',{{'SINK'}},'NameChangeFlag',0),'SFcnRTICANMessage',struct('MsgType','RX','MsgName',['RX Message'],'MsgIdFormat','STD','MsgId',100,'MsgLength',8,'NumSignals',1,'SampleTime',-1,'Signal',struct('SgnName',['RX signal'],'SgnStartBit',0,'SgnLength',8,'SgnType','standard','ModeValue',-1,'DataType',['unsigned int'],'ByteLayout',['little endian'],'SLDataType','SS_DOUBLE','Factor',1,'Offset',0),'StatusSelected','yes','TimeSelected','yes','DeltaTimeSelected','yes','BytePortSelected','no','MessageLengthSelected','no','EnablePortSelected','no','UserCoding',struct('Selected','no','InterfaceFile','UserDecodingFile','FcnName','UserDecodeFcn','InportSelected','no','InportWidth',1,'OutportSelected','no','OutportWidth',1),'TriggerPort',struct('Selected','no','TriggerType','rising'),'UseRXService','no','BoardType','DS4302','BoardNo',1,'ControllerNo',1,'SFcnPortType','Scalar'),'TLCFileName','rtican_rx_message')
      settings: AttributesFormatString=Group Id: RTICAN1\n  SourceProductName=dSPACE RTI CAN Blockset
  COM_VehBus_st : Outport  OutDataTypeStr=Bus: COM_VEHBUS_ST  BusOutputAsStruct=on
  wires:
  Data Type Conversion55/1 -> Bus Creator10/5
  Data Type Conversion57/1 -> Bus Creator11/2
  GW_HSC2_HCU_FrP08_0xAC/4 -> Data Type Conversion57/1  "EPTTrInptShaftMinAvlblToqHSC2"
  Data Type Conversion3/1 -> Bus Creator2/4
  SCS_HSC2_FrP22_0x24C/9 -> Data Type Conversion36/1  "WhlGndVelLDrvnV_RadarHSC2"
  Data Type Conversion46/1 -> Bus Creator8/6
  Data Type Conversion21/1 -> Bus Creator/1
  GW_HSC2_HCU_FrP08_0xAC/6 -> Data Type Conversion59/1  "EPTTrInptShaftMinAvlblToqVHSC2"
  SCS_HSC2_FrP23_0x24E/6 -> Data Type Conversion45/1  "LNonDrvnWhlRotlDircn_RadarHSC2"
  GW_HSC2_HCU_FrP08_0xAC/5 -> Data Type Conversion58/1  "EPTTrInptShaftMaxAvlblToqVHSC2"
  GW_HSC2_HCU_FrP00_0xAF/5 -> Data Type Conversion53/1  "EPTBrkPdlDscrtInptStsVHSC2"
  GW_HSC2_HCU_FrP08_0xAC/2 -> Data Type Conversion56/1  "EPTTrInptShaftMaxAvlblToqHSC2"
  SCS_HSC2_FrP22_0x24C/2 -> Data Type Conversion31/1  "WhlGndVelLDrvn_RadarHSC2"
  Data Type Conversion59/1 -> Bus Creator11/4
  Bus Creator4/1 -> Bus Creator9/5
  GW_HSC2_HCU_FrP00_0xAF/8 -> Data Type Conversion55/1  "EPTAccelActuPosHSC2"
  Data Type Conversion14/1 -> Bus Creator3/7
  Data Type Conversion45/1 -> Bus Creator8/5
  SCS_HSC2_FrP22_0x24C/10 -> Data Type Conversion37/1  "WhlGndVelRDrvnV_RadarHSC2"
  SCS_HSC2_FrP05_0x1E9/4 -> Data Type Conversion19/1  "ABSAHSC2"
  Data Type Conversion54/1 -> Bus Creator10/4
  Data Type Conversion22/1 -> Bus Creator/3
  SCS_HSC2_FrP19_0x23C/2 -> Data Type Conversion30/1  "VehSpdAvgHSC2"
  GW_HSC2_HCU_FrP00_0xAF/6 -> Data Type Conversion54/1  "EPTStCmdOn_h1HSC2"
  Bus Creator5/1 -> Bus Creator9/6
  Data Type Conversion58/1 -> Bus Creator11/3
  Data Type Conversion47/1 -> Bus Creator8/7
  Data Type Conversion36/1 -> Bus Creator7/6
  Data Type Conversion53/1 -> Bus Creator10/3
  Data Type Conversion33/1 -> Bus Creator7/3
  Bus Creator2/1 -> Bus Creator9/3
  Data Type Conversion56/1 -> Bus Creator11/1
  Data Type Conversion29/1 -> Bus Creator5/1
  GW_HSC2_FrP04_0x1E1/7 -> Data Type Conversion3/1  "CCSwStsSpdIncSwA_h2HSC2"
  SCS_HSC2_FrP02_0x185/3 -> Data Type Conversion15/1  "VSELongtAccVHSC2"
  Bus Creator7/1 -> Bus Creator9/8
  Data Type Conversion24/1 -> Bus Creator3/1
  Bus Creator9/1 -> COM_VehBus_st/1  "COM_VehBus_st"
  Bus Creator8/1 -> Bus Creator9/9
  Bus Creator1/1 -> Bus Creator9/2
  Bus Creator3/1 -> Bus Creator9/4
  Data Type Conversion52/1 -> Bus Creator10/2
  Bus Creator6/1 -> Bus Creator9/7
  Data Type Conversion51/1 -> Bus Creator10/1
  SCS_HSC2_FrP23_0x24E/7 -> Data Type Conversion46/1  "TCSOpngMd_RadarHSC2"
  SCS_HSC2_FrP23_0x24E/5 -> Data Type Conversion44/1  "WhlGndVelRNonDrvnV_RadarHSC2"
  Data Type Conversion49/1 -> Bus Creator8/9
  Data Type Conversion43/1 -> Bus Creator8/3
  SCS_HSC2_FrP23_0x24E/4 -> Data Type Conversion43/1  "WhlGndVelLNonDrvnV_RadarHSC2"
  Data Type Conversion50/1 -> Bus Creator8/10
  SCS_HSC2_FrP23_0x24E/9 -> Data Type Conversion48/1  "RNonDrvnWhlRotlDircn_RadarHSC2"
  SCS_HSC2_FrP23_0x24E/11 -> Data Type Conversion50/1  "VSESts_RadarHSC2"
  SCS_HSC2_FrP22_0x24C/12 -> Data Type Conversion39/1  "BrkDiscTemStsHSC2"
  SCS_HSC2_FrP23_0x24E/10 -> Data Type Conversion49/1  "VSEMd_RadarHSC2"
  Data Type Conversion42/1 -> Bus Creator8/2
  SCS_HSC2_FrP05_0x1E9/3 -> Data Type Conversion18/1  "EnDragToqRducnAHSC2"
  Data Type Conversion30/1 -> Bus Creator6/1
  SCS_HSC2_FrP23_0x24E/2 -> Data Type Conversion41/1  "WhlGndVelLNonDrvn_RadarHSC2"
  Data Type Conversion40/1 -> Bus Creator7/10
  SCS_HSC2_FrP22_0x24C/11 -> Data Type Conversion38/1  "WhlBrkPrsStsHSC2"
  SCS_HSC2_FrP23_0x24E/3 -> Data Type Conversion42/1  "WhlGndVelRNonDrvn_RadarHSC2"
  Data Type Conversion34/1 -> Bus Creator7/4
  SCS_HSC2_FrP22_0x24C/3 -> Data Type Conversion32/1  "WhlGndVelRDrvn_RadarHSC2"
  Data Type Conversion41/1 -> Bus Creator8/1
  Data Type Conversion44/1 -> Bus Creator8/4
  Data Type Conversion39/1 -> Bus Creator7/9
  Data Type Conversion23/1 -> Bus Creator1/2
  Data Type Conversion32/1 -> Bus Creator7/2
  Data Type Conversion26/1 -> Bus Creator3/6
  Bus Creator11/1 -> Bus Creator9/11
  GW_HSC2_ECM_FrP27_0xFB/4 -> Data Type Conversion23/1  "PtACCToqReqRespHSC2"
  Data Type Conversion25/1 -> Bus Creator3/2
  GW_HSC2_FrP04_0x1E1/9 -> Data Type Conversion5/1  "CCSwStsRsmSwA_h2HSC2"
  Data Type Conversion27/1 -> Bus Creator4/1
  SCS_HSC2_FrP22_0x24C/4 -> Data Type Conversion33/1  "BrkPdlDrvrAppdPrs_RadarHSC2"
  Data Type Conversion48/1 -> Bus Creator8/8
  Data Type Conversion2/1 -> Bus Creator2/3
  SCS_HSC2_FrP05_0x1E9/1 -> Data Type Conversion29/1  "VehDynYawRateHSC2"
  Data Type Conversion12/1 -> Bus Creator3/4
  Data Type Conversion10/1 -> Bus Creator1/1
  GW_HSC2_FrP04_0x1E1/6 -> Data Type Conversion2/1  "CCSwStsSpdDecSwA_h2HSC2"
  Data Type Conversion7/1 -> Bus Creator2/8
  SCS_HSC2_FrP22_0x24C/13 -> Data Type Conversion40/1  "BrkPdlDrvrAppdPrsV_RadarHSC2"
  Data Type Conversion13/1 -> Bus Creator3/5
  GW_HSC2_HCU_FrP00_0xAF/4 -> Data Type Conversion52/1  "EPTBrkPdlDscrtInptStsHSC2"
  SCS_HSC2_FrP02_0x185/1 -> Data Type Conversion27/1  "VSELatAccHSC2"
  Data Type Conversion18/1 -> Bus Creator5/3
  Data Type Conversion37/1 -> Bus Creator7/7
  Data Type Conversion19/1 -> Bus Creator5/4
  SCS_HSC2_FrP23_0x24E/8 -> Data Type Conversion47/1  "TCSOpngSts_RadarHSC2"
  Data Type Conversion35/1 -> Bus Creator7/5
  Data Type Conversion15/1 -> Bus Creator4/3
  Data Type Conversion11/1 -> Bus Creator3/3
  Data Type Conversion16/1 -> Bus Creator4/4
  Data Type Conversion4/1 -> Bus Creator2/5
  SCS_HSC2_FrP05_0x1E9/2 -> Data Type Conversion17/1  "VehDynYawRateVHSC2"
  GW_HSC2_FrP04_0x1E1/10 -> Data Type Conversion6/1  "CCSwStsOnSwA_h2HSC2"
  SCS_HSC2_FrP19_0x23C/3 -> Data Type Conversion20/1  "VehSpdAvgVHSC2"
  GW_HSC2_ECM_FrP27_0xFB/3 -> Data Type Conversion10/1  "AccelOvrdHSC2"
  Data Type Conversion5/1 -> Bus Creator2/6
  GW_HSC2_FrP04_0x1E1/11 -> Data Type Conversion7/1  "CCSwStsCanclSwA_h2HSC2"
  Data Type Conversion8/1 -> Bus Creator/2
  Bus Creator/1 -> Bus Creator9/1
  GW_HSC2_FrP04_0x1E1/3 -> Data Type Conversion1/1  "CCSwStsDistIncSwA_h2HSC2"
  Data Type Conversion20/1 -> Bus Creator6/2
  SCS_HSC2_FrP02_0x185/2 -> Data Type Conversion28/1  "VSELongtAccHSC2"
  Data Type Conversion9/1 -> Bus Creator/4
  SCS_HSC2_FrP02_0x185/4 -> Data Type Conversion16/1  "VSELatAccVHSC2"
  Data Type Conversion/1 -> Bus Creator2/1
  Data Type Conversion31/1 -> Bus Creator7/1
  Data Type Conversion17/1 -> Bus Creator5/2
  GW_HSC2_ECM_FrP04_0x194/4 -> Data Type Conversion9/1  "TrEstdGearVHSC2"
  Data Type Conversion1/1 -> Bus Creator2/2
  GW_HSC2_HCU_FrP00_0xAF/2 -> Data Type Conversion51/1  "EPTAccelActuPosVHSC2"
  GW_HSC2_ECM_FrP04_0x194/3 -> Data Type Conversion22/1  "TrEstdGearHSC2"
  Data Type Conversion38/1 -> Bus Creator7/8
  Data Type Conversion6/1 -> Bus Creator2/7
  GW_HSC2_FrP04_0x1E1/8 -> Data Type Conversion4/1  "CCSwStsSetSwA_h2HSC2"
  GW_HSC2_FrP04_0x1E1/2 -> Data Type Conversion/1  "CCSwStsDistDecSwA_h2HSC2"
  SCS_HSC2_FrP22_0x24C/7 -> Data Type Conversion34/1  "LDrvnWhlRotlDircnHSC2"
  GW_HSC2_ECM_FrP04_0x194/1 -> Data Type Conversion21/1  "TrShftLvrPos_h1HSC2"
  SCS_HSC2_FrP22_0x24C/8 -> Data Type Conversion35/1  "RDrvnWhlRotlDircnHSC2"
  Bus Creator10/1 -> Bus Creator9/10
  GW_HSC2_ECM_FrP04_0x194/2 -> Data Type Conversion8/1  "TrShftLvrPosV_h1HSC2"
  Data Type Conversion28/1 -> Bus Creator4/2
  EHBS_HSC2_FrP00_0x1B6/3 -> Data Type Conversion60/1  "BrkPdlAppdVHSC2"
  EHBS_HSC2_FrP00_0x1B6/4 -> Data Type Conversion61/1  "BrkPdlAppdHSC2"
  Bus Creator12/1 -> Bus Creator9/12
  Data Type Conversion60/1 -> Bus Creator12/1
  Data Type Conversion61/1 -> Bus Creator12/2
  GW_HSC2_FICM_FrP02_0x376/2 -> Data Type Conversion63/1  "LDWLKASwReqHSC2"
  Data Type Conversion62/1 -> Bus Creator13/1
  Data Type Conversion63/1 -> Bus Creator14/1
  Bus Creator14/1 -> Bus Creator9/14
  Bus Creator13/1 -> Bus Creator9/13
  Data Type Conversion64/1 -> Bus Creator15/1
  Data Type Conversion65/1 -> Bus Creator15/2
  Data Type Conversion66/1 -> Bus Creator15/3
  Data Type Conversion67/1 -> Bus Creator15/4
  Data Type Conversion68/1 -> Bus Creator15/5
  Bus Creator15/1 -> Bus Creator9/15
  EPS_HSC2_FrP03_0x1EC/1 -> Data Type Conversion64/1  "ChLKACtrlStsHSC2"
  EPS_HSC2_FrP03_0x1EC/2 -> Data Type Conversion65/1  "DrvrStrgDlvrdToqVHSC2"
  EPS_HSC2_FrP03_0x1EC/3 -> Data Type Conversion66/1  "DrvrStrgDlvrdToqHSC2"
  EPS_HSC2_FrP03_0x1EC/5 -> Data Type Conversion67/1  "ChLKARespToqHSC2"
  EPS_HSC2_FrP03_0x1EC/6 -> Data Type Conversion68/1  "ChLKARespToqVHSC2"
  SCS_HSC2_FrP24_0x251/2 -> Data Type Conversion69/1  "VehTrgtLongtAccHSC2"
  Data Type Conversion69/1 -> Bus Creator16/1
  Data Type Conversion70/1 -> Bus Creator16/2
  SCS_HSC2_FrP24_0x251/4 -> Data Type Conversion70/1  "ChAEBDclReqRespHSC2"
  Data Type Conversion71/1 -> Bus Creator16/3
